simulink model "simulator_prototype"  (R2021b)
(part 11 of 12)

t6722 = ct{1511};
t6724 = ct{1512};
t6725 = ct{1513};
t6727 = ct{1514};
t6728 = ct{1515};
t6731 = ct{1516};
t6732 = ct{1517};
t6736 = ct{1518};
t6737 = ct{1519};
t6738 = ct{1520};
t6739 = ct{1521};
t674 = ct{1522};
t6740 = ct{1523};
t6742 = ct{1524};
t6743 = ct{1525};
t6744 = ct{1526};
t6745 = ct{1527};
t6746 = ct{1528};
t6747 = ct{1529};
t6750 = ct{1530};
t6751 = ct{1531};
t6754 = ct{1532};
t6756 = ct{1533};
t6757 = ct{1534};
t6758 = ct{1535};
t6760 = ct{1536};
t6762 = ct{1537};
t6763 = ct{1538};
t6764 = ct{1539};
t6765 = ct{1540};
t6766 = ct{1541};
t6767 = ct{1542};
t6768 = ct{1543};
t6769 = ct{1544};
t6770 = ct{1545};
t6771 = ct{1546};
t6772 = ct{1547};
t6773 = ct{1548};
t6774 = ct{1549};
t6775 = ct{1550};
t6776 = ct{1551};
t6778 = ct{1552};
t6779 = ct{1553};
t6780 = ct{1554};
t6781 = ct{1555};
t6782 = ct{1556};
t6783 = ct{1557};
t6784 = ct{1558};
t6785 = ct{1559};
t6786 = ct{1560};
t6787 = ct{1561};
t6788 = ct{1562};
t6789 = ct{1563};
t6791 = ct{1564};
t6792 = ct{1565};
t6793 = ct{1566};
t6795 = ct{1567};
t6796 = ct{1568};
t6797 = ct{1569};
t6798 = ct{1570};
t6799 = ct{1571};
t6800 = ct{1572};
t6803 = ct{1573};
t6804 = ct{1574};
t6808 = ct{1575};
t6810 = ct{1576};
t6813 = ct{1577};
t6814 = ct{1578};
t6816 = ct{1579};
t6817 = ct{1580};
t6819 = ct{1581};
t6820 = ct{1582};
t6821 = ct{1583};
t6822 = ct{1584};
t6823 = ct{1585};
t6824 = ct{1586};
t6825 = ct{1587};
t6826 = ct{1588};
t6827 = ct{1589};
t6828 = ct{1590};
t6831 = ct{1591};
t6833 = ct{1592};
t6836 = ct{1593};
t6838 = ct{1594};
t6839 = ct{1595};
t684 = ct{1596};
t6841 = ct{1597};
t6842 = ct{1598};
t6843 = ct{1599};
t6844 = ct{1600};
t6848 = ct{1601};
t6849 = ct{1602};
t685 = ct{1603};
t6851 = ct{1604};
t6852 = ct{1605};
t6853 = ct{1606};
t6855 = ct{1607};
t6858 = ct{1608};
t6859 = ct{1609};
t686 = ct{1610};
t6866 = ct{1611};
t6867 = ct{1612};
t6868 = ct{1613};
t687 = ct{1614};
t6870 = ct{1615};
t6872 = ct{1616};
t6873 = ct{1617};
t6875 = ct{1618};
t6877 = ct{1619};
t6878 = ct{1620};
t6879 = ct{1621};
t6880 = ct{1622};
t6882 = ct{1623};
t6883 = ct{1624};
t6884 = ct{1625};
t6885 = ct{1626};
t6886 = ct{1627};
t6887 = ct{1628};
t6888 = ct{1629};
t6889 = ct{1630};
t6894 = ct{1631};
t6897 = ct{1632};
t6900 = ct{1633};
t6902 = ct{1634};
t6903 = ct{1635};
t6904 = ct{1636};
t6908 = ct{1637};
t6909 = ct{1638};
t6910 = ct{1639};
t6911 = ct{1640};
t6912 = ct{1641};
t6913 = ct{1642};
t6916 = ct{1643};
t6918 = ct{1644};
t6919 = ct{1645};
t6920 = ct{1646};
t6924 = ct{1647};
t6925 = ct{1648};
t6929 = ct{1649};
t6931 = ct{1650};
t6932 = ct{1651};
t6933 = ct{1652};
t6941 = ct{1653};
t6942 = ct{1654};
t6945 = ct{1655};
t6949 = ct{1656};
t6950 = ct{1657};
t6951 = ct{1658};
t6959 = ct{1659};
t6962 = ct{1660};
t6964 = ct{1661};
t6965 = ct{1662};
t6966 = ct{1663};
t6968 = ct{1664};
t6971 = ct{1665};
t6972 = ct{1666};
t6975 = ct{1667};
t6976 = ct{1668};
t6979 = ct{1669};
t6983 = ct{1670};
t6985 = ct{1671};
t6987 = ct{1672};
t6989 = ct{1673};
t6992 = ct{1674};
t6993 = ct{1675};
t6994 = ct{1676};
t6995 = ct{1677};
t6996 = ct{1678};
t6997 = ct{1679};
t7000 = ct{1680};
t7001 = ct{1681};
t7003 = ct{1682};
t7005 = ct{1683};
t7007 = ct{1684};
t7009 = ct{1685};
t7010 = ct{1686};
t7011 = ct{1687};
t7012 = ct{1688};
t7014 = ct{1689};
t7016 = ct{1690};
t7019 = ct{1691};
t7020 = ct{1692};
t7022 = ct{1693};
t7023 = ct{1694};
t7024 = ct{1695};
t7025 = ct{1696};
t7026 = ct{1697};
t7028 = ct{1698};
t7029 = ct{1699};
t7030 = ct{1700};
t7031 = ct{1701};
t7032 = ct{1702};
t7033 = ct{1703};
t7034 = ct{1704};
t7035 = ct{1705};
t7036 = ct{1706};
t7037 = ct{1707};
t7038 = ct{1708};
t7039 = ct{1709};
t7040 = ct{1710};
t7041 = ct{1711};
t7042 = ct{1712};
t7043 = ct{1713};
t7047 = ct{1714};
t7048 = ct{1715};
t7049 = ct{1716};
t7051 = ct{1717};
t7052 = ct{1718};
t7055 = ct{1719};
t7057 = ct{1720};
t7059 = ct{1721};
t7060 = ct{1722};
t7061 = ct{1723};
t7062 = ct{1724};
t7063 = ct{1725};
t7064 = ct{1726};
t7066 = ct{1727};
t707 = ct{1728};
t7072 = ct{1729};
t7073 = ct{1730};
t7074 = ct{1731};
t7076 = ct{1732};
t7078 = ct{1733};
t7079 = ct{1734};
t708 = ct{1735};
t7080 = ct{1736};
t7083 = ct{1737};
t7084 = ct{1738};
t7086 = ct{1739};
t7088 = ct{1740};
t7090 = ct{1741};
t7092 = ct{1742};
t7095 = ct{1743};
t7098 = ct{1744};
t710 = ct{1745};
t7101 = ct{1746};
t7102 = ct{1747};
t7108 = ct{1748};
t7109 = ct{1749};
t7111 = ct{1750};
t7112 = ct{1751};
t7114 = ct{1752};
t7118 = ct{1753};
t7125 = ct{1754};
t7127 = ct{1755};
t7128 = ct{1756};
t7131 = ct{1757};
t7132 = ct{1758};
t7133 = ct{1759};
t7134 = ct{1760};
t7140 = ct{1761};
t7142 = ct{1762};
t7148 = ct{1763};
t7149 = ct{1764};
t7150 = ct{1765};
t7156 = ct{1766};
t7159 = ct{1767};
t7161 = ct{1768};
t7162 = ct{1769};
t7164 = ct{1770};
t7166 = ct{1771};
t7170 = ct{1772};
t7171 = ct{1773};
t7174 = ct{1774};
t7176 = ct{1775};
t7179 = ct{1776};
t7181 = ct{1777};
t7182 = ct{1778};
t7184 = ct{1779};
t7186 = ct{1780};
t7187 = ct{1781};
t7195 = ct{1782};
t7196 = ct{1783};
t7197 = ct{1784};
t7199 = ct{1785};
t7200 = ct{1786};
t7203 = ct{1787};
t7204 = ct{1788};
t7205 = ct{1789};
t7206 = ct{1790};
t7208 = ct{1791};
t721 = ct{1792};
t7211 = ct{1793};
t7213 = ct{1794};
t7215 = ct{1795};
t7216 = ct{1796};
t7217 = ct{1797};
t7218 = ct{1798};
t7219 = ct{1799};
t722 = ct{1800};
t7220 = ct{1801};
t7221 = ct{1802};
t7222 = ct{1803};
t7224 = ct{1804};
t7226 = ct{1805};
t7228 = ct{1806};
t7229 = ct{1807};
t7230 = ct{1808};
t7231 = ct{1809};
t7232 = ct{1810};
t7233 = ct{1811};
t7234 = ct{1812};
t7235 = ct{1813};
t7237 = ct{1814};
t7238 = ct{1815};
t724 = ct{1816};
t7240 = ct{1817};
t7243 = ct{1818};
t7244 = ct{1819};
t7246 = ct{1820};
t7248 = ct{1821};
t7249 = ct{1822};
t7251 = ct{1823};
t7253 = ct{1824};
t7254 = ct{1825};
t7255 = ct{1826};
t7256 = ct{1827};
t7257 = ct{1828};
t7260 = ct{1829};
t7261 = ct{1830};
t7262 = ct{1831};
t7263 = ct{1832};
t7265 = ct{1833};
t7266 = ct{1834};
t7267 = ct{1835};
t7268 = ct{1836};
t7269 = ct{1837};
t7271 = ct{1838};
t7272 = ct{1839};
t7273 = ct{1840};
t7274 = ct{1841};
t7275 = ct{1842};
t7277 = ct{1843};
t7279 = ct{1844};
t7281 = ct{1845};
t7283 = ct{1846};
t7292 = ct{1847};
t7294 = ct{1848};
t7295 = ct{1849};
t7298 = ct{1850};
t7300 = ct{1851};
t7301 = ct{1852};
t7302 = ct{1853};
t7303 = ct{1854};
t7304 = ct{1855};
t7307 = ct{1856};
t7310 = ct{1857};
t7311 = ct{1858};
t7312 = ct{1859};
t7315 = ct{1860};
t7316 = ct{1861};
t7319 = ct{1862};
t7323 = ct{1863};
t7324 = ct{1864};
t7326 = ct{1865};
t7327 = ct{1866};
t7328 = ct{1867};
t7329 = ct{1868};
t7335 = ct{1869};
t7336 = ct{1870};
t7337 = ct{1871};
t7342 = ct{1872};
t7343 = ct{1873};
t7344 = ct{1874};
t7345 = ct{1875};
t7346 = ct{1876};
t7347 = ct{1877};
t7349 = ct{1878};
t7351 = ct{1879};
t7352 = ct{1880};
t7353 = ct{1881};
t7354 = ct{1882};
t7355 = ct{1883};
t7356 = ct{1884};
t7358 = ct{1885};
t7359 = ct{1886};
t7360 = ct{1887};
t7363 = ct{1888};
t7364 = ct{1889};
t7367 = ct{1890};
t7368 = ct{1891};
t7369 = ct{1892};
t7370 = ct{1893};
t7378 = ct{1894};
t7379 = ct{1895};
t7380 = ct{1896};
t7385 = ct{1897};
t7387 = ct{1898};
t7388 = ct{1899};
t7390 = ct{1900};
t7391 = ct{1901};
t7392 = ct{1902};
t7393 = ct{1903};
t7394 = ct{1904};
t7396 = ct{1905};
t7397 = ct{1906};
t7398 = ct{1907};
t7399 = ct{1908};
t7401 = ct{1909};
t7402 = ct{1910};
t7404 = ct{1911};
t7405 = ct{1912};
t7406 = ct{1913};
t7407 = ct{1914};
t7408 = ct{1915};
t7409 = ct{1916};
t7410 = ct{1917};
t7411 = ct{1918};
t7412 = ct{1919};
t7413 = ct{1920};
t7414 = ct{1921};
t7415 = ct{1922};
t7416 = ct{1923};
t7417 = ct{1924};
t7419 = ct{1925};
t7420 = ct{1926};
t7421 = ct{1927};
t7424 = ct{1928};
t7425 = ct{1929};
t7432 = ct{1930};
t7433 = ct{1931};
t7436 = ct{1932};
t7439 = ct{1933};
t7441 = ct{1934};
t7443 = ct{1935};
t7444 = ct{1936};
t7446 = ct{1937};
t7447 = ct{1938};
t7448 = ct{1939};
t7450 = ct{1940};
t7451 = ct{1941};
t7453 = ct{1942};
t7454 = ct{1943};
t7456 = ct{1944};
t7458 = ct{1945};
t7462 = ct{1946};
t7463 = ct{1947};
t7469 = ct{1948};
t7470 = ct{1949};
t7472 = ct{1950};
t7473 = ct{1951};
t7479 = ct{1952};
t7480 = ct{1953};
t7482 = ct{1954};
t7483 = ct{1955};
t7487 = ct{1956};
t7489 = ct{1957};
t749 = ct{1958};
t7490 = ct{1959};
t7491 = ct{1960};
t7493 = ct{1961};
t7494 = ct{1962};
t7501 = ct{1963};
t7511 = ct{1964};
t7512 = ct{1965};
t7514 = ct{1966};
t7518 = ct{1967};
t7519 = ct{1968};
t7523 = ct{1969};
t7524 = ct{1970};
t7525 = ct{1971};
t7526 = ct{1972};
t7532 = ct{1973};
t7534 = ct{1974};
t7535 = ct{1975};
t7537 = ct{1976};
t7538 = ct{1977};
t7544 = ct{1978};
t7548 = ct{1979};
t7553 = ct{1980};
t7554 = ct{1981};
t7560 = ct{1982};
t7561 = ct{1983};
t7562 = ct{1984};
t7596 = ct{1985};
t7599 = ct{1986};
t7601 = ct{1987};
t7607 = ct{1988};
t7609 = ct{1989};
t7610 = ct{1990};
t7611 = ct{1991};
t7612 = ct{1992};
t7613 = ct{1993};
t7614 = ct{1994};
t7615 = ct{1995};
t762 = ct{1996};
t7624 = ct{1997};
t7626 = ct{1998};
t7630 = ct{1999};
t7631 = ct{2000};
t7638 = ct{2001};
t7639 = ct{2002};
t7641 = ct{2003};
t7652 = ct{2004};
t7654 = ct{2005};
t7655 = ct{2006};
t7656 = ct{2007};
t7658 = ct{2008};
t7662 = ct{2009};
t7663 = ct{2010};
t7664 = ct{2011};
t7665 = ct{2012};
t7668 = ct{2013};
t7670 = ct{2014};
t7672 = ct{2015};
t7675 = ct{2016};
t7676 = ct{2017};
t7677 = ct{2018};
t768 = ct{2019};
t7682 = ct{2020};
t7683 = ct{2021};
t7686 = ct{2022};
t7688 = ct{2023};
t7690 = ct{2024};
t7691 = ct{2025};
t7692 = ct{2026};
t7695 = ct{2027};
t7696 = ct{2028};
t7697 = ct{2029};
t7704 = ct{2030};
t7707 = ct{2031};
t7710 = ct{2032};
t7711 = ct{2033};
t7712 = ct{2034};
t7713 = ct{2035};
t7715 = ct{2036};
t7716 = ct{2037};
t7724 = ct{2038};
t7725 = ct{2039};
t7727 = ct{2040};
t7730 = ct{2041};
t7736 = ct{2042};
t7737 = ct{2043};
t7738 = ct{2044};
t7746 = ct{2045};
t7752 = ct{2046};
t7753 = ct{2047};
t7756 = ct{2048};
t7763 = ct{2049};
t777 = ct{2050};
t7773 = ct{2051};
t7784 = ct{2052};
t7789 = ct{2053};
t7790 = ct{2054};
t7791 = ct{2055};
t7792 = ct{2056};
t7796 = ct{2057};
t7798 = ct{2058};
t7804 = ct{2059};
t7805 = ct{2060};
t7807 = ct{2061};
t7808 = ct{2062};
t7809 = ct{2063};
t7811 = ct{2064};
t7814 = ct{2065};
t7815 = ct{2066};
t7816 = ct{2067};
t7817 = ct{2068};
t7820 = ct{2069};
t7822 = ct{2070};
t7823 = ct{2071};
t7824 = ct{2072};
t7826 = ct{2073};
t7827 = ct{2074};
t7828 = ct{2075};
t7830 = ct{2076};
t7835 = ct{2077};
t7836 = ct{2078};
t7838 = ct{2079};
t7839 = ct{2080};
t7840 = ct{2081};
t7841 = ct{2082};
t7842 = ct{2083};
t7845 = ct{2084};
t7847 = ct{2085};
t7848 = ct{2086};
t7850 = ct{2087};
t7859 = ct{2088};
t7860 = ct{2089};
t7868 = ct{2090};
t7869 = ct{2091};
t7880 = ct{2092};
t7885 = ct{2093};
t7888 = ct{2094};
t7891 = ct{2095};
t7894 = ct{2096};
t7895 = ct{2097};
t7897 = ct{2098};
t7900 = ct{2099};
t7902 = ct{2100};
t7909 = ct{2101};
t7919 = ct{2102};
t792 = ct{2103};
t7920 = ct{2104};
t7921 = ct{2105};
t7922 = ct{2106};
t7923 = ct{2107};
t7924 = ct{2108};
t7925 = ct{2109};
t7926 = ct{2110};
t793 = ct{2111};
t7938 = ct{2112};
t7939 = ct{2113};
t7940 = ct{2114};
t7948 = ct{2115};
t7949 = ct{2116};
t7951 = ct{2117};
t7952 = ct{2118};
t7953 = ct{2119};
t7955 = ct{2120};
t7957 = ct{2121};
t7965 = ct{2122};
t7966 = ct{2123};
t7975 = ct{2124};
t7976 = ct{2125};
t8 = ct{2126};
t801 = ct{2127};
t802 = ct{2128};
t808 = ct{2129};
t813 = ct{2130};
t819 = ct{2131};
t821 = ct{2132};
t850 = ct{2133};
t855 = ct{2134};
t874 = ct{2135};
t878 = ct{2136};
t9 = ct{2137};
t941 = ct{2138};
t948 = ct{2139};
t951 = ct{2140};
t7372 = t7369./2.0;
t7426 = t5486+t6634+t6638;
t7440 = -t7439;
t7442 = -t7441;
t7449 = t5579+t6772+t6780;
t7461 = t5682+t6817+t6819;
t7495 = -t7494;
t7496 = (t3915.*t7469)./2.0;
t7497 = t7470.*(-t1901+t3122+t3277).*(-1.0./2.0);
t7498 = (t3976.*t7469)./2.0;
t7502 = (t4001.*t7470)./2.0;
t7505 = t5082+t5356+t6395+t7203;
t7506 = t6793.*(t4844+t5119-t5723-t6364).*(-1.0./2.0);
t7507 = (t6793.*(t4844+t5119-t5723-t6364))./2.0;
t7508 = (t4118.*t7469)./2.0;
t7510 = t7470.*(t951+t10.*(-t1881+t3121+t3276)).*(-1.0./2.0);
t7515 = t6711.*(t4927+t5198-t5762-t6392).*(-1.0./2.0);
t7516 = (t6711.*(t4927+t5198-t5762-t6392))./2.0;
t7529 = (t4838.*t7469)./2.0;
t7530 = t7470.*(t11.*((t237.*(t42-t43))./9.007199254740992e+15+t15.*(-t1881+t3121+t3276))+t16.*(-t1901+t3122+t3277)).*(-1.0./2.0);
t7541 = (t3500.*t7523)./2.0;
t7543 = t11.*t7523.*(t1861-t3221).*(-1.0./2.0);
t7545 = (t3503.*t7524)./2.0;
t7546 = (t11.*t3502.*t7524)./2.0;
t7549 = (t3915.*t7523)./2.0;
t7551 = t7524.*(-t1901+t3122+t3277).*(-1.0./2.0);
t7552 = (t7524.*(-t1901+t3122+t3277))./2.0;
t7557 = (t4118.*t7523)./2.0;
t7558 = t7524.*(t951+t10.*(-t1881+t3121+t3276)).*(-1.0./2.0);
t7559 = (t7524.*(t951+t10.*(-t1881+t3121+t3276)))./2.0;
t7563 = (t3500.*t7544)./2.0;
t7564 = t11.*t7544.*(t1861-t3221).*(-1.0./2.0);
t7565 = (t3503.*t7548)./2.0;
t7566 = (t11.*t3502.*t7548)./2.0;
t7575 = (t3976.*t7544)./2.0;
t7577 = (t4001.*t7548)./2.0;
t7579 = (t4838.*t7523)./2.0;
t7580 = t7524.*(t11.*((t237.*(t42-t43))./9.007199254740992e+15+t15.*(-t1881+t3121+t3276))+t16.*(-t1901+t3122+t3277)).*(-1.0./2.0);
t7581 = t5844+t7072+t7074;
t7602 = (t5958.*t7463)./2.0;
t7604 = (t5962.*t7463)./2.0;
t7616 = (t5958.*t7480)./2.0;
t7618 = (t5962.*t7480)./2.0;
t7632 = (t3500.*t7630)./2.0;
t7634 = t11.*t7630.*(t1861-t3221).*(-1.0./2.0);
t7635 = (t3503.*t7631)./2.0;
t7636 = (t11.*t3502.*t7631)./2.0;
t7645 = (t3915.*t7630)./2.0;
t7646 = t7631.*(-t1901+t3122+t3277).*(-1.0./2.0);
t7647 = (t3976.*t7630)./2.0;
t7648 = (t4001.*t7631)./2.0;
t7649 = (t4118.*t7630)./2.0;
t7651 = t7631.*(t951+t10.*(-t1881+t3121+t3276)).*(-1.0./2.0);
t7657 = -t7656;
t7660 = (t4838.*t7630)./2.0;
t7661 = t7631.*(t11.*((t237.*(t42-t43))./9.007199254740992e+15+t15.*(-t1881+t3121+t3276))+t16.*(-t1901+t3122+t3277)).*(-1.0./2.0);
t7669 = (t6689.*t7463)./2.0;
t7671 = t6650.*(t5034-t5280-t6302+t7166).*(-1.0./2.0);
t7673 = (t6793.*t7463)./2.0;
t7678 = t6711.*(t5034-t5280-t6302+t7166).*(-1.0./2.0);
t7679 = (t6711.*(t5034-t5280-t6302+t7166))./2.0;
t7680 = (t6689.*t7480)./2.0;
t7687 = (t6793.*t7480)./2.0;
t7709 = t5234+t5453+t6369+t6372+t6616+t6618;
t7714 = t6773+t6774+t6775+t6784;
t7720 = t6813+t6814+t6816+t6823;
t7726 = t6842+t6843+t6844+t6849;
t7728 = t6848+t6851+t6853+t6855;
t7729 = -t7727;
t7731 = -t7730;
t7734 = t3217.*(-t6848+t6852+t6584.*(t3563-t4051)+t6585.*(t3563-t4051)).*(-1.0./2.0);
t7741 = t3502.*(-t6848+t6852+t6584.*(t3563-t4051)+t6585.*(t3563-t4051)).*(-1.0./2.0);
t7745 = t3910.*(-t6848+t6852+t6584.*(t3563-t4051)+t6585.*(t3563-t4051)).*(-1.0./2.0);
t7748 = t5410+t5564+t6547+t6548+t6758+t6763;
t7749 = t5412+t5563+t6550+t6551+t6764+t6765;
t7751 = (t3216.*t7746)./2.0;
t7755 = t6929+t6931+t6932+t6933;
t7758 = t5419+t5641+t6552+t6556+t6791+t6796;
t7761 = t7746.*(t2674-t2676+t3022-t3027).*(-1.0./2.0);
t7762 = (t7746.*(t2674-t2676+t3022-t3027))./2.0;
t7766 = (t3980.*t7746)./2.0;
t7769 = (t3217.*t7756)./2.0;
t7771 = (t3502.*t7756)./2.0;
t7772 = t6945+t6949+t6950+t6951;
t7775 = (t3910.*t7756)./2.0;
t7779 = (t3217.*t7773)./2.0;
t7782 = (t3502.*t7773)./2.0;
t7788 = (t3910.*t7773)./2.0;
t7793 = -t7792;
t7795 = t5798+t5802+t6561+t6562+t6866+t6867;
t7799 = t5636+t5772+t6683+t6684+t6908+t6909;
t7800 = t5638+t5774+t6685+t6686+t6910+t6912;
t7802 = (t3217.*t7798)./2.0;
t7810 = (t3910.*t7798)./2.0;
t7813 = (t3991.*t7798)./2.0;
t7825 = t7181+t7184+t7186+t7187;
t7831 = t5553+t6111+t6740+t6743+t7324+t7327;
t7843 = t5695+t6262+t6885+t6886+t7353+t7354;
t7844 = t5694+t6266+t6887+t6889+t7355+t7356;
t7846 = -t7845;
t7849 = -t7848;
t7854 = t2297.*(t5816-t6360-t7032+t7033+t7367-t7369).*(-1.0./2.0);
t7855 = t3047.*(t5816-t6360-t7032+t7033+t7367-t7369).*(-1.0./2.0);
t7856 = t6074+t6941+t6942+t7073+t7076+t7078+t7079;
t7861 = -t7860;
t7862 = t5875+t6481+t7128+t7131+t7390+t7391;
t7863 = t5874+t6480+t7132+t7133+t7392+t7393;
t7875 = t5467+t6626+t6627+t6663+t7490+t7493;
t7881 = t3129+t3200+t3201+t3208+t3468+t3482+t3488+t3590+t3817+t3818+t3890+t3896+t4208+t4339+t4341+t4415+t4416+t5589+t5593+t5720+t5724+t5907+t5914+t6008+t6015+t6447+t6453+t6503+t6507;
t7883 = t5945+t6750+t7108+t7109+t7424+t7425;
t7896 = (t3217.*t7894)./2.0;
t7898 = (t3502.*t7894)./2.0;
t7901 = -t7900;
t7903 = t5573+t6754+t6756+t6804+t7534+t7535;
t7908 = t5890+t6810+t7047+t7049+t7525+t7526;
t7911 = (t3217.*t7909)./2.0;
t7914 = (t3502.*t7909)./2.0;
t7918 = (t3991.*t7909)./2.0;
t7927 = (t3216.*t7925)./2.0;
t7928 = (t3217.*t7926)./2.0;
t7930 = t7925.*(t1861-t3221).*(-1.0./2.0);
t7931 = (t7925.*(t1861-t3221))./2.0;
t7932 = (t3502.*t7926)./2.0;
t7934 = (t3980.*t7925)./2.0;
t7936 = (t3991.*t7926)./2.0;
t7937 = t2990+t2991+t3057+t3058+t4828+t4833+t4895+t4902+t5919+t5922+t5930+t5933+t6316+t6319+t6354+t6357+t6836+t6838+t6839+t6841;
t7941 = t5826+t7060+t7061+t7195+t7652+t7655;
t7950 = t6110+t7213+t7238+t7240+t7664+t7665;
t7954 = (t3217.*t7951)./2.0;
t7956 = (t3502.*t7951)./2.0;
t7958 = (t3991.*t7951)./2.0;
t6277 = t3934.*t5848.*(t1513+t1879+t2598+t2820+t2834+t3117+t3118).*(-3.633675e-3);
t6278 = t3934.*t5848.*(t1513+t1879+t2598+t2820+t2834+t3117+t3118).*3.633675e-3;
t6644 = -t6643;
t6834 = (t5848.*t5958)./2.0;
t6835 = (t5848.*t5962)./2.0;
t6960 = -t6959;
t7013 = -t7012;
t7027 = -t7026;
t7085 = -t7084;
t7103 = -t7102;
t7113 = -t7112;
t7115 = -t7114;
t7143 = -t7142;
t7157 = -t7156;
t7175 = -t7174;
t7177 = -t7176;
t7180 = -t7179;
t7202 = -t7200;
t7207 = -t7206;
t7242 = (t5848.*t6689)./2.0;
t7245 = -t7244;
t7250 = -t7249;
t7258 = -t7257;
t7264 = (t5848.*t6793)./2.0;
t7270 = -t7269;
t7276 = -t7275;
t7371 = -t7370;
t7373 = -t7372;
t7427 = t188.*t7426.*4.297799892626299e-1;
t7428 = (t2338.*t7426)./2.0;
t7429 = (t2994.*t7426)./2.0;
t7431 = t7426.*(t1456-t2355).*(-1.0./2.0);
t7464 = (t2307.*t7461)./2.0;
t7466 = (t11.*t2297.*t7461)./2.0;
t7467 = t7461.*(t1456-t2355).*(-1.0./2.0);
t7499 = -t7498;
t7503 = -t7502;
t7509 = -t7508;
t7542 = -t7541;
t7547 = -t7546;
t7550 = -t7549;
t7567 = -t7565;
t7568 = -t7566;
t7576 = -t7575;
t7578 = -t7577;
t7582 = t188.*t7581.*4.297799892626299e-1;
t7584 = (t2307.*t7581)./2.0;
t7585 = (t11.*t2297.*t7581)./2.0;
t7586 = (t2338.*t7581)./2.0;
t7587 = (t2994.*t7581)./2.0;
t7588 = t7581.*(t1456-t2355).*(-1.0./2.0);
t7589 = (t7581.*(t1456-t2355))./2.0;
t7603 = -t7602;
t7605 = -t7604;
t7617 = -t7616;
t7619 = -t7618;
t7628 = (t5859.*t7505)./2.0;
t7629 = (t5860.*t7505)./2.0;
t7633 = -t7632;
t7650 = -t7649;
t7674 = -t7673;
t7684 = (t6650.*t7505)./2.0;
t7693 = (t6711.*t7505)./2.0;
t7698 = t6632+t6633+t6636+t6637;
t7717 = t50.*t189.*t7714.*4.771516396025243e-17;
t7719 = (t2297.*t7714)./2.0;
t7721 = t50.*t189.*t7720.*4.771516396025243e-17;
t7722 = (t2297.*t7720)./2.0;
t7732 = (t3216.*t7726)./2.0;
t7739 = t7726.*(t1861-t3221).*(-1.0./2.0);
t7740 = (t7726.*(t1861-t3221))./2.0;
t7743 = t7726.*(t2674-t2676+t3022-t3027).*(-1.0./2.0);
t7744 = (t7726.*(t2674-t2676+t3022-t3027))./2.0;
t7759 = (t2297.*t7758)./2.0;
t7764 = (t3047.*t7758)./2.0;
t7768 = (t3216.*t7755)./2.0;
t7770 = t7755.*(t1861-t3221).*(-1.0./2.0);
t7774 = t7755.*(t2674-t2676+t3022-t3027).*(-1.0./2.0);
t7776 = -t7775;
t7777 = (t3216.*t7772)./2.0;
t7780 = -t7779;
t7781 = t7772.*(t1861-t3221).*(-1.0./2.0);
t7783 = -t7782;
t7786 = t7772.*(t2674-t2676+t3022-t3027).*(-1.0./2.0);
t7787 = (t7772.*(t2674-t2676+t3022-t3027))./2.0;
t7803 = -t7802;
t7806 = t7799.*(t1861-t3221).*(-1.0./2.0);
t7818 = t7799.*(t2674-t2676+t3022-t3027).*(-1.0./2.0);
t7819 = (t7799.*(t2674-t2676+t3022-t3027))./2.0;
t7821 = (t3980.*t7799)./2.0;
t7832 = (t2297.*t7831)./2.0;
t7833 = (t3047.*t7831)./2.0;
t7853 = t5817+t6360+t7032+t7036+t7368+t7369;
t7857 = t34.*t7856;
t7864 = t7862.*(t1861-t3221).*(-1.0./2.0);
t7865 = (t3502.*t7863)./2.0;
t7870 = t7862.*(t2674-t2676+t3022-t3027).*(-1.0./2.0);
t7871 = (t3910.*t7863)./2.0;
t7873 = (t3980.*t7862)./2.0;
t7874 = (t3991.*t7863)./2.0;
t7876 = t50.*t189.*t7875.*4.771516396025243e-17;
t7877 = (t2297.*t7875)./2.0;
t7878 = (t3047.*t7875)./2.0;
t7886 = (t3217.*t7883)./2.0;
t7889 = (t3910.*t7883)./2.0;
t7892 = (t3991.*t7883)./2.0;
t7904 = t50.*t189.*t7903.*4.771516396025243e-17;
t7906 = (t2297.*t7903)./2.0;
t7907 = (t3047.*t7903)./2.0;
t7910 = (t3216.*t7908)./2.0;
t7912 = t7908.*(t1861-t3221).*(-1.0./2.0);
t7913 = (t7908.*(t1861-t3221))./2.0;
t7917 = (t3980.*t7908)./2.0;
t7929 = -t7928;
t7933 = -t7932;
t7935 = -t7934;
t7942 = t50.*t189.*t7941.*4.771516396025243e-17;
t7944 = (t2297.*t7941)./2.0;
t7945 = (t3047.*t7941)./2.0;
t7969 = t5846+t6625+t6731+t6737+t6781+t6782+t6785+t6786+t7024+t7025+t7204+t7206+t7396+t7399;
t7970 = t5846+t6625+t6732+t6739+t6781+t6782+t6785+t6786+t7024+t7025+t7204+t7206+t7396+t7399;
t7971 = t5827+t5967+t5969+t6206+t6209+t6822+t6824+t6826+t6827+t7062+t7063+t7196+t7654+t7657;
t7972 = t5827+t5967+t5969+t6208+t6210+t6822+t6824+t6826+t6827+t7062+t7063+t7196+t7654+t7657;
t7987 = t5105+t5246+t5248+t5374+t5383+t5386+t5390+t5422+t5468+t5556+t5558+t5614+t5624+t5642+t5725+t5753+t5867+t5870+t5891+t5893+t5988+t6022+t6055+t6080+t6125+t6141+t6185+t6188+t6200+t6418+t6555+t6557+t6569+t6571+t6575+t6608+t6628+t6629+t6664+t6797+t6798+t6883+t7095+t7098+t7148+t7150+t7279+t7342+t7343+t7349+t7472+t7491+t7495+t7607+t7610;
t7988 = t5105+t5246+t5248+t5374+t5383+t5386+t5390+t5422+t5468+t5556+t5558+t5616+t5632+t5642+t5725+t5753+t5868+t5872+t5891+t5893+t5988+t6022+t6055+t6080+t6125+t6141+t6187+t6189+t6200+t6418+t6555+t6557+t6570+t6572+t6575+t6608+t6628+t6629+t6664+t6797+t6798+t6883+t7095+t7098+t7148+t7150+t7279+t7342+t7343+t7349+t7472+t7491+t7495+t7609+t7611;
t7430 = -t7429;
t7465 = -t7464;
t7583 = -t7582;
t7694 = -t7693;
t7699 = t50.*t189.*t7698.*4.771516396025243e-17;
t7700 = (t2297.*t7698)./2.0;
t7718 = -t7717;
t7723 = -t7722;
t7760 = -t7759;
t7765 = -t7764;
t7778 = -t7777;
t7834 = -t7833;
t7866 = -t7865;
t7872 = -t7871;
t7879 = -t7878;
t7887 = -t7886;
t7890 = -t7889;
t7905 = -t7904;
t7943 = -t7942;
t7959 = t5567+t6050+t6119+t6219+t6226+t6788+t6792+t6878+t6880+t7057+t7064+t7140+t7143;
t7960 = t5567+t6050+t6119+t6219+t6226+t6789+t6799+t6878+t6880+t7057+t7064+t7140+t7143;
t7961 = t5612+t6062+t6094+t6324+t6343+t6831+t6834+t6894+t6900+t7041+t7048+t7197+t7200;
t7962 = t5612+t6062+t6094+t6324+t6343+t6833+t6835+t6894+t6900+t7041+t7048+t7197+t7200;
t7963 = t3416+t3765+t3766+t4030+t4039+t4041+t4270+t4272+t4318+t4372+t4373+t5997+t6000+t6045+t6047+t6455+t6458+t6520+t6522+t7265+t7266+t7268+t7270;
t7964 = t3416+t3765+t3766+t4030+t4039+t4041+t4270+t4272+t4318+t4372+t4373+t5999+t6001+t6043+t6046+t6457+t6459+t6519+t6521+t7271+t7272+t7274+t7276;
t7967 = t5820+t6361+t6635+t6641+t6642+t6644+t6692+t6694+t7034+t7039+t7149+t7157+t7371+t7372;
t7968 = t5820+t6361+t6635+t6641+t6642+t6644+t6693+t6695+t7034+t7039+t7149+t7157+t7371+t7372;
t7973 = t3129+t3200+t3201+t3208+t3468+t3482+t3488+t3590+t3817+t3818+t3890+t3896+t4208+t4339+t4341+t4415+t4416+t5589+t5593+t5717+t5722+t5907+t5914+t6006+t6010+t6447+t6453+t6501+t6505+t6671+t6672+t6688+t6691+t7255+t7258+t7262+t7263;
t7974 = t3129+t3200+t3201+t3208+t3468+t3482+t3488+t3590+t3817+t3818+t3890+t3896+t4208+t4339+t4341+t4415+t4416+t5587+t5592+t5720+t5724+t5905+t5910+t6008+t6015+t6445+t6450+t6503+t6507+t6858+t6859+t6868+t6870+t7243+t7245+t7248+t7251;
t7977 = t5343+t5565+t5813+t5851+t5877+t5880+t6067+t6096+t6173+t6180+t6217+t6225+t6425+t6438+t6461+t6469+t6483+t6484+t6701+t6707+t6962+t6964+t6994+t6996+t7111+t7115+t7159+t7161+t7416+t7419;
t7978 = t5343+t5565+t5813+t5851+t5877+t5880+t6067+t6096+t6175+t6183+t6217+t6225+t6425+t6438+t6461+t6469+t6483+t6484+t6703+t6709+t6962+t6964+t6994+t6996+t7111+t7115+t7159+t7161+t7417+t7421;
t7979 = t5344+t5568+t5680+t5690+t5924+t5926+t5966+t5974+t5977+t5981+t5982+t6241+t6290+t6296+t6366+t6368+t6527+t6539+t7029+t7030+t7035+t7040+t7301+t7303+t7360+t7363+t7613+t7617;
t7980 = t5344+t5568+t5680+t5690+t5924+t5926+t5966+t5975+t5979+t5981+t5982+t6241+t6292+t6300+t6366+t6368+t6527+t6539+t7029+t7030+t7035+t7040+t7301+t7303+t7360+t7363+t7615+t7619;
t7981 = t5430+t5496+t5497+t5554+t6087+t6112+t6152+t6153+t6157+t6192+t6195+t6231+t6238+t6284+t6582+t6595+t6601+t6612+t6614+t6645+t6648+t6705+t6742+t6746+t6976+t7118+t7125+t7127+t7171+t7177+t7323+t7326+t7329+t7411+t7414;
t7982 = t5430+t5496+t5497+t5554+t6087+t6112+t6152+t6153+t6157+t6192+t6195+t6233+t6240+t6284+t6582+t6595+t6601+t6612+t6614+t6646+t6649+t6705+t6742+t6746+t6976+t7118+t7125+t7127+t7171+t7177+t7323+t7326+t7329+t7413+t7415;
t7983 = t4489+t5251+t5256+t5258+t5306+t5449+t5451+t5549+t5576+t5577+t5764+t5768+t5836+t5839+t5908+t5913+t5928+t5931+t5937+t5950+t5957+t6143+t6144+t6227+t6304+t6307+t6309+t6311+t6512+t6514+t6524+t6525+t7003+t7005+t7007+t7009+t7042+t7052+t7294+t7295+t7351+t7352+t7599+t7603;
t7984 = t4489+t5251+t5256+t5258+t5306+t5449+t5451+t5549+t5576+t5577+t5766+t5770+t5836+t5839+t5908+t5913+t5928+t5931+t5937+t5951+t5960+t6143+t6144+t6227+t6307+t6308+t6311+t6312+t6513+t6517+t6524+t6525+t7003+t7005+t7007+t7009+t7042+t7052+t7294+t7295+t7351+t7352+t7601+t7605;
t7985 = t5574+t5626+t5650+t5652+t5685+t5687+t5878+t5882+t5898+t5899+t6088+t6169+t6179+t6314+t6432+t6435+t6436+t6466+t6467+t6717+t6757+t6760+t6768+t6769+t6808+t6904+t7298+t7358+t7359+t7378+t7532+t7537+t7538+t7624+t7628;
t7986 = t5574+t5626+t5650+t5652+t5685+t5687+t5879+t5884+t5898+t5899+t6088+t6170+t6182+t6314+t6432+t6435+t6436+t6466+t6467+t6717+t6757+t6760+t6768+t6769+t6808+t6904+t7298+t7358+t7359+t7378+t7532+t7537+t7538+t7626+t7629;
t7701 = -t7700;
et303 = (t5465.*(t350+t366-t1205+t1210-t1217-t1218-t2147+t2152+t2154+t2155-t3405-t3409-t3420-t3739+t3746+t26.*t50.*t202.*(t46-t47).*8.687615694748404e-39))./2.0;
et304 = t5480.*(t350+t366-t1205+t1210-t1217-t1218-t2147+t2152+t2154+t2155-t3405-t3409-t3420-t3739+t3746+t26.*t50.*t202.*(t46-t47).*8.687615694748404e-39).*(-1.0./2.0)+(t3879.*t4147)./2.0+(t3876.*t4154)./2.0-(t3877.*t4153)./2.0-(t3898.*t4147)./2.0+(t3877.*t4313)./2.0+(t5142.*t5362)./2.0;
et305 = (t5205.*t5305)./2.0-(t5200.*t5362)./2.0-(t5205.*t5358)./2.0+(t5483.*t5603)./2.0+(t5466.*t5646)./2.0-(t5483.*t5647)./2.0-(t5491.*t5646)./2.0-(t5860.*t5904)./2.0+(t5858.*t5911)./2.0+(t5856.*t5949)./2.0+(t5860.*t5946)./2.0-(t5859.*t5949)./2.0-(t5858.*t5958)./2.0-(t5855.*t5962)./2.0+(t5857.*t5962)./2.0+(t3878.*(t1089-t1104-t1105-t1121-t2117+t2120+t2122+t2123))./2.0-(t3897.*(t1089-t1104-t1105-t1121-t2117+t2120+t2122+t2123))./2.0+(t5594.*(t410-t5466))./2.0-(t5645.*(t410-t5466))./2.0-(t5359.*(t649+t670+t686+t687+t1577+t1578+t1586+t1600+t2303+t2339+t2689+t3030+t3299+t3312))./2.0;
et306 = t5201.*(t1196+t1212+t1237+t1238+t2139+t2140+t2159+t2165+t2754+t2814+t2953+t3072+t3415+t3423).*(-1.0./2.0)+(t3876.*(t313-t314-t1108+t1115-t1158-t1159-t2117+t2120+t2122+t2123))./2.0+(t5359.*(-t56+t60+t649+t670+t686+t687+t1577+t1578+t1586+t1600+t2303+t2339+t2689+t3030+t3299+t3312))./2.0+(t5201.*(-t321+t332+t1196+t1212+t1237+t1238+t2139+t2140+t2159+t2165+t2754+t2814+t2953+t3072+t3415+t3423))./2.0;
et307 = -t5547-t5584-t5585-t5825+t6076+t6341-t6346+t6377+t6379./2.0+t6491+t6493+t6727+t6728+t6985+t7162+t7174+t7179;
et308 = t5857.*(t4371.*(t1896-t3239).*7.26735e-3+t2363.*(t3328+t3344+t3642-t3658+t22.*(t3242-t3554).*1.838876e-2+t28.*(t3242-t3554).*9.99471e-3).*7.26735e-3).*(-1.0./2.0);
et309 = (t5313.*(t4853.*(t1896-t3239).*7.26735e-3+t2363.*(t684+t685-t710+t724+t1686-t1690+t1700+t1701+t2371+t2698+t2707-t2716+t2719+t3329-t3337-t3351-t3641+t3643+t3655-t3659+t4114+t4115).*7.26735e-3))./2.0-(t5859.*t6064)./2.0-(t5946.*t6039)./2.0-(t5958.*t6041)./2.0+(t6681.*(t1477-t2502))./2.0+(t6913.*(t1861-t3221))./2.0;
et310 = (t3055.*(t3435-t3448+t4615+t4619+t3976.*(t1896-t3239).*5.7e-7+t3980.*(t1896-t3239).*4.0e-8))./2.0;
et311 = t4746-t5085+t5091-t5214+t4920.*(t1861-t3221).*7.83e-6+t3934.*(t951+t10.*(-t1881+t3121+t3276)).*7.83e-6+t4118.*(t2694-t2701+t3036-t3043).*7.83e-6;
et312 = t3934.*(-t1901+t3122+t3277).*3.24e-6;
et313 = -t2306-t2317+t3145+t3148+t35.*t941.*t948.*(t850-t874).*3.775747223193135e-1;
et314 = t36.*t941.*t948.*(t850-t874).*2.244797987218524e-1;
et315 = -t2306-t2317+t3145+t3148+t35.*t941.*t948.*(t850-t874).*3.775747223193135e-1;
et316 = t36.*t941.*t948.*(t850-t874).*2.244797987218524e-1;
et317 = -t2306-t2317+t3145+t3148+t35.*t941.*t948.*(t850-t874).*3.775747223193135e-1;
et318 = t36.*t941.*t948.*(t850-t874).*2.244797987218524e-1;
et319 = -t2748-t2749+t2773+t2781-t2788+t3211+t3471+t4032-t4047+t262.*(t46-t47).*2.075672598245148e-23;
et320 = t264.*(t46-t47).*1.875105520197095e-20;
et321 = t50.*t202.*(t4757-t5088-t5090+t5097-t5098+t3913.*(t2694-t2701+t3036-t3043).*1.6e-7+t3934.*(-t1881+t3121+t3276).*1.6e-7+t3934.*(-t1901+t3122+t3277).*5.0e-8);
et322 = 2.836813422250052e-17;
et323 = -t2306-t2317+t3145+t3148+t35.*t941.*t948.*(t850-t874).*3.775747223193135e-1;
et324 = t36.*t941.*t948.*(t850-t874).*2.244797987218524e-1;
et325 = t5038+t5387-t5415-t5416-t5673+t5779-t5781+t5784-t5896-t5938+t5941+t5990-t6019+t6024-t6115+t6116+t6202-t6271-t6272+t6398+t6423-t6440-t6442+t6515-t6518+t6602-t6803+t6897-t6965+t6966+t7014+t7016+t7055+t7086+t7090+t7304-t7311-t7312+t7319+t7385./2.0+t7436+t7596+t7641./2.0;
et326 = (t201.*(t4213+t5016+t123.*t188.*(t2694-t2701+t3036-t3043).*2.442490654175345e-23+t50.*t189.*t4915.*(t42-t43).*2.711709361697228e-39))./2.0;
et327 = (t3395.*(t5508-t5515+t5598+t5599-t5605-t5611+t4920.*(t3985+t12.*(t1861-t3221)).*9.3e-7+t4915.*(t3512-t4006).*9.0e-8))./2.0+(t2363.*(et311+et312))./2.0+(t6696.*(t2527-t3009))./2.0+(t5141.*(et313+et314))./2.0;
et328 = t3934.*t4215.*(t1554+t2361+t2362+t2367+t2414+t3961+t3968+t4198+t4201+t11.*(-t1901+t3122+t3277).*5.68686e-3).*5.43845e-3+t3517.*t5200.*(t2694-t2701+t3036-t3043).*1.444822e-2+(t3499.*t5358.*(t2674-t2676+t3022-t3027))./2.0;
et329 = t3649.*t5560.*(t2694-t2701+t3036-t3043).*1.444822e-2+t3943.*t5480.*(t2694-t2701+t3036-t3043).*5.43845e-3+(t3924.*t5645.*(t2674-t2676+t3022-t3027))./2.0+t4352.*t5857.*(t2694-t2701+t3036-t3043).*3.633675e-3+(t4346.*t5946.*(t2674-t2676+t3022-t3027))./2.0;
et330 = t3517.*t3934.*(-t56+t60+t649+t670+t686+t687+t1577+t1578+t1586+t1600+t2303+t2339+t2689+t3030+t3299+t3312).*(-1.444822e-2)-t3649.*t4915.*(-t56+t60+t649+t670+t686+t687+t1577+t1578+t1586+t1600+t2303+t2339+t2689+t3030+t3299+t3312).*1.444822e-2-(t3499.*t3910.*(-t321+t332+t1196+t1212+t1237+t1238+t2139+t2140+t2159+t2165+t2754+t2814+t2953+t3072+t3415+t3423))./2.0+(t4172.*t5647.*(et315+et316))./2.0+(t5958.*(et317+et318).*(t1488+t1874+t2519+t2740+t2747+t3096+t3097))./2.0;
et331 = t3934.*t3943.*t5491.*5.43845e-3+(t3910.*t3924.*t5647)./2.0-t3649.*t4920.*t5200.*1.444822e-2-(t3638.*t4879.*t5358)./2.0+t3934.*t4352.*t5859.*3.633675e-3+(t3910.*t4346.*t5958)./2.0+t4215.*t4920.*t5480.*5.43845e-3;
et332 = t4215.*t4915.*t5491.*(-5.43845e-3)+(t4172.*t4879.*t5645)./2.0+(t3638.*t3910.*(et319+et320))./2.0+(t4879.*t5946.*(t1488+t1874+t2519+t2740+t2747+t3096+t3097))./2.0-t4915.*t5859.*(t1513+t1879+t2598+t2820+t2834+t3117+t3118).*3.633675e-3+t4920.*t5857.*(t1513+t1879+t2598+t2820+t2834+t3117+t3118).*3.633675e-3+et321.*et322+(t3638.*(et323+et324).*(-t321+t332+t1196+t1212+t1237+t1238+t2139+t2140+t2159+t2165+t2754+t2814+t2953+t3072+t3415+t3423))./2.0;
et333 = t3582.*1.33637554986e-4+t3716-t3717+t27.*(t1896-t3239).*4.36041e-5;
et334 = t27.*t28.*(t1896-t3239).*7.26350557185e-5;
et335 = -t5014-t5083-t5103+t5106-t5455-t5745-t5747-t5751+t5814./2.0+t5842+t5853+t5986-t6091+t6121+t6234+t6373-t6394+t6396-t6568-t6574+t6576-t6619+t6620+t6968+t6972+t7102+t7112+(t6647.*(et333+et334))./2.0+(t3395.*(t3428-t3432-t4570+t4576+t4582-t4603))./2.0;
et336 = (t6682.*(t3524.*1.838876e-2-t3591+t3592+t16.*(t1861-t3221).*(3.0./5.0e+2)+t16.*t17.*(t1861-t3221).*9.99471e-3))./2.0+(t2388.*(-t3064+t4065+t3236.*(t1861-t3221).*9.840000000000001e-6))./2.0+(t5645.*t6013)./2.0+(t5647.*t6014)./2.0+(t5480.*t6256)./2.0+(t5491.*t6257)./2.0-(t5857.*t6059)./2.0-(t5859.*t6060)./2.0;
et337 = t5946.*t6031.*(-1.0./2.0)-(t5958.*t6032)./2.0+(t3055.*(-t3080+t4100+t11.*t3236.*(t1861-t3221).*1.02e-6))./2.0+(t3217.*(t3993+t4240-t4332+t4464+t4031.*(t2801-t2850)+t4026.*(t335-t1539-t2831+t2851)))./2.0+(t3216.*(-t4236+t4330+t4645+t3213.*(t1896-t3239)+t4019.*(t2801-t2850)+t21.*t3893.*(t1896-t3239)))./2.0;
et338 = t707+t708-t721-t722-t749+t762+t768-t777-t792-t793-t801-t802-t808+t813-t819+t821-t1629+t1637-t1640-t1641-t1659-t1661+t1666+t1667+t1683+t1692+t1705-t1712+t1758+t1759+t1775+t1776+t1973+t1993+t1994+t2023+t2053+t2060-t2089-t2090+t2098+t2099-t8.*t9.*t15.*t50.*t189.*3.670836568391568e-22;
et339 = t10.*t13.*t14.*t50.*t189.*(-3.279367663374749e-19)-t8.*t9.*t11.*t15.*t50.*t189.*7.075931802640439e-19;
et340 = t8.*t11.*t14.*t15.*t50.*t189.*(-1.190170786299927e-18)-t9.*t11.*t13.*t15.*t50.*t189.*1.190170786299927e-18;
et341 = t13.*t14.*t15.*t16.*t50.*t189.*(-3.226512155691387e-19);
et342 = t3704+t3707-t3863+t4904+t4912-t5154+t5155-t5186+t3370.*(t1477-t2502).*9.3e-7+t4031.*(t3512-t4006).*9.0e-8+t12.*t3980.*(t3242-t3554).*9.0e-8;
et343 = t17.*t3980.*(t3242-t3554).*9.3e-7;
et344 = t707+t708-t721-t722-t749+t762+t768-t777-t792-t793-t801-t802-t808+t813-t819+t821-t1629+t1637-t1640-t1641-t1659-t1661+t1666+t1667+t1683+t1692+t1705-t1712+t1758+t1759+t1775+t1776+t1973+t1993+t1994+t2023+t2053+t2060-t2089-t2090+t2098+t2099-t8.*t9.*t15.*t50.*t189.*3.670836568391568e-22;
et345 = t10.*t13.*t14.*t50.*t189.*(-3.279367663374749e-19)-t8.*t9.*t11.*t15.*t50.*t189.*7.075931802640439e-19;
et346 = t8.*t11.*t14.*t15.*t50.*t189.*(-1.190170786299927e-18)-t9.*t11.*t13.*t15.*t50.*t189.*1.190170786299927e-18;
et347 = t13.*t14.*t15.*t16.*t50.*t189.*(-3.226512155691387e-19);
et348 = -t5813+t6066+t6086-t6112+t6171-t6180+t6283-t6425+t6460-t6469+t6700-t6705+t6706-t6742+t6744-t6962-t6964+t7114+t7170+t7176-t7326+t7328+t7410+(t5026.*(et344+et345+et346+et347))./2.0+(t7092.*(t1477-t2502))./2.0;
et349 = (t6647.*(t3359-t3670+t22.*(t3242-t3554).*1.33637554986e-4+t28.*(t3242-t3554).*7.26350557185e-5))./2.0;
et350 = (t3055.*(t3131+t3132+t3171+t3446-t4281-t4282-t4301+t4303-t4308+t4310-t4583-t4594+t4623+t4639+t2388.*(t1456-t2355).*4.0e-8+(t3543.*(t1861-t3221))./1.0e+8+(t3500.*(t1896-t3239))./1.0e+8-t11.*t2297.*t2363.*2.4e-7))./2.0;
et351 = (t2363.*(t3157+t3158+t3386-t4299-t4300-t4562+t4567+t3543.*(t1861-t3221).*6.2e-7+t3500.*(t1896-t3239).*6.2e-7-(t11.*(t1861-t3221).*(t1896-t3239))./1.0e+8-(t11.*t2297.*t2363)./1.0e+8-(t11.*t3502.*t3547)./1.0e+8))./2.0+(t5859.*(t4927+t5198-t5762-t6392))./2.0;
et352 = (t21.*t2363.*(-t3434+t4606+t3980.*(t1896-t3239).*1.02e-6))./2.0;
et353 = t3582.*1.33637554986e-4+t3716-t3717+t27.*(t1896-t3239).*4.36041e-5;
et354 = t27.*t28.*(t1896-t3239).*7.26350557185e-5;
et355 = t6093+t6731+t6737+t6781+t6782+t6785+t6786-t7041-t7048+t7204+t7206+(t3976.*(t4573.*(t2813-t2835+t12.*(t1456-t2355).*1.02e-6+t17.*(t1456-t2355).*9.0e-8)+t4577.*(-t2804+t2838+t3109+t17.*(t1456-t2355).*9.3e-7)+t3133.*(t3242-t3554)))./2.0;
et356 = (t5543.*(t1456-t2355))./2.0+(t4001.*(t4359-t5236+t4604.*(-t2804+t2838+t3109+t17.*(t1456-t2355).*9.3e-7)))./2.0;
et357 = t50.*t189.*(-t4504+t4515+t3395.*(t2813-t2835+t12.*(t1456-t2355).*1.02e-6+t17.*(t1456-t2355).*9.0e-8)+t3396.*(-t2804+t2838+t3109+t17.*(t1456-t2355).*9.3e-7));
et358 = 4.771516396025243e-17;
et359 = t7857+t30.*(et303+et304+et305+et306)+t33.*(et307+et308+et309+et310)-t31.*(et325+et326+et327+et328+et329+et330+et331+et332)+t32.*(et335+et336+et337)+dq2.*dq4.*(t3129+t3200+t3201+t3208+t3468+t3482+t3488+t3590+t3817+t3818+t3890+t3896+t4208+t4339+t4341+t4415+t4416+t5587+t5592+t5720+t5724+t5905+t5910+t6008+t6015+t6445+t6450+t6503+t6507-t6672+t6687+t6690-t7255+t7257+t7261-t7263+(t5594.*(et338+et339+et340+et341))./2.0);
et360 = -dq2.*dq3.*(t2965+t2966+t3195+t3205+t3318+t3324+t3474+t3496+t3688+t3689+t3770+t3823+t3906+t3967+t4244+t4286+t4458+t4461+t4486+t4488+t4663+t4665+t4728+t4730+t5653+t5658-t5675-t5677-t5920+t5934+t5947+t6131+t6134+t6162+t6166+t6291+t6297-t6323+t6656+t6658+t6673+t6679+t7226+t7230+t7232+t7234+t4215.*t5466.*(t2694-t2701+t3036-t3043).*5.43845e-3+t3934.*t5857.*(t1513+t1879+t2598+t2820+t2834+t3117+t3118).*3.633675e-3);
et361 = dq3.*dq5.*(t5344+t5568+t5628+t5649+t5651+t5686+t5688+t5881+t5897+t5900+t5966+t5981+t5982+t6177+t6241+t6366+t6368+t6431+t6433+t6437+t6465+t6468+t6770+t6771+t6903+t7035+t7040+t7301+t7303+t7360+t7363+t7613+t7617+t3810.*t5480.*(t2694-t2701+t3036-t3043).*5.43845e-3+t3951.*t5857.*(t2694-t2701+t3036-t3043).*3.633675e-3);
et362 = dq5.*dq6.*(t6062+t6831+t6834+t6894+t6900-t7024-t7025+t7197+t7200+t7398+(t3395.*(et342+et343))./2.0+(t5792.*(t1477-t2502))./2.0+(t3055.*(t4876+t4905+t4906+t3055.*(t1456-t2355).*1.02e-6+t3047.*(t1477-t2502).*1.02e-6+t3976.*(t3242-t3554).*1.02e-6))./2.0);
et363 = -dq2.*dq5.*(t3416+t3765+t3766+t4030+t4039+t4041+t4270+t4272+t4318+t4372+t4373+t5999+t6001+t6043+t6046+t6457+t6459+t6519+t6521-t7266+t7267+t7269+(t5856.*(t4853.*(t1896-t3239).*7.26735e-3+t2363.*(t684+t685-t710+t724+t1686-t1690+t1700+t1701+t2371+t2698+t2707-t2716+t2719+t3329-t3337-t3351-t3641+t3643+t3655-t3659+t4114+t4115).*7.26735e-3))./2.0)+dq4.*dq5.*(et348+et349+et350+et351+et352);
et364 = -dq2.*dq5.*(t3416+t3765+t3766+t4030+t4039+t4041+t4270+t4272+t4318+t4372+t4373+t5997+t6000+t6045+t6047+t6455+t6458+t6520+t6522-t7272+t7273+t7275+(t5911.*(t4814.*(t1861-t3221)+t2297.*(t642+t643-t667+t674+t1587+t1606+t1608+t1609+t2295+t2671+t2683+t2684-t2695+t3279+t3297-t3303+t3597+t3603+t3609-t3614+t4053+t4054)))./2.0)+dq3.*dq6.*(t5590+t5968+t5970+t6205-t6209+t6270+t6508+t6509+t6820+t6821+t6825+t6828+t7315+t7316)+dq3.*dq6.*(t5827+t5993+t5995+t6342-t6355+t6924+t6925+t7062+t7063+t7196+t7654+t7657)-dq2.*dq4.*(t3126+t3193+t3194+t3209+t3463+t3480+t3490+t3588+t3820+t3821+t3891+t3895+t4205+t4337+t4342+t4413+t4417-t5589-t5593+t5718+t5721-t5907-t5914+t6007+t6009+t6452+t6502+t6504+t6858+t6859+t6868+t6870+t7243+t7245+t7248+t7251+(t5858.*(et353+et354))./2.0);
et365 = dq4.*dq5.*(t5343+t5430+t5496+t5497+t5565+t5851+t5877+t5880+t6096+t6152+t6153+t6157+t6192+t6195+t6217+t6225+t6231+t6238+t6483+t6484+t6582+t6595+t6601+t6612+t6614+t6645+t6648+t6994+t6996+t7118+t7125+t7159+t7161+t7416+t7419)+dq4.*dq6.*(t5567+t6119+t6219+t6226-t6635+t6639+t6640+t6643-t6692-t6694+t7057+t7064+t7156+(t6682.*(-t4045+t4049+t12.*(t1861-t3221).*1.838876e-2+t17.*(t1861-t3221).*9.99471e-3))./2.0);
et366 = dq3.*dq4.*(t5105+t5257+t5259+t5468+t5575+t5578+t5725+t5753+t5763+t5835+t5840+t5909+t5915+t5956+t5988+t6125+t6141+t6303-t6309+t6523+t6526+t6569+t6571+t6575+t6628+t6629+t6664+t7043+t7051+t7095+t7098+t7148+t7150+t7279+t7342+t7343+t7349+t7472+t7491+t7495+t7607+t7610+(t3712.*t5645.*(t2674-t2676+t3022-t3027))./2.0+(t3322.*t3910.*(-t321+t332+t1196+t1212+t1237+t1238+t2139+t2140+t2159+t2165+t2754+t2814+t2953+t3072+t3415+t3423))./2.0);
et367 = dq3.*dq4.*(t4489+t5247+t5249+t5251+t5306+t5376+t5384+t5385+t5389+t5421+t5449+t5451+t5549+t5555+t5557+t5613+t5643+t5869+t5892+t5894+t5928+t5931+t5937+t6023+t6053+t6081+t6143+t6144+t6184-t6188+t6201+t6227+t6307+t6311+t6419+t6512+t6514+t6554+t6558+t6607+t6795+t6800+t6882+t7003+t7005+t7007+t7009+t7294+t7295+t7351+t7352+t7599+t7603+t3755.*t5480.*(t2694-t2701+t3036-t3043).*5.43845e-3+t3369.*t3934.*(-t56+t60+t649+t670+t686+t687+t1577+t1578+t1586+t1600+t2303+t2339+t2689+t3030+t3299+t3312).*1.444822e-2)-dq1.*dq6.*t7710.*2.0-dq2.*dq6.*t7711-dq2.*dq6.*t7712-dq1.*dq5.*t7835.*2.0-dq1.*dq4.*t7880.*2.0;
et368 = dq1.*dq2.*t7937.*2.0-dq1.*dq3.*t7966.*2.0+dq5.*dq6.*(et355+et356)+dq3.*dq5.*(t5574+t5679+t5689+t5925+t5927+t5976+t6088+t6295+t6314+t6528+t6540+t6717+t6757+t6760+t6808+t7028+t7031+t7298+t7358+t7359+t7378+t7532+t7537+t7538+t7624+t7628+(t3808.*t5645.*(t2674-t2676+t3022-t3027))./2.0+(t3925.*t5946.*(t2674-t2676+t3022-t3027))./2.0)-dq2.*dq3.*(t2965+t2966+t3195+t3205+t3318+t3324+t3474+t3496+t3688+t3689+t3770+t3823+t3906+t3967+t4244+t4286+t4458+t4461+t4486+t4488+t4677+t4680+t4704+t4708+t5775+t5777-t5787-t5788-t6020+t6026+t6028+t6129+t6133+t6164+t6168+t6407+t6409-t6421+t6654+t6657+t6678+t6680+t7224+t7229+t7233+t7235+(t4172.*t5603.*(t2674-t2676+t3022-t3027))./2.0+(t3910.*t5946.*(t1488+t1874+t2519+t2740+t2747+t3096+t3097))./2.0);
et369 = dq4.*dq6.*(t5820+t6361-t6788-t6792+t6877+t6879+t7034+t7039+t7142+t7371+t7372+(t6647.*(t3566.*1.33637554986e-4+t4157-t4158+t28.*(t1896-t3239).*7.26350557185e-5))./2.0+et357.*et358);
et370 = -t5547-t5584-t5585-t5825+t6076+t6341-t6346+t6377+t6379./2.0+t6491+t6493+t6727+t6728+t6985+t7162+t7174+t7179;
et371 = t5858.*(t4371.*(t1896-t3239).*7.26735e-3+t2363.*(t3328+t3344+t3642-t3658+t22.*(t3242-t3554).*1.838876e-2+t28.*(t3242-t3554).*9.99471e-3).*7.26735e-3).*(-1.0./2.0);
et372 = (t5313.*(t4853.*(t1896-t3239).*7.26735e-3+t2363.*(t684+t685-t710+t724+t1686-t1690+t1700+t1701+t2371+t2698+t2707-t2716+t2719+t3329-t3337-t3351-t3641+t3643+t3655-t3659+t4114+t4115).*7.26735e-3))./2.0-(t5860.*t6064)./2.0-(t5949.*t6039)./2.0-(t5962.*t6041)./2.0+(t6681.*(t1477-t2502))./2.0+(t6913.*(t1861-t3221))./2.0;
et373 = (t3055.*(t3435-t3448+t4615+t4619+t3976.*(t1896-t3239).*5.7e-7+t3980.*(t1896-t3239).*4.0e-8))./2.0;
et374 = t4746-t5085+t5091-t5214+t4920.*(t1861-t3221).*7.83e-6+t3934.*(t951+t10.*(-t1881+t3121+t3276)).*7.83e-6+t4118.*(t2694-t2701+t3036-t3043).*7.83e-6;
et375 = t3934.*(-t1901+t3122+t3277).*3.24e-6;
et376 = -t2306-t2317+t3145+t3148+t35.*t941.*t948.*(t850-t874).*3.775747223193135e-1;
et377 = t36.*t941.*t948.*(t850-t874).*2.244797987218524e-1;
et378 = -t2306-t2317+t3145+t3148+t35.*t941.*t948.*(t850-t874).*3.775747223193135e-1;
et379 = t36.*t941.*t948.*(t850-t874).*2.244797987218524e-1;
et380 = -t2306-t2317+t3145+t3148+t35.*t941.*t948.*(t850-t874).*3.775747223193135e-1;
et381 = t36.*t941.*t948.*(t850-t874).*2.244797987218524e-1;
et382 = -t2306-t2317+t3145+t3148+t35.*t941.*t948.*(t850-t874).*3.775747223193135e-1;
et383 = t36.*t941.*t948.*(t850-t874).*2.244797987218524e-1;
et384 = -t2748-t2749+t2773+t2781-t2788+t3211+t3471+t4032-t4047+t262.*(t46-t47).*2.075672598245148e-23;
et385 = t264.*(t46-t47).*1.875105520197095e-20;
et386 = t50.*t202.*(t4757-t5088-t5090+t5097-t5098+t3913.*(t2694-t2701+t3036-t3043).*1.6e-7+t3934.*(-t1881+t3121+t3276).*1.6e-7+t3934.*(-t1901+t3122+t3277).*5.0e-8);
et387 = 2.836813422250052e-17;
et388 = t5038+t5387-t5415-t5416-t5673+t5779-t5781+t5784-t5896-t5938+t5941+t5990-t6019+t6024-t6115+t6116+t6202-t6271-t6272+t6398+t6423-t6440-t6442+t6515-t6518+t6602-t6803+t6897-t6965+t6966+t7014+t7016+t7055+t7086+t7090+t7304-t7311-t7312+t7319+t7385./2.0+t7436+t7596+t7641./2.0;
et389 = (t201.*(t4213+t5016+t123.*t188.*(t2694-t2701+t3036-t3043).*2.442490654175345e-23+t50.*t189.*t4915.*(t42-t43).*2.711709361697228e-39))./2.0;
et390 = (t3395.*(t5508-t5515+t5598+t5599-t5605-t5611+t4920.*(t3985+t12.*(t1861-t3221)).*9.3e-7+t4915.*(t3512-t4006).*9.0e-8))./2.0+(t2363.*(et374+et375))./2.0+(t6696.*(t2527-t3009))./2.0+(t5141.*(et376+et377))./2.0;
et391 = t3934.*t4215.*(t1554+t2361+t2362+t2367+t2414+t3961+t3968+t4198+t4201+t11.*(-t1901+t3122+t3277).*5.68686e-3).*5.43845e-3;
et392 = t4172.*(et378+et379).*(t350+t366-t1205+t1210-t1217-t1218-t2147+t2152+t2154+t2155-t3405-t3409-t3420-t3739+t3746+t26.*t50.*t202.*(t46-t47).*8.687615694748404e-39).*(-1.0./2.0);
et393 = t3517.*t5201.*(t2694-t2701+t3036-t3043).*1.444822e-2+(t3499.*t5359.*(t2674-t2676+t3022-t3027))./2.0+t3649.*t5560.*(t2694-t2701+t3036-t3043).*1.444822e-2+t3943.*t5483.*(t2694-t2701+t3036-t3043).*5.43845e-3+(t3924.*t5646.*(t2674-t2676+t3022-t3027))./2.0;
et394 = t4352.*t5858.*(t2694-t2701+t3036-t3043).*3.633675e-3+(t4346.*t5949.*(t2674-t2676+t3022-t3027))./2.0+(t3638.*t5362.*(et380+et381))./2.0+(t5962.*(et382+et383).*(t1488+t1874+t2519+t2740+t2747+t3096+t3097))./2.0;
et395 = t3910.*t3924.*(t350+t366-t1205+t1210-t1217-t1218-t2147+t2152+t2154+t2155-t3405-t3409-t3420-t3739+t3746+t26.*t50.*t202.*(t46-t47).*8.687615694748404e-39).*(-1.0./2.0);
et396 = t3517.*t3934.*t5205.*(-1.444822e-2)-(t3499.*t3910.*t5362)./2.0-t3649.*t4915.*t5205.*1.444822e-2-t3649.*t4920.*t5201.*1.444822e-2-(t3638.*t4879.*t5359)./2.0+t3934.*t4352.*t5860.*3.633675e-3+(t3910.*t4346.*t5962)./2.0;
et397 = t4215.*t4920.*t5483.*5.43845e-3+(t4172.*t4879.*t5646)./2.0+(t3638.*t3910.*(et384+et385))./2.0+(t4879.*t5949.*(t1488+t1874+t2519+t2740+t2747+t3096+t3097))./2.0-t4915.*t5860.*(t1513+t1879+t2598+t2820+t2834+t3117+t3118).*3.633675e-3+t4920.*t5858.*(t1513+t1879+t2598+t2820+t2834+t3117+t3118).*3.633675e-3+et386.*et387;
et398 = t3934.*t3943.*(t410-t5466).*(-5.43845e-3)+t4215.*t4915.*(t410-t5466).*5.43845e-3;
et399 = t3582.*1.33637554986e-4+t3716-t3717+t27.*(t1896-t3239).*4.36041e-5;
et400 = t27.*t28.*(t1896-t3239).*7.26350557185e-5;
et401 = -t5014-t5083-t5103+t5106-t5455-t5745-t5747-t5751+t5814./2.0+t5842+t5853+t5986-t6091+t6121+t6234+t6373-t6394+t6396-t6568-t6574+t6576-t6619+t6620+t6968+t6972+t7102+t7112+(t6647.*(et399+et400))./2.0+(t3395.*(t3428-t3432-t4570+t4576+t4582-t4603))./2.0;
et402 = t6014.*(t350+t366-t1205+t1210-t1217-t1218-t2147+t2152+t2154+t2155-t3405-t3409-t3420-t3739+t3746+t26.*t50.*t202.*(t46-t47).*8.687615694748404e-39).*(-1.0./2.0);
et403 = (t6682.*(t3524.*1.838876e-2-t3591+t3592+t16.*(t1861-t3221).*(3.0./5.0e+2)+t16.*t17.*(t1861-t3221).*9.99471e-3))./2.0+(t2388.*(-t3064+t4065+t3236.*(t1861-t3221).*9.840000000000001e-6))./2.0+(t5646.*t6013)./2.0+(t5483.*t6256)./2.0-(t5858.*t6059)./2.0-(t5860.*t6060)./2.0-(t5949.*t6031)./2.0-(t5962.*t6032)./2.0;
et404 = (t3055.*(-t3080+t4100+t11.*t3236.*(t1861-t3221).*1.02e-6))./2.0-(t6257.*(t410-t5466))./2.0+(t3217.*(t3993+t4240-t4332+t4464+t4031.*(t2801-t2850)+t4026.*(t335-t1539-t2831+t2851)))./2.0+(t3216.*(-t4236+t4330+t4645+t3213.*(t1896-t3239)+t4019.*(t2801-t2850)+t21.*t3893.*(t1896-t3239)))./2.0;
et405 = t3704+t3707-t3863+t4904+t4912-t5154+t5155-t5186+t3370.*(t1477-t2502).*9.3e-7+t4031.*(t3512-t4006).*9.0e-8+t12.*t3980.*(t3242-t3554).*9.0e-8;
et406 = t17.*t3980.*(t3242-t3554).*9.3e-7;
et407 = t3582.*1.33637554986e-4+t3716-t3717+t27.*(t1896-t3239).*4.36041e-5;
et408 = t27.*t28.*(t1896-t3239).*7.26350557185e-5;
et409 = t707+t708-t721-t722-t749+t762+t768-t777-t792-t793-t801-t802-t808+t813-t819+t821-t1629+t1637-t1640-t1641-t1659-t1661+t1666+t1667+t1683+t1692+t1705-t1712+t1758+t1759+t1775+t1776+t1973+t1993+t1994+t2023+t2053+t2060-t2089-t2090+t2098+t2099-t8.*t9.*t15.*t50.*t189.*3.670836568391568e-22;
et410 = t10.*t13.*t14.*t50.*t189.*(-3.279367663374749e-19)-t8.*t9.*t11.*t15.*t50.*t189.*7.075931802640439e-19;
et411 = t8.*t11.*t14.*t15.*t50.*t189.*(-1.190170786299927e-18)-t9.*t11.*t13.*t15.*t50.*t189.*1.190170786299927e-18;
et412 = t13.*t14.*t15.*t16.*t50.*t189.*(-3.226512155691387e-19);
et413 = t707+t708-t721-t722-t749+t762+t768-t777-t792-t793-t801-t802-t808+t813-t819+t821-t1629+t1637-t1640-t1641-t1659-t1661+t1666+t1667+t1683+t1692+t1705-t1712+t1758+t1759+t1775+t1776+t1973+t1993+t1994+t2023+t2053+t2060-t2089-t2090+t2098+t2099-t8.*t9.*t15.*t50.*t189.*3.670836568391568e-22;
et414 = t10.*t13.*t14.*t50.*t189.*(-3.279367663374749e-19)-t8.*t9.*t11.*t15.*t50.*t189.*7.075931802640439e-19;
et415 = t8.*t11.*t14.*t15.*t50.*t189.*(-1.190170786299927e-18)-t9.*t11.*t13.*t15.*t50.*t189.*1.190170786299927e-18;
et416 = t13.*t14.*t15.*t16.*t50.*t189.*(-3.226512155691387e-19);
et417 = -t5813+t6066+t6086-t6112+t6174+t6283-t6425+t6460-t6469+t6702-t6705+t6708-t6742+t6744-t6962-t6964+t7114+t7170+t7176-t7326+t7328+t7412;
et418 = (t5278.*(t350+t366-t1205+t1210-t1217-t1218-t2147+t2152+t2154+t2155-t3405-t3409-t3420-t3739+t3746+t26.*t50.*t202.*(t46-t47).*8.687615694748404e-39))./2.0+(t5026.*(et413+et414+et415+et416))./2.0+(t7092.*(t1477-t2502))./2.0;
et419 = (t6647.*(t3359-t3670+t22.*(t3242-t3554).*1.33637554986e-4+t28.*(t3242-t3554).*7.26350557185e-5))./2.0;
et420 = (t3055.*(t3131+t3132+t3171+t3446-t4281-t4282-t4301+t4303-t4308+t4310-t4583-t4594+t4623+t4639+t2388.*(t1456-t2355).*4.0e-8+(t3543.*(t1861-t3221))./1.0e+8+(t3500.*(t1896-t3239))./1.0e+8-t11.*t2297.*t2363.*2.4e-7))./2.0;
et421 = (t2363.*(t3157+t3158+t3386-t4299-t4300-t4562+t4567+t3543.*(t1861-t3221).*6.2e-7+t3500.*(t1896-t3239).*6.2e-7-(t11.*(t1861-t3221).*(t1896-t3239))./1.0e+8-(t11.*t2297.*t2363)./1.0e+8-(t11.*t3502.*t3547)./1.0e+8))./2.0+(t5860.*(t4927+t5198-t5762-t6392))./2.0;
et422 = (t21.*t2363.*(-t3434+t4606+t3980.*(t1896-t3239).*1.02e-6))./2.0;
et423 = -t5344-t5568+t5626+t5650+t5652+t5685+t5687+t5879+t5884+t5898+t5899-t5966+t5980+t6170+t6182-t6241+t6367+t6432+t6435+t6436+t6466+t6467+t6768+t6769+t6904-t7040+t7300+t7302-t7363+t7614+t7618;
et424 = (t4118.*(t4573.*(t2813-t2835+t12.*(t1456-t2355).*1.02e-6+t17.*(t1456-t2355).*9.0e-8)+t4577.*(-t2804+t2838+t3109+t17.*(t1456-t2355).*9.3e-7)+t3133.*(t3242-t3554)))./2.0;
et425 = (t6651.*(t4814.*(t1861-t3221)+t2297.*(t642+t643-t667+t674+t1587+t1606+t1608+t1609+t2295+t2671+t2683+t2684-t2695+t3279+t3297-t3303+t3597+t3603+t3609-t3614+t4053+t4054)))./2.0+(t5809.*(t951+t10.*(-t1881+t3121+t3276)))./2.0+((t1861-t3221).*(t4658+t4719+t5240+t5262-t3483.*(t1005+t20.*(t1941-t3315+t39.*t1022.*(t855-t878).*2.196325630278387e-1))-t3431.*(t1896-t3239)))./2.0;
et426 = t6093+t6732+t6739+t6781+t6782+t6785+t6786-t7041-t7048+t7204+t7206+(t3976.*(t4573.*(t2813-t2835+t12.*(t1456-t2355).*1.02e-6+t17.*(t1456-t2355).*9.0e-8)+t4577.*(-t2804+t2838+t3109+t17.*(t1456-t2355).*9.3e-7)+t3133.*(t3242-t3554)))./2.0;
et427 = (t5543.*(t1456-t2355))./2.0+(t4001.*(t4359-t5236+t4604.*(-t2804+t2838+t3109+t17.*(t1456-t2355).*9.3e-7)))./2.0;
et428 = t50.*t189.*(-t4504+t4515+t3395.*(t2813-t2835+t12.*(t1456-t2355).*1.02e-6+t17.*(t1456-t2355).*9.0e-8)+t3396.*(-t2804+t2838+t3109+t17.*(t1456-t2355).*9.3e-7));
et429 = 4.771516396025243e-17;
et430 = t7857+t33.*(et370+et371+et372+et373)-t29.*t7937-t31.*(et388+et389+et390+et391+et392+et393+et394+et395+et396+et397+et398)+t32.*(et401+et402+et403+et404);
et431 = dq5.*dq6.*(t6062+t6833+t6835+t6894+t6900-t7024-t7025+t7197+t7200+t7398+(t3395.*(et405+et406))./2.0+(t5792.*(t1477-t2502))./2.0+(t3055.*(t4876+t4905+t4906+t3055.*(t1456-t2355).*1.02e-6+t3047.*(t1477-t2502).*1.02e-6+t3976.*(t3242-t3554).*1.02e-6))./2.0);
et432 = -dq1.*dq4.*(t3126+t3193+t3194+t3209+t3463+t3480+t3490+t3588+t3820+t3821+t3891+t3895+t4205+t4337+t4342+t4413+t4417-t5589-t5593+t5718+t5721-t5907-t5914+t6007+t6009+t6452+t6502+t6504-t6672+t6687+t6690-t7255+t7257+t7261-t7263+(t5594.*(et409+et410+et411+et412))./2.0+(t5858.*(et407+et408))./2.0)+dq3.*dq6.*(t5590+t5968+t5970+t6207-t6210+t6270+t6508+t6509+t6820+t6821+t6825+t6828+t7315+t7316)+dq3.*dq6.*(t5827+t5993+t5995+t6347-t6358+t6924+t6925+t7062+t7063+t7196+t7654+t7657);
et433 = dq3.*dq4.*(t4489+t5247+t5249+t5251+t5306+t5376+t5384+t5385+t5389+t5421+t5449+t5451+t5549+t5555+t5557+t5615+t5631+t5643+t5871+t5892+t5894+t5928+t5931+t5937+t6023+t6053+t6081+t6143+t6144+t6186-t6189+t6201+t6227+t6307+t6311+t6419+t6513+t6517+t6554+t6558+t6607+t6795+t6800+t6882+t7003+t7005+t7007+t7009+t7294+t7295+t7351+t7352+t7601+t7605+t3755.*t5483.*(t2694-t2701+t3036-t3043).*5.43845e-3)+dq4.*dq5.*(t5343+t5430+t5496+t5497+t5565+t5851+t5877+t5880+t6096+t6152+t6153+t6157+t6192+t6195+t6217+t6225+t6233+t6240+t6483+t6484+t6582+t6595+t6601+t6612+t6614+t6646+t6649+t6994+t6996+t7118+t7125+t7159+t7161+t7417+t7421);
et434 = dq4.*dq6.*(t5567+t6119+t6219+t6226-t6635+t6639+t6640+t6643-t6693-t6695+t7057+t7064+t7156+(t6682.*(-t4045+t4049+t12.*(t1861-t3221).*1.838876e-2+t17.*(t1861-t3221).*9.99471e-3))./2.0)+dq4.*dq5.*(et417+et418+et419+et420+et421+et422)-dq3.*dq5.*(et423+et424+et425);
et435 = dq3.*dq4.*(t5105+t5257+t5259+t5468+t5575+t5578+t5725+t5753+t5765+t5769+t5835+t5840+t5909+t5915+t5959+t5988+t6125+t6141+t6306-t6312+t6523+t6526+t6570+t6572+t6575+t6628+t6629+t6664+t7043+t7051+t7095+t7098+t7148+t7150+t7279+t7342+t7343+t7349+t7472+t7491+t7495+t7609+t7611+(t3712.*t5646.*(t2674-t2676+t3022-t3027))./2.0)-dq1.*dq6.*t7711-dq1.*dq6.*t7712-dq2.*dq6.*t7713.*2.0-dq2.*dq5.*t7836.*2.0+dq2.*dq4.*t7881.*2.0-dq1.*dq5.*t7963-dq1.*dq5.*t7964-dq2.*dq3.*t7965.*2.0-dq1.*dq3.*t7975+dq1.*dq4.*t7974-dq1.*dq3.*t7976+dq5.*dq6.*(et426+et427)+dq3.*dq5.*(t5574+t5679+t5689+t5925+t5927+t5978+t6088+t6299+t6314+t6528+t6540+t6717+t6757+t6760+t6808+t7028+t7031+t7298+t7358+t7359+t7378+t7532+t7537+t7538+t7626+t7629+(t3808.*t5646.*(t2674-t2676+t3022-t3027))./2.0+(t3925.*t5949.*(t2674-t2676+t3022-t3027))./2.0);
et436 = dq4.*dq6.*(t5820+t6361-t6789-t6799+t6877+t6879+t7034+t7039+t7142+t7371+t7372+(t6647.*(t3566.*1.33637554986e-4+t4157-t4158+t28.*(t1896-t3239).*7.26350557185e-5))./2.0+et428.*et429);
et437 = t1288+t1289+t1302+t1303-t1319-t1320+t1336-t1348+t1350+t1351-t1360+t1369-t1378+t1396-t1425+t1435-t2174+t2183-t2187+t2193-t2194-t2195+t2199-t2203-t2215+t2219-t2222-t2223+t2239+t2240-t2256-t2257+t2555+t2556+t2572+t2583-t2605-t2606+t2612+t2613-t2618-t2619+t2651+t2652;
et438 = t18.*t19.*t20.*t50.*t202.*(-3.566935413776081e-21);
et439 = t24.*t25.*t26.*t50.*t202.*(-3.992732227073824e-24);
et440 = t18.*t19.*t26.*t27.*t50.*t202.*(-3.509445006623964e-21);
et441 = t21.*t24.*t25.*t26.*t50.*t202.*(-7.696420262413979e-21);
et442 = t707+t708-t721-t722-t749+t762+t768-t777-t792-t793-t801-t802-t808+t813-t819+t821-t1629+t1637-t1640-t1641-t1659-t1661+t1666+t1667+t1683+t1692+t1705-t1712+t1758+t1759+t1775+t1776+t1973+t1993+t1994+t2023+t2053+t2060-t2089-t2090+t2098+t2099-t8.*t9.*t15.*t50.*t189.*3.670836568391568e-22;
et443 = t10.*t13.*t14.*t50.*t189.*(-3.279367663374749e-19)-t8.*t9.*t11.*t15.*t50.*t189.*7.075931802640439e-19;
et444 = t8.*t11.*t14.*t15.*t50.*t189.*(-1.190170786299927e-18)-t9.*t11.*t13.*t15.*t50.*t189.*1.190170786299927e-18;
et445 = t13.*t14.*t15.*t16.*t50.*t189.*(-3.226512155691387e-19);
et446 = t1288+t1289+t1302+t1303-t1319-t1320+t1336-t1348+t1350+t1351-t1360+t1369-t1378+t1396-t1425+t1435-t2174+t2183-t2187+t2193-t2194-t2195+t2199-t2203-t2215+t2219-t2222-t2223+t2239+t2240-t2256-t2257+t2555+t2556+t2572+t2583-t2605-t2606+t2612+t2613-t2618-t2619+t2651+t2652;
et447 = t18.*t19.*t20.*t50.*t202.*(-3.566935413776081e-21);
et448 = t24.*t25.*t26.*t50.*t202.*(-3.992732227073824e-24);
et449 = t18.*t19.*t26.*t27.*t50.*t202.*(-3.509445006623964e-21);
et450 = t21.*t24.*t25.*t26.*t50.*t202.*(-7.696420262413979e-21);
et451 = t4923+t4924-t5678+t5684+t6918-t6919+t6920-t6987+t7164+t7408+t7427-t7444-t7496+t7668+t7669+t7670-t7737-t7789+t7790+t7868+t7876+t7895-t7896-t7910-t7911+((t2674-t2676+t3022-t3027).*(t5243+t5265-t5821+t3543.*(-t3064+t4065+t3236.*(t1861-t3221).*9.840000000000001e-6)+t5043.*(t1896-t3239)))./2.0+(t3910.*(t5411-t5563+t6762-t6765+t4604.*(t3428-t3432-t4570+t4576+t4582-t4603)+t6244.*(t3563-t4051)))./2.0+(t3880.*t3901)./2.0+(t3805.*t4274)./2.0+(t3902.*t4324)./2.0;
et452 = (t4008.*t4273)./2.0+(t3216.*t7379)./2.0+(t3217.*t7380)./2.0+(t3216.*t7799)./2.0-(t3216.*t7804)./2.0+(t3217.*t7805)./2.0+(t3910.*t7281)./2.0-(t3910.*t7716)./2.0+(t5783.*(et437+et438+et439+et440+et441))./2.0-(t3217.*(t5637+t5773-t6685-t6910+t6911+t6490.*(t3563-t4051)))./2.0+(t7715.*(t2674-t2676+t3022-t3027))./2.0-(t7748.*(t2674-t2676+t3022-t3027))./2.0+(t6650.*(t5034-t5280-t6302+t7166))./2.0+(t7083.*(-t1901+t3122+t3277))./2.0+(t7433.*(-t1901+t3122+t3277))./2.0+(t7470.*(-t1901+t3122+t3277))./2.0;
et453 = t50.*t189.*(t2363.*t5346-t2363.*t5353-t2388.*t5345+t2388.*t6004+t50.*t202.*t5352.*9.543032792050485e-17).*4.771516396025243e-17+t3755.*t6011.*(t2694-t2701+t3036-t3043).*5.43845e-3+(t3712.*t6255.*(t2674-t2676+t3022-t3027))./2.0;
et454 = t4215.*t6013.*(t2694-t2701+t3036-t3043).*5.43845e-3+(t4172.*t6256.*(t2674-t2676+t3022-t3027))./2.0-(t3975.*t6682.*(t2674-t2676+t3022-t3027))./2.0-t4018.*t6647.*(t2694-t2701+t3036-t3043).*3.633675e-3-(t6059.*(t2674-t2676+t3022-t3027).*(t1488+t1874+t2519+t2740+t2747+t3096+t3097))./2.0;
et455 = t6031.*(t2694-t2701+t3036-t3043).*(t1513+t1879+t2598+t2820+t2834+t3117+t3118).*(-3.633675e-3)+t3755.*t3934.*(et442+et443+et444+et445).*5.43845e-3-t50.*t189.*t7758.*4.771516396025243e-17;
et456 = t50.*t189.*t7791.*(-4.771516396025243e-17)+t3934.*t4215.*t6014.*5.43845e-3+(t3910.*t4172.*t6257)./2.0-(t3910.*t3975.*t6689)./2.0-t3934.*t4018.*t6650.*3.633675e-3-(t3910.*t6060.*(t1488+t1874+t2519+t2740+t2747+t3096+t3097))./2.0;
et457 = t3934.*t6032.*(t1513+t1879+t2598+t2820+t2834+t3117+t3118).*(-3.633675e-3)-(t3712.*t3910.*(et446+et447+et448+et449+et450))./2.0-t236.*t241.*t4343.*t5036.*1.16903445774439e-94;
et458 = t236.*t241.*t4375.*t5025.*(-1.16903445774439e-94);
et459 = t236.*t241.*t4705.*t5037.*(-1.16903445774439e-94);
et460 = t236.*t241.*t4716.*t5027.*(-1.16903445774439e-94);
et461 = t5793+t5796+t4577.*(t4618+t4634-t12.*t2363.*t3047.*9.0e-8-t17.*t2363.*t3047.*9.3e-7+t12.*t3980.*(t1896-t3239).*9.0e-8+t17.*t3980.*(t1896-t3239).*9.3e-7);
et462 = t4573.*(t4617+t4635-t12.*t2363.*t3047.*1.02e-6-t17.*t2363.*t3047.*9.0e-8+t12.*t3980.*(t1896-t3239).*1.02e-6+t17.*t3980.*(t1896-t3239).*9.0e-8);
et463 = t22.*t6675.*(t3242-t3554)+t28.*t6674.*(t3242-t3554);
et464 = t5537+t5542+t7443+t7456+t7518+t7519+t7557+t7559+t7686+t7687+t7692+t7694+t7902+t7906+t7922+t7923+t7931+t7933-(t3502.*t7725)./2.0-(t3502.*t7798)./2.0+(t3910.*t7795)./2.0-(t3910.*(t5669-t6476-t6478+t6875+t4026.*(t3435-t3448+t4615+t4619+t3976.*(t1896-t3239).*5.7e-7+t3980.*(t1896-t3239).*4.0e-8)))./2.0-(t7724.*(t1861-t3221))./2.0;
et465 = (t2297.*(t5618+t6429-t6902+t3055.*(t4795+t4801+t4808+t3976.*(t2694-t2701+t3036-t3043).*5.7e-7)+t6384.*(t1477-t2502)))./2.0-(t7704.*(t2674-t2676+t3022-t3027))./2.0-((t1861-t3221).*(-t5828-t5829+t6593+t6596+t22.*t6699.*(t3242-t3554)+t28.*t6696.*(t3242-t3554)))./2.0;
et466 = t2297.*(t6462-t6464-t6766-t6767+t3055.*(t4809+t3976.*(t2694-t2701+t3036-t3043).*1.02e-6)+t5572.*(t1477-t2502)).*(-1.0./2.0)-((t2674-t2676+t3022-t3027).*(et461+et462+et463))./2.0;
et467 = (t3925.*(t4853.*(t1896-t3239).*7.26735e-3+t2363.*(t684+t685-t710+t724+t1686-t1690+t1700+t1701+t2371+t2698+t2707-t2716+t2719+t3329-t3337-t3351-t3641+t3643+t3655-t3659+t4114+t4115).*7.26735e-3).*(t2674-t2676+t3022-t3027))./2.0;
et468 = t3951.*(t4814.*(t1861-t3221)+t2297.*(t642+t643-t667+t674+t1587+t1606+t1608+t1609+t2295+t2671+t2683+t2684-t2695+t3279+t3297-t3303+t3597+t3603+t3609-t3614+t4053+t4054)).*(t2694-t2701+t3036-t3043).*3.633675e-3;
et469 = (t4371.*(t1896-t3239).*7.26735e-3+t2363.*(t3328+t3344+t3642-t3658+t22.*(t3242-t3554).*1.838876e-2+t28.*(t3242-t3554).*9.99471e-3).*7.26735e-3).*(t2674-t2676+t3022-t3027).*(t1488+t1874+t2519+t2740+t2747+t3096+t3097).*(-1.0./2.0);
et470 = t6039.*(t2694-t2701+t3036-t3043).*(t1513+t1879+t2598+t2820+t2834+t3117+t3118).*(-3.633675e-3)+t3934.*t3951.*t6711.*3.633675e-3+(t3910.*t3925.*t6793)./2.0-(t3910.*t6064.*(t1488+t1874+t2519+t2740+t2747+t3096+t3097))./2.0-t3934.*t6041.*(t1513+t1879+t2598+t2820+t2834+t3117+t3118).*3.633675e-3;
et471 = t236.*t241.*t4314.*t4763.*(-2.394182569460511e-91);
et472 = t236.*t241.*t4260.*t4850.*(-2.394182569460511e-91);
et473 = t236.*t241.*t4716.*t4762.*(-2.394182569460511e-91);
et474 = t236.*t241.*t4705.*t4847.*(-2.394182569460511e-91);
et475 = t6413+t7401+t4880.*(t4795+t4801+t4808+t3976.*(t2694-t2701+t3036-t3043).*5.7e-7)+t4031.*(t5287+t5291-t5328+t5333+t5337-t5340+t4835.*(t2694-t2701+t3036-t3043).*5.7e-7+t4838.*(t2694-t2701+t3036-t3043).*4.0e-8);
et476 = t4026.*(-t5202+t5286+t5297+t5331-t5332-t5336+t5341+(t4920.*(t1861-t3221))./1.0e+8+(t3934.*(t951+t10.*(-t1881+t3121+t3276)))./1.0e+8+(t4118.*(t2694-t2701+t3036-t3043))./1.0e+8+t4835.*(t2694-t2701+t3036-t3043).*4.0e-8+t4838.*(t2694-t2701+t3036-t3043).*2.4e-7);
et477 = t4872.*(-t4494-t4495+t4799+t4823+t3976.*(t2694-t2701+t3036-t3043).*4.0e-8+t3980.*(t2694-t2701+t3036-t3043).*2.4e-7);
et478 = t237.*6.47e-6;
et479 = t238.*5.84482e-3-t50.*t189.*3.311325901843639e-18;
et480 = t10.*t50.*t189.*3.31613276532711e-19-t15.*t50.*t189.*3.670836568391568e-22;
et481 = -t2306-t2317+t3145+t3148+t35.*t941.*t948.*(t850-t874).*3.775747223193135e-1;
et482 = t36.*t941.*t948.*(t850-t874).*2.244797987218524e-1;
et483 = t3237.*(t4744-t5084+t5087-t5089-t5096+t3913.*(t2694-t2701+t3036-t3043).*5.0e-8+t3934.*(-t1881+t3121+t3276).*5.0e-8+t3934.*(-t1901+t3122+t3277).*1.1e-7)-t3931.*t5917-t3937.*t5916;
et484 = t3238.*(t4757-t5088-t5090+t5097-t5098+t3913.*(t2694-t2701+t3036-t3043).*1.6e-7+t3934.*(-t1881+t3121+t3276).*1.6e-7+t3934.*(-t1901+t3122+t3277).*5.0e-8)+(t201.*t5028.*(t46-t47))./9.007199254740992e+15;
et485 = t50.*t202.*(t46-t47).*(t4213+t5016+t123.*t188.*(t2694-t2701+t3036-t3043).*2.442490654175345e-23+t50.*t189.*t4915.*(t42-t43).*2.711709361697228e-39).*(-1.232595164407831e-32);
et486 = t262.*1.869599668e-7;
et487 = t264.*1.688944904408e-4;
et488 = t50.*t202.*(-9.568553024307061e-20);
et489 = t20.*t50.*t202.*9.582443148530891e-21;
et490 = t26.*t50.*t202.*(-1.060741086483328e-23);
et491 = -t2306-t2317+t3145+t3148+t35.*t941.*t948.*(t850-t874).*3.775747223193135e-1;
et492 = t36.*t941.*t948.*(t850-t874).*2.244797987218524e-1;
et493 = t3236.*(t4744-t5084+t5087-t5089-t5096+t3913.*(t2694-t2701+t3036-t3043).*5.0e-8+t3934.*(-t1881+t3121+t3276).*5.0e-8+t3934.*(-t1901+t3122+t3277).*1.1e-7);
et494 = t5917.*(t1941-t3315+t39.*t1022.*(t855-t878).*2.196325630278387e-1)-t5916.*(t1959-t3313+t38.*t1022.*(t855-t878).*2.196325630278387e-1);
et495 = -t3235.*(t4757-t5088-t5090+t5097-t5098+t3913.*(t2694-t2701+t3036-t3043).*1.6e-7+t3934.*(-t1881+t3121+t3276).*1.6e-7+t3934.*(-t1901+t3122+t3277).*5.0e-8)-(t140.*t201.*t5028)./9.007199254740992e+15;
et496 = (t50.*t140.*t202.*(t4213+t5016+t123.*t188.*(t2694-t2701+t3036-t3043).*2.442490654175345e-23+t50.*t189.*t4915.*(t42-t43).*2.711709361697228e-39))./8.112963841460668e+31;
et497 = -t2306-t2317+t3145+t3148+t35.*t941.*t948.*(t850-t874).*3.775747223193135e-1;
et498 = t36.*t941.*t948.*(t850-t874).*2.244797987218524e-1;
et499 = -t2306-t2317+t3145+t3148+t35.*t941.*t948.*(t850-t874).*3.775747223193135e-1;
et500 = t36.*t941.*t948.*(t850-t874).*2.244797987218524e-1;
et501 = -t2306-t2317+t3145+t3148+t35.*t941.*t948.*(t850-t874).*3.775747223193135e-1;
et502 = t36.*t941.*t948.*(t850-t874).*2.244797987218524e-1;
et503 = -t2306-t2317+t3145+t3148+t35.*t941.*t948.*(t850-t874).*3.775747223193135e-1;
et504 = t36.*t941.*t948.*(t850-t874).*2.244797987218524e-1;
et505 = -t2306-t2317+t3145+t3148+t35.*t941.*t948.*(t850-t874).*3.775747223193135e-1;
et506 = t36.*t941.*t948.*(t850-t874).*2.244797987218524e-1;
tau_c = ft_17({dq1,dq2,dq3,dq4,dq5,dq6,et359,et360,et361,et362,et363,et364,et365,et366,et367,et368,et369,et430,et431,et432,et433,et434,et435,et436,et451,et452,et453,et454,et455,et456,et457,et458,et459,et460,et464,et465,et466,et467,et468,et469,et470,et471,et472,et473,et474,et475,et476,et477,et478,et479,et480,et481,et482,et483,et484,et485,et486,et487,et488,et489,et490,et491,et492,et493,et494,et495,et496,et497,et498,et499,et500,et501,et502,et503,et504,et505,et506,t10,t1005,t1022,t11,t12,t1205,t1210,t1217,t1218,t1288,t1289,t13,t1302,t1303,t1319,t1320,t1336,t1348,t1350,t1351,t1360,t1369,t1378,t1396,t14,t140,t1425,t1435,t1456,t1477,t1488,t15,t1513,t1539,t1587,t16,t1606,t1608,t1609,t1629,t1637,t1640,t1641,t1659,t1661,t1666,t1667,t1683,t1686,t1690,t1692,t17,t1700,t1701,t1705,t1712,t1758,t1759,t1775,t1776,t18,t1861,t1874,t1879,t188,t1881,t189,t1896,t19,t1901,t1941,t1959,t1973,t1993,t1994,t20,t201,t202,t2023,t2053,t2060,t2089,t2090,t2098,t2099,t21,t2147,t2152,t2154,t2155,t2174,t2183,t2187,t2193,t2194,t2195,t2199,t22,t2203,t2215,t2219,t2222,t2223,t2239,t2240,t2256,t2257,t2292,t2295,t2297,t2306,t2307,t2317,t2337,t2338,t2355,t236,t2363,t2368,t237,t2371,t2388,t2399,t24,t241,t2419,t25,t2502,t2519,t2555,t2556,t2572,t2583,t2598,t26,t2605,t2606,t2612,t2613,t2618,t2619,t2651,t2652,t2671,t2674,t2676,t2683,t2684,t2694,t2695,t2698,t27,t2701,t2707,t2716,t2719,t2740,t2747,t28,t2801,t2804,t2813,t2820,t2831,t2834,t2835,t2838,t2850,t2851,t29,t2994,t30,t3015,t3022,t3027,t3036,t3043,t3047,t3055,t3064,t3068,t3080,t3096,t3097,t31,t3109,t3117,t3118,t3121,t3122,t3126,t3131,t3132,t3133,t3145,t3148,t3157,t3158,t3171,t3193,t3194,t32,t3209,t3216,t3217,t3221,t3235,t3236,t3237,t3238,t3239,t3242,t3276,t3277,t3279,t3290,t3297,t33,t3303,t3313,t3315,t3328,t3329,t3337,t3340,t3344,t335,t3351,t3359,t3370,t3386,t3395,t34,t3405,t3409,t3420,t3428,t3431,t3432,t3434,t3435,t3446,t3448,t3463,t3480,t3483,t3490,t3499,t35,t350,t3500,t3502,t3503,t3512,t3517,t3524,t3543,t3547,t3554,t3563,t3566,t3582,t3588,t3591,t3592,t3597,t36,t3603,t3609,t3611,t3614,t3638,t3639,t3640,t3641,t3642,t3643,t3649,t3655,t3658,t3659,t366,t3670,t3703,t3704,t3707,t3708,t3716,t3717,t3739,t3746,t38,t3808,t3809,t3810,t3820,t3821,t3840,t3846,t3856,t3862,t3863,t3891,t3895,t39,t3901,t3902,t3903,t3910,t3915,t3924,t3925,t3934,t3943,t3951,t3974,t3975,t3976,t3980,t3991,t3993,t4001,t4006,t4008,t4018,t4019,t4026,t4031,t4035,t4045,t4049,t4051,t4053,t4054,t4065,t4100,t4109,t4110,t4114,t4115,t4118,t4146,t4165,t4172,t4187,t42,t4205,t4215,t4240,t4261,t4263,t4273,t4274,t4275,t4281,t4282,t4287,t4288,t4299,t43,t4300,t4301,t4303,t4308,t4310,t4324,t4325,t4326,t4332,t4334,t4337,t4342,t4346,t4352,t4371,t4413,t4417,t4464,t4468,t4470,t4476,t4494,t4495,t4501,t4502,t4518,t4553,t4559,t4562,t4563,t4567,t4570,t4573,t4576,t4577,t4582,t4583,t4594,t46,t4603,t4604,t4606,t4615,t4617,t4618,t4619,t4623,t4634,t4635,t4639,t4644,t4652,t4658,t4673,t4675,t4678,t4683,t47,t4703,t4705,t4709,t4713,t4716,t4719,t4722,t4724,t4725,t4741,t4746,t4751,t4760,t4761,t4762,t4763,t4795,t4799,t4801,t4808,t4809,t4814,t4823,t4835,t4838,t4843,t4844,t4847,t4850,t4853,t4872,t4874,t4876,t4879,t4880,t4887,t4903,t4904,t4905,t4906,t4911,t4912,t4915,t4920,t4923,t4924,t4925,t4927,t4950,t50,t5025,t5026,t5027,t5028,t5034,t5036,t5037,t5041,t5042,t5043,t5080,t5085,t5086,t5091,t5093,t5108,t5119,t5153,t5154,t5155,t5161,t5164,t5167,t5169,t5183,t5184,t5185,t5186,t5189,t5190,t5194,t5198,t5202,t5213,t5214,t5240,t5243,t5262,t5264,t5265,t5278,t5279,t5280,t5283,t5286,t5287,t5291,t5296,t5297,t5301,t5302,t5303,t5304,t5308,t5309,t5328,t5331,t5332,t5333,t5336,t5337,t5340,t5341,t5343,t5344,t5346,t5361,t5363,t5370,t5372,t5381,t5382,t5391,t5392,t5393,t5395,t5399,t5400,t5401,t5402,t5403,t5404,t5405,t5411,t5425,t5430,t5433,t5434,t5436,t5437,t5438,t5439,t5452,t5453,t5454,t5456,t5457,t5458,t5459,t5460,t5464,t5481,t5487,t5488,t5490,t5493,t5494,t5495,t5496,t5499,t5523,t5535,t5536,t5537,t5538,t5539,t5542,t5544,t5545,t5548,t5550,t5563,t5565,t5568,t5569,t5570,t5572,t5580,t5581,t5586,t5589,t5593,t5594,t5604,t5607,t5618,t5637,t5645,t5646,t5669,t5678,t5679,t5684,t5689,t5691,t5698,t5699,t5713,t5714,t5718,t5721,t5723,t5730,t5731,t5734,t5735,t5738,t5739,t5741,t5742,t5758,t5759,t5760,t5761,t5762,t5767,t5771,t5773,t5782,t5783,t5790,t5791,t5792,t5793,t5796,t5804,t5809,t5813,t5816,t5819,t5821,t5828,t5829,t5849,t5851,t5857,t5858,t5859,t5860,t5876,t5880,t5886,t5901,t5902,t5907,t5914,t5916,t5917,t5918,t5925,t5927,t5939,t5946,t5949,t5954,t5955,t5966,t5976,t5978,t5980,t6004,t6005,t6007,t6009,t6011,t6013,t6014,t6031,t6032,t6039,t6041,t6054,t6058,t6059,t6060,t6064,t6065,t6066,t6083,t6086,t6095,t6098,t6100,t6102,t6112,t6135,t6137,t6149,t6151,t6156,t6159,t6160,t6172,t6174,t6178,t6190,t6192,t6193,t6194,t6196,t6223,t6228,t6230,t6231,t6233,t6237,t6239,t6241,t6244,t6250,t6251,t6255,t6256,t6257,t6261,t6263,t6275,t6278,t6281,t6283,t6287,t6295,t6299,t6302,t6305,t6326,t6360,t6362,t6364,t6367,t6371,t6376,t6384,t6392,t6402,t6413,t642,t6425,t6428,t6429,t643,t6443,t6452,t6460,t6462,t6464,t6469,t6476,t6478,t6482,t6490,t6502,t6504,t6510,t6528,t6540,t6549,t6564,t6565,t6580,t6584,t6585,t6589,t6593,t6594,t6596,t6609,t6610,t6611,t6613,t6616,t6617,t6622,t6623,t6635,t6639,t6640,t6643,t6645,t6646,t6647,t6648,t6649,t6650,t6651,t6665,t667,t6672,t6674,t6675,t6681,t6682,t6685,t6687,t6689,t6690,t6692,t6693,t6694,t6695,t6696,t6699,t6702,t6704,t6705,t6708,t6711,t6719,t6722,t6724,t6725,t6736,t6738,t674,t6742,t6744,t6745,t6747,t6751,t6762,t6765,t6766,t6767,t6772,t6776,t6778,t6779,t6783,t6787,t6793,t684,t6848,t685,t6852,t6872,t6873,t6875,t6884,t6886,t6887,t6888,t6902,t6910,t6911,t6916,t6918,t6919,t6920,t6959,t6962,t6964,t6971,t6975,t6979,t6983,t6987,t6989,t6992,t6993,t6995,t6997,t7000,t7001,t7010,t7011,t7012,t7013,t7019,t7020,t7022,t7023,t7024,t7025,t7027,t7028,t7031,t7032,t7033,t7037,t7038,t7040,t7059,t7066,t707,t708,t7080,t7083,t7084,t7088,t7092,t710,t7101,t7114,t7118,t7125,t7134,t7156,t7159,t7161,t7164,t7166,t7170,t7176,t7182,t7187,t7199,t7205,t7207,t7208,t721,t7211,t7215,t7216,t7217,t7218,t7219,t722,t7220,t7221,t7222,t7228,t7231,t7237,t7238,t724,t7240,t7242,t7246,t7250,t7253,t7254,t7255,t7256,t7257,t7260,t7261,t7263,t7264,t7277,t7281,t7283,t7292,t7300,t7302,t7307,t7310,t7326,t7328,t7335,t7336,t7337,t7344,t7345,t7346,t7347,t7353,t7354,t7355,t7363,t7364,t7367,t7369,t7370,t7373,t7387,t7388,t7394,t7397,t7398,t7401,t7402,t7404,t7405,t7406,t7407,t7408,t7409,t7410,t7412,t7420,t7426,t7427,t7428,t7429,t7430,t7432,t7433,t7439,t7440,t7442,t7443,t7444,t7446,t7447,t7448,t7450,t7451,t7453,t7454,t7456,t7458,t7461,t7462,t7463,t7464,t7465,t7466,t7469,t7470,t7473,t7479,t7480,t7482,t7483,t7487,t7489,t749,t7496,t7498,t7501,t7502,t7505,t7507,t7508,t7509,t7510,t7511,t7512,t7514,t7516,t7518,t7519,t7523,t7524,t7529,t7530,t7542,t7544,t7545,t7546,t7548,t7549,t7550,t7551,t7552,t7553,t7554,t7557,t7559,t7560,t7561,t7562,t7563,t7564,t7565,t7566,t7567,t7568,t7575,t7577,t7579,t7582,t7583,t7584,t7585,t7586,t7587,t7589,t7612,t7614,t7616,t7618,t762,t7630,t7631,t7633,t7634,t7635,t7636,t7638,t7639,t7645,t7646,t7647,t7648,t7650,t7651,t7658,t7660,t7662,t7663,t7668,t7669,t7670,t7672,t7673,t7674,t7675,t7676,t7677,t7678,t7679,t768,t7680,t7682,t7683,t7684,t7686,t7687,t7688,t7690,t7691,t7692,t7694,t7695,t7696,t7697,t7698,t7699,t7701,t7704,t7707,t7710,t7711,t7712,t7713,t7714,t7715,t7716,t7718,t7719,t7720,t7721,t7723,t7726,t7727,t7730,t7732,t7734,t7736,t7737,t7738,t7740,t7741,t7744,t7745,t7746,t7748,t7751,t7752,t7753,t7755,t7756,t7759,t7760,t7762,t7763,t7764,t7765,t7766,t7768,t7769,t777,t7771,t7772,t7773,t7775,t7778,t7780,t7781,t7783,t7784,t7786,t7787,t7788,t7789,t7790,t7792,t7793,t7795,t7796,t7799,t7802,t7804,t7806,t7807,t7808,t7809,t7810,t7811,t7813,t7814,t7815,t7816,t7817,t7818,t7819,t7820,t7821,t7822,t7823,t7824,t7826,t7827,t7828,t7830,t7831,t7832,t7833,t7835,t7836,t7838,t7839,t7840,t7841,t7842,t7846,t7847,t7848,t7849,t7850,t7854,t7855,t7859,t7861,t7862,t7863,t7864,t7866,t7868,t7869,t7870,t7871,t7872,t7873,t7874,t7876,t7877,t7878,t7879,t7880,t7881,t7883,t7885,t7887,t7888,t7890,t7891,t7892,t7894,t7895,t7896,t7897,t7898,t7900,t7901,t7902,t7904,t7905,t7906,t7907,t7908,t7909,t7910,t7911,t7912,t7913,t7914,t7917,t7918,t7919,t792,t7920,t7921,t7922,t7923,t7924,t7925,t7926,t7927,t7928,t7929,t793,t7931,t7933,t7934,t7936,t7938,t7939,t7940,t7942,t7943,t7944,t7945,t7948,t7949,t7951,t7952,t7953,t7954,t7955,t7956,t7957,t7958,t7959,t7960,t7961,t7962,t7963,t7964,t7965,t7966,t7971,t7972,t7974,t7975,t7976,t7977,t7983,t7984,t7985,t7986,t7987,t7988,t8,t801,t802,t808,t813,t819,t821,t850,t855,t874,t878,t9,t941,t948,t951});
end
function tau_c = ft_17(ct)
dq1 = ct{1};
dq2 = ct{2};
dq3 = ct{3};
dq4 = ct{4};
dq5 = ct{5};
dq6 = ct{6};
et359 = ct{7};
et360 = ct{8};
et361 = ct{9};
et362 = ct{10};
et363 = ct{11};
et364 = ct{12};
et365 = ct{13};
et366 = ct{14};
et367 = ct{15};
et368 = ct{16};
et369 = ct{17};
et430 = ct{18};
et431 = ct{19};
et432 = ct{20};
et433 = ct{21};
et434 = ct{22};
et435 = ct{23};
et436 = ct{24};
et451 = ct{25};
et452 = ct{26};
et453 = ct{27};
et454 = ct{28};
et455 = ct{29};
et456 = ct{30};
et457 = ct{31};
et458 = ct{32};
et459 = ct{33};
et460 = ct{34};
et464 = ct{35};
et465 = ct{36};
et466 = ct{37};
et467 = ct{38};
et468 = ct{39};
et469 = ct{40};
et470 = ct{41};
et471 = ct{42};
et472 = ct{43};
et473 = ct{44};
et474 = ct{45};
et475 = ct{46};
et476 = ct{47};
et477 = ct{48};
et478 = ct{49};
et479 = ct{50};
et480 = ct{51};
et481 = ct{52};
et482 = ct{53};
et483 = ct{54};
et484 = ct{55};
et485 = ct{56};
et486 = ct{57};
et487 = ct{58};
et488 = ct{59};
et489 = ct{60};
et490 = ct{61};
et491 = ct{62};
et492 = ct{63};
et493 = ct{64};
et494 = ct{65};
et495 = ct{66};
et496 = ct{67};
et497 = ct{68};
et498 = ct{69};
et499 = ct{70};
et500 = ct{71};
et501 = ct{72};
et502 = ct{73};
et503 = ct{74};
et504 = ct{75};
et505 = ct{76};
et506 = ct{77};
t10 = ct{78};
t1005 = ct{79};
t1022 = ct{80};
t11 = ct{81};
t12 = ct{82};
t1205 = ct{83};
t1210 = ct{84};
t1217 = ct{85};
t1218 = ct{86};
t1288 = ct{87};
t1289 = ct{88};
t13 = ct{89};
t1302 = ct{90};
t1303 = ct{91};
t1319 = ct{92};
t1320 = ct{93};
t1336 = ct{94};
t1348 = ct{95};
t1350 = ct{96};
t1351 = ct{97};
t1360 = ct{98};
t1369 = ct{99};
t1378 = ct{100};
t1396 = ct{101};
t14 = ct{102};
t140 = ct{103};
t1425 = ct{104};
t1435 = ct{105};
t1456 = ct{106};
t1477 = ct{107};
t1488 = ct{108};
t15 = ct{109};
t1513 = ct{110};
t1539 = ct{111};
t1587 = ct{112};
t16 = ct{113};
t1606 = ct{114};
t1608 = ct{115};
t1609 = ct{116};
t1629 = ct{117};
t1637 = ct{118};
t1640 = ct{119};
t1641 = ct{120};
t1659 = ct{121};
t1661 = ct{122};
t1666 = ct{123};
t1667 = ct{124};
t1683 = ct{125};
t1686 = ct{126};
t1690 = ct{127};
t1692 = ct{128};
t17 = ct{129};
t1700 = ct{130};
t1701 = ct{131};
t1705 = ct{132};
t1712 = ct{133};
t1758 = ct{134};
t1759 = ct{135};
t1775 = ct{136};
t1776 = ct{137};
t18 = ct{138};
t1861 = ct{139};
t1874 = ct{140};
t1879 = ct{141};
t188 = ct{142};
t1881 = ct{143};
t189 = ct{144};
t1896 = ct{145};
t19 = ct{146};
t1901 = ct{147};
t1941 = ct{148};
t1959 = ct{149};
t1973 = ct{150};
t1993 = ct{151};
t1994 = ct{152};
t20 = ct{153};
t201 = ct{154};
t202 = ct{155};
t2023 = ct{156};
t2053 = ct{157};
t2060 = ct{158};
t2089 = ct{159};
t2090 = ct{160};
t2098 = ct{161};
t2099 = ct{162};
t21 = ct{163};
t2147 = ct{164};
t2152 = ct{165};
t2154 = ct{166};
t2155 = ct{167};
t2174 = ct{168};
t2183 = ct{169};
t2187 = ct{170};
t2193 = ct{171};
t2194 = ct{172};
t2195 = ct{173};
t2199 = ct{174};
t22 = ct{175};
t2203 = ct{176};
t2215 = ct{177};
t2219 = ct{178};
t2222 = ct{179};
t2223 = ct{180};
t2239 = ct{181};
t2240 = ct{182};
t2256 = ct{183};
t2257 = ct{184};
t2292 = ct{185};
t2295 = ct{186};
t2297 = ct{187};
t2306 = ct{188};
t2307 = ct{189};
t2317 = ct{190};
t2337 = ct{191};
t2338 = ct{192};
t2355 = ct{193};
t236 = ct{194};
t2363 = ct{195};
t2368 = ct{196};
t237 = ct{197};
t2371 = ct{198};
t2388 = ct{199};
t2399 = ct{200};
t24 = ct{201};
t241 = ct{202};
t2419 = ct{203};
t25 = ct{204};
t2502 = ct{205};
t2519 = ct{206};
t2555 = ct{207};
t2556 = ct{208};
t2572 = ct{209};
t2583 = ct{210};
t2598 = ct{211};
t26 = ct{212};
t2605 = ct{213};
t2606 = ct{214};
t2612 = ct{215};
t2613 = ct{216};
t2618 = ct{217};
t2619 = ct{218};
t2651 = ct{219};
t2652 = ct{220};
t2671 = ct{221};
t2674 = ct{222};
t2676 = ct{223};
t2683 = ct{224};
t2684 = ct{225};
t2694 = ct{226};
t2695 = ct{227};
t2698 = ct{228};
t27 = ct{229};
t2701 = ct{230};
t2707 = ct{231};
t2716 = ct{232};
t2719 = ct{233};
t2740 = ct{234};
t2747 = ct{235};
t28 = ct{236};
t2801 = ct{237};
t2804 = ct{238};
t2813 = ct{239};
t2820 = ct{240};
t2831 = ct{241};
t2834 = ct{242};
t2835 = ct{243};
t2838 = ct{244};
t2850 = ct{245};
t2851 = ct{246};
t29 = ct{247};
t2994 = ct{248};
t30 = ct{249};
t3015 = ct{250};
t3022 = ct{251};
t3027 = ct{252};
t3036 = ct{253};
t3043 = ct{254};
t3047 = ct{255};
t3055 = ct{256};
t3064 = ct{257};
t3068 = ct{258};
t3080 = ct{259};
t3096 = ct{260};
t3097 = ct{261};
t31 = ct{262};
t3109 = ct{263};
t3117 = ct{264};
t3118 = ct{265};
t3121 = ct{266};
t3122 = ct{267};
t3126 = ct{268};
t3131 = ct{269};
t3132 = ct{270};
t3133 = ct{271};
t3145 = ct{272};
t3148 = ct{273};
t3157 = ct{274};
t3158 = ct{275};
t3171 = ct{276};
t3193 = ct{277};
t3194 = ct{278};
t32 = ct{279};
t3209 = ct{280};
t3216 = ct{281};
t3217 = ct{282};
t3221 = ct{283};
t3235 = ct{284};
t3236 = ct{285};
t3237 = ct{286};
t3238 = ct{287};
t3239 = ct{288};
t3242 = ct{289};
t3276 = ct{290};
t3277 = ct{291};
t3279 = ct{292};
t3290 = ct{293};
t3297 = ct{294};
t33 = ct{295};
t3303 = ct{296};
t3313 = ct{297};
t3315 = ct{298};
t3328 = ct{299};
t3329 = ct{300};
t3337 = ct{301};
t3340 = ct{302};
t3344 = ct{303};
t335 = ct{304};
t3351 = ct{305};
t3359 = ct{306};
t3370 = ct{307};
t3386 = ct{308};
t3395 = ct{309};
t34 = ct{310};
t3405 = ct{311};
t3409 = ct{312};
t3420 = ct{313};
t3428 = ct{314};
t3431 = ct{315};
t3432 = ct{316};
t3434 = ct{317};
t3435 = ct{318};
t3446 = ct{319};
t3448 = ct{320};
t3463 = ct{321};
t3480 = ct{322};
t3483 = ct{323};
t3490 = ct{324};
t3499 = ct{325};
t35 = ct{326};
t350 = ct{327};
t3500 = ct{328};
t3502 = ct{329};
t3503 = ct{330};
t3512 = ct{331};
t3517 = ct{332};
t3524 = ct{333};
t3543 = ct{334};
t3547 = ct{335};
t3554 = ct{336};
t3563 = ct{337};
t3566 = ct{338};
t3582 = ct{339};
t3588 = ct{340};
t3591 = ct{341};
t3592 = ct{342};
t3597 = ct{343};
t36 = ct{344};
t3603 = ct{345};
t3609 = ct{346};
t3611 = ct{347};
t3614 = ct{348};
t3638 = ct{349};
t3639 = ct{350};
t3640 = ct{351};
t3641 = ct{352};
t3642 = ct{353};
t3643 = ct{354};
t3649 = ct{355};
t3655 = ct{356};
t3658 = ct{357};
t3659 = ct{358};
t366 = ct{359};
t3670 = ct{360};
t3703 = ct{361};
t3704 = ct{362};
t3707 = ct{363};
t3708 = ct{364};
t3716 = ct{365};
t3717 = ct{366};
t3739 = ct{367};
t3746 = ct{368};
t38 = ct{369};
t3808 = ct{370};
t3809 = ct{371};
t3810 = ct{372};
t3820 = ct{373};
t3821 = ct{374};
t3840 = ct{375};
t3846 = ct{376};
t3856 = ct{377};
t3862 = ct{378};
t3863 = ct{379};
t3891 = ct{380};
t3895 = ct{381};
t39 = ct{382};
t3901 = ct{383};
t3902 = ct{384};
t3903 = ct{385};
t3910 = ct{386};
t3915 = ct{387};
t3924 = ct{388};
t3925 = ct{389};
t3934 = ct{390};
t3943 = ct{391};
t3951 = ct{392};
t3974 = ct{393};
t3975 = ct{394};
t3976 = ct{395};
t3980 = ct{396};
t3991 = ct{397};
t3993 = ct{398};
t4001 = ct{399};
t4006 = ct{400};
t4008 = ct{401};
t4018 = ct{402};
t4019 = ct{403};
t4026 = ct{404};
t4031 = ct{405};
t4035 = ct{406};
t4045 = ct{407};
t4049 = ct{408};
t4051 = ct{409};
t4053 = ct{410};
t4054 = ct{411};
t4065 = ct{412};
t4100 = ct{413};
t4109 = ct{414};
t4110 = ct{415};
t4114 = ct{416};
t4115 = ct{417};
t4118 = ct{418};
t4146 = ct{419};
t4165 = ct{420};
t4172 = ct{421};
t4187 = ct{422};
t42 = ct{423};
t4205 = ct{424};
t4215 = ct{425};
t4240 = ct{426};
t4261 = ct{427};
t4263 = ct{428};
t4273 = ct{429};
t4274 = ct{430};
t4275 = ct{431};
t4281 = ct{432};
t4282 = ct{433};
t4287 = ct{434};
t4288 = ct{435};
t4299 = ct{436};
t43 = ct{437};
t4300 = ct{438};
t4301 = ct{439};
t4303 = ct{440};
t4308 = ct{441};
t4310 = ct{442};
t4324 = ct{443};
t4325 = ct{444};
t4326 = ct{445};
t4332 = ct{446};
t4334 = ct{447};
t4337 = ct{448};
t4342 = ct{449};
t4346 = ct{450};
t4352 = ct{451};
t4371 = ct{452};
t4413 = ct{453};
t4417 = ct{454};
t4464 = ct{455};
t4468 = ct{456};
t4470 = ct{457};
t4476 = ct{458};
t4494 = ct{459};
t4495 = ct{460};
t4501 = ct{461};
t4502 = ct{462};
t4518 = ct{463};
t4553 = ct{464};
t4559 = ct{465};
t4562 = ct{466};
t4563 = ct{467};
t4567 = ct{468};
t4570 = ct{469};
t4573 = ct{470};
t4576 = ct{471};
t4577 = ct{472};
t4582 = ct{473};
t4583 = ct{474};
t4594 = ct{475};
t46 = ct{476};
t4603 = ct{477};
t4604 = ct{478};
t4606 = ct{479};
t4615 = ct{480};
t4617 = ct{481};
t4618 = ct{482};
t4619 = ct{483};
t4623 = ct{484};
t4634 = ct{485};
t4635 = ct{486};
t4639 = ct{487};
t4644 = ct{488};
t4652 = ct{489};
t4658 = ct{490};
t4673 = ct{491};
t4675 = ct{492};
t4678 = ct{493};
t4683 = ct{494};
t47 = ct{495};
t4703 = ct{496};
t4705 = ct{497};
t4709 = ct{498};
t4713 = ct{499};
t4716 = ct{500};
t4719 = ct{501};
t4722 = ct{502};
t4724 = ct{503};
t4725 = ct{504};
t4741 = ct{505};
t4746 = ct{506};
t4751 = ct{507};
t4760 = ct{508};
t4761 = ct{509};
t4762 = ct{510};
t4763 = ct{511};
t4795 = ct{512};
t4799 = ct{513};
t4801 = ct{514};
t4808 = ct{515};
t4809 = ct{516};
t4814 = ct{517};
t4823 = ct{518};
t4835 = ct{519};
t4838 = ct{520};
t4843 = ct{521};
t4844 = ct{522};
t4847 = ct{523};
t4850 = ct{524};
t4853 = ct{525};
t4872 = ct{526};
t4874 = ct{527};
t4876 = ct{528};
t4879 = ct{529};
t4880 = ct{530};
t4887 = ct{531};
t4903 = ct{532};
t4904 = ct{533};
t4905 = ct{534};
t4906 = ct{535};
t4911 = ct{536};
t4912 = ct{537};
t4915 = ct{538};
t4920 = ct{539};
t4923 = ct{540};
t4924 = ct{541};
t4925 = ct{542};
t4927 = ct{543};
t4950 = ct{544};
t50 = ct{545};
t5025 = ct{546};
t5026 = ct{547};
t5027 = ct{548};
t5028 = ct{549};
t5034 = ct{550};
t5036 = ct{551};
t5037 = ct{552};
t5041 = ct{553};
t5042 = ct{554};
t5043 = ct{555};
t5080 = ct{556};
t5085 = ct{557};
t5086 = ct{558};
t5091 = ct{559};
t5093 = ct{560};
t5108 = ct{561};
t5119 = ct{562};
t5153 = ct{563};
t5154 = ct{564};
t5155 = ct{565};
t5161 = ct{566};
t5164 = ct{567};
t5167 = ct{568};
t5169 = ct{569};
t5183 = ct{570};
t5184 = ct{571};
t5185 = ct{572};
t5186 = ct{573};
t5189 = ct{574};
t5190 = ct{575};
t5194 = ct{576};
t5198 = ct{577};
t5202 = ct{578};
t5213 = ct{579};
t5214 = ct{580};
t5240 = ct{581};
t5243 = ct{582};
t5262 = ct{583};
t5264 = ct{584};
t5265 = ct{585};
t5278 = ct{586};
t5279 = ct{587};
t5280 = ct{588};
t5283 = ct{589};
t5286 = ct{590};
t5287 = ct{591};
t5291 = ct{592};
t5296 = ct{593};
t5297 = ct{594};
t5301 = ct{595};
t5302 = ct{596};
t5303 = ct{597};
t5304 = ct{598};
t5308 = ct{599};
t5309 = ct{600};
t5328 = ct{601};
t5331 = ct{602};
t5332 = ct{603};
t5333 = ct{604};
t5336 = ct{605};
t5337 = ct{606};
t5340 = ct{607};
t5341 = ct{608};
t5343 = ct{609};
t5344 = ct{610};
t5346 = ct{611};
t5361 = ct{612};
t5363 = ct{613};
t5370 = ct{614};
t5372 = ct{615};
t5381 = ct{616};
t5382 = ct{617};
t5391 = ct{618};
t5392 = ct{619};
t5393 = ct{620};
t5395 = ct{621};
t5399 = ct{622};
t5400 = ct{623};
t5401 = ct{624};
t5402 = ct{625};
t5403 = ct{626};
t5404 = ct{627};
t5405 = ct{628};
t5411 = ct{629};
t5425 = ct{630};
t5430 = ct{631};
t5433 = ct{632};
t5434 = ct{633};
t5436 = ct{634};
t5437 = ct{635};
t5438 = ct{636};
t5439 = ct{637};
t5452 = ct{638};
t5453 = ct{639};
t5454 = ct{640};
t5456 = ct{641};
t5457 = ct{642};
t5458 = ct{643};
t5459 = ct{644};
t5460 = ct{645};
t5464 = ct{646};
t5481 = ct{647};
t5487 = ct{648};
t5488 = ct{649};
t5490 = ct{650};
t5493 = ct{651};
t5494 = ct{652};
t5495 = ct{653};
t5496 = ct{654};
t5499 = ct{655};
t5523 = ct{656};
t5535 = ct{657};
t5536 = ct{658};
t5537 = ct{659};
t5538 = ct{660};
t5539 = ct{661};
t5542 = ct{662};
t5544 = ct{663};
t5545 = ct{664};
t5548 = ct{665};
t5550 = ct{666};
t5563 = ct{667};
t5565 = ct{668};
t5568 = ct{669};
t5569 = ct{670};
t5570 = ct{671};
t5572 = ct{672};
t5580 = ct{673};
t5581 = ct{674};
t5586 = ct{675};
t5589 = ct{676};
t5593 = ct{677};
t5594 = ct{678};
t5604 = ct{679};
t5607 = ct{680};
t5618 = ct{681};
t5637 = ct{682};
t5645 = ct{683};
t5646 = ct{684};
t5669 = ct{685};
t5678 = ct{686};
t5679 = ct{687};
t5684 = ct{688};
t5689 = ct{689};
t5691 = ct{690};
t5698 = ct{691};
t5699 = ct{692};
t5713 = ct{693};
t5714 = ct{694};
t5718 = ct{695};
t5721 = ct{696};
t5723 = ct{697};
t5730 = ct{698};
t5731 = ct{699};
t5734 = ct{700};
t5735 = ct{701};
t5738 = ct{702};
t5739 = ct{703};
t5741 = ct{704};
t5742 = ct{705};
t5758 = ct{706};
t5759 = ct{707};
t5760 = ct{708};
t5761 = ct{709};
t5762 = ct{710};
t5767 = ct{711};
t5771 = ct{712};
t5773 = ct{713};
t5782 = ct{714};
t5783 = ct{715};
t5790 = ct{716};
t5791 = ct{717};
t5792 = ct{718};
t5793 = ct{719};
t5796 = ct{720};
t5804 = ct{721};
t5809 = ct{722};
t5813 = ct{723};
t5816 = ct{724};
t5819 = ct{725};
t5821 = ct{726};
t5828 = ct{727};
t5829 = ct{728};
t5849 = ct{729};
t5851 = ct{730};
t5857 = ct{731};
t5858 = ct{732};
t5859 = ct{733};
t5860 = ct{734};
t5876 = ct{735};
t5880 = ct{736};
t5886 = ct{737};
t5901 = ct{738};
t5902 = ct{739};
t5907 = ct{740};
t5914 = ct{741};
t5916 = ct{742};
t5917 = ct{743};
t5918 = ct{744};
t5925 = ct{745};
t5927 = ct{746};
t5939 = ct{747};
t5946 = ct{748};
t5949 = ct{749};
t5954 = ct{750};
t5955 = ct{751};
t5966 = ct{752};
t5976 = ct{753};
t5978 = ct{754};
t5980 = ct{755};
t6004 = ct{756};
t6005 = ct{757};
t6007 = ct{758};
t6009 = ct{759};
t6011 = ct{760};
t6013 = ct{761};
t6014 = ct{762};
t6031 = ct{763};
t6032 = ct{764};
t6039 = ct{765};
t6041 = ct{766};
t6054 = ct{767};
t6058 = ct{768};
t6059 = ct{769};
t6060 = ct{770};
t6064 = ct{771};
t6065 = ct{772};
t6066 = ct{773};
t6083 = ct{774};
t6086 = ct{775};
t6095 = ct{776};
t6098 = ct{777};
t6100 = ct{778};
t6102 = ct{779};
t6112 = ct{780};
t6135 = ct{781};
t6137 = ct{782};
t6149 = ct{783};
t6151 = ct{784};
t6156 = ct{785};
t6159 = ct{786};
t6160 = ct{787};
t6172 = ct{788};
t6174 = ct{789};
t6178 = ct{790};
t6190 = ct{791};
t6192 = ct{792};
t6193 = ct{793};
t6194 = ct{794};
t6196 = ct{795};
t6223 = ct{796};
t6228 = ct{797};
t6230 = ct{798};
t6231 = ct{799};
t6233 = ct{800};
t6237 = ct{801};
t6239 = ct{802};
t6241 = ct{803};
t6244 = ct{804};
t6250 = ct{805};
t6251 = ct{806};
t6255 = ct{807};
t6256 = ct{808};
t6257 = ct{809};
t6261 = ct{810};
t6263 = ct{811};
t6275 = ct{812};
t6278 = ct{813};
t6281 = ct{814};
t6283 = ct{815};
t6287 = ct{816};
t6295 = ct{817};
t6299 = ct{818};
t6302 = ct{819};
t6305 = ct{820};
t6326 = ct{821};
t6360 = ct{822};
t6362 = ct{823};
t6364 = ct{824};
t6367 = ct{825};
t6371 = ct{826};
t6376 = ct{827};
t6384 = ct{828};
t6392 = ct{829};
t6402 = ct{830};
t6413 = ct{831};
t642 = ct{832};
t6425 = ct{833};
t6428 = ct{834};
t6429 = ct{835};
t643 = ct{836};
t6443 = ct{837};
t6452 = ct{838};
t6460 = ct{839};
t6462 = ct{840};
t6464 = ct{841};
t6469 = ct{842};
t6476 = ct{843};
t6478 = ct{844};
t6482 = ct{845};
t6490 = ct{846};
t6502 = ct{847};
t6504 = ct{848};
t6510 = ct{849};
t6528 = ct{850};
t6540 = ct{851};
t6549 = ct{852};
t6564 = ct{853};
t6565 = ct{854};
t6580 = ct{855};
t6584 = ct{856};
t6585 = ct{857};
t6589 = ct{858};
t6593 = ct{859};
t6594 = ct{860};
t6596 = ct{861};
t6609 = ct{862};
t6610 = ct{863};
t6611 = ct{864};
t6613 = ct{865};
t6616 = ct{866};
t6617 = ct{867};
t6622 = ct{868};
t6623 = ct{869};
t6635 = ct{870};
t6639 = ct{871};
t6640 = ct{872};
t6643 = ct{873};
t6645 = ct{874};
t6646 = ct{875};
t6647 = ct{876};
t6648 = ct{877};
t6649 = ct{878};
t6650 = ct{879};
t6651 = ct{880};
t6665 = ct{881};
t667 = ct{882};
t6672 = ct{883};
t6674 = ct{884};
t6675 = ct{885};
t6681 = ct{886};
t6682 = ct{887};
t6685 = ct{888};
t6687 = ct{889};
t6689 = ct{890};
t6690 = ct{891};
t6692 = ct{892};
t6693 = ct{893};
t6694 = ct{894};
t6695 = ct{895};
t6696 = ct{896};
t6699 = ct{897};
t6702 = ct{898};
t6704 = ct{899};
t6705 = ct{900};
t6708 = ct{901};
t6711 = ct{902};
t6719 = ct{903};
t6722 = ct{904};
t6724 = ct{905};
t6725 = ct{906};
t6736 = ct{907};
t6738 = ct{908};
t674 = ct{909};
t6742 = ct{910};
t6744 = ct{911};
t6745 = ct{912};
t6747 = ct{913};
t6751 = ct{914};
t6762 = ct{915};
t6765 = ct{916};
t6766 = ct{917};
t6767 = ct{918};
t6772 = ct{919};
t6776 = ct{920};
t6778 = ct{921};
t6779 = ct{922};
t6783 = ct{923};
t6787 = ct{924};
t6793 = ct{925};
t684 = ct{926};
t6848 = ct{927};
t685 = ct{928};
t6852 = ct{929};
t6872 = ct{930};
t6873 = ct{931};
t6875 = ct{932};
t6884 = ct{933};
t6886 = ct{934};
t6887 = ct{935};
t6888 = ct{936};
t6902 = ct{937};
t6910 = ct{938};
t6911 = ct{939};
t6916 = ct{940};
t6918 = ct{941};
t6919 = ct{942};
t6920 = ct{943};
t6959 = ct{944};
t6962 = ct{945};
t6964 = ct{946};
t6971 = ct{947};
t6975 = ct{948};
t6979 = ct{949};
t6983 = ct{950};
t6987 = ct{951};
t6989 = ct{952};
t6992 = ct{953};
t6993 = ct{954};
t6995 = ct{955};
t6997 = ct{956};
t7000 = ct{957};
t7001 = ct{958};
t7010 = ct{959};
t7011 = ct{960};
t7012 = ct{961};
t7013 = ct{962};
t7019 = ct{963};
t7020 = ct{964};
t7022 = ct{965};
t7023 = ct{966};
t7024 = ct{967};
t7025 = ct{968};
t7027 = ct{969};
t7028 = ct{970};
t7031 = ct{971};
t7032 = ct{972};
t7033 = ct{973};
t7037 = ct{974};
t7038 = ct{975};
t7040 = ct{976};
t7059 = ct{977};
t7066 = ct{978};
t707 = ct{979};
t708 = ct{980};
t7080 = ct{981};
t7083 = ct{982};
t7084 = ct{983};
t7088 = ct{984};
t7092 = ct{985};
t710 = ct{986};
t7101 = ct{987};
t7114 = ct{988};
t7118 = ct{989};
t7125 = ct{990};
t7134 = ct{991};
t7156 = ct{992};
t7159 = ct{993};
t7161 = ct{994};
t7164 = ct{995};
t7166 = ct{996};
t7170 = ct{997};
t7176 = ct{998};
t7182 = ct{999};
t7187 = ct{1000};
t7199 = ct{1001};
t7205 = ct{1002};
t7207 = ct{1003};
t7208 = ct{1004};
t721 = ct{1005};
t7211 = ct{1006};
t7215 = ct{1007};
t7216 = ct{1008};
t7217 = ct{1009};
t7218 = ct{1010};
t7219 = ct{1011};
t722 = ct{1012};
t7220 = ct{1013};
t7221 = ct{1014};
t7222 = ct{1015};
t7228 = ct{1016};
t7231 = ct{1017};
t7237 = ct{1018};
t7238 = ct{1019};
t724 = ct{1020};
t7240 = ct{1021};
t7242 = ct{1022};
t7246 = ct{1023};
t7250 = ct{1024};
t7253 = ct{1025};
t7254 = ct{1026};
t7255 = ct{1027};
t7256 = ct{1028};
t7257 = ct{1029};
t7260 = ct{1030};
t7261 = ct{1031};
t7263 = ct{1032};
t7264 = ct{1033};
t7277 = ct{1034};
t7281 = ct{1035};
t7283 = ct{1036};
t7292 = ct{1037};
t7300 = ct{1038};
t7302 = ct{1039};
t7307 = ct{1040};
t7310 = ct{1041};
t7326 = ct{1042};
t7328 = ct{1043};
t7335 = ct{1044};
t7336 = ct{1045};
t7337 = ct{1046};
t7344 = ct{1047};
t7345 = ct{1048};
t7346 = ct{1049};
t7347 = ct{1050};
t7353 = ct{1051};
t7354 = ct{1052};
t7355 = ct{1053};
t7363 = ct{1054};
t7364 = ct{1055};
t7367 = ct{1056};
t7369 = ct{1057};
t7370 = ct{1058};
t7373 = ct{1059};
t7387 = ct{1060};
t7388 = ct{1061};
t7394 = ct{1062};
t7397 = ct{1063};
t7398 = ct{1064};
t7401 = ct{1065};
t7402 = ct{1066};
t7404 = ct{1067};
t7405 = ct{1068};
t7406 = ct{1069};
t7407 = ct{1070};
t7408 = ct{1071};
t7409 = ct{1072};
t7410 = ct{1073};
t7412 = ct{1074};
t7420 = ct{1075};
t7426 = ct{1076};
t7427 = ct{1077};
t7428 = ct{1078};
t7429 = ct{1079};
t7430 = ct{1080};
t7432 = ct{1081};
t7433 = ct{1082};
t7439 = ct{1083};
t7440 = ct{1084};
t7442 = ct{1085};
t7443 = ct{1086};
t7444 = ct{1087};
t7446 = ct{1088};
t7447 = ct{1089};
t7448 = ct{1090};
t7450 = ct{1091};
t7451 = ct{1092};
t7453 = ct{1093};
t7454 = ct{1094};
t7456 = ct{1095};
t7458 = ct{1096};
t7461 = ct{1097};
t7462 = ct{1098};
t7463 = ct{1099};
t7464 = ct{1100};
t7465 = ct{1101};
t7466 = ct{1102};
t7469 = ct{1103};
t7470 = ct{1104};
t7473 = ct{1105};
t7479 = ct{1106};
t7480 = ct{1107};
t7482 = ct{1108};
t7483 = ct{1109};
t7487 = ct{1110};
t7489 = ct{1111};
t749 = ct{1112};
t7496 = ct{1113};
t7498 = ct{1114};
t7501 = ct{1115};
t7502 = ct{1116};
t7505 = ct{1117};
t7507 = ct{1118};
t7508 = ct{1119};
t7509 = ct{1120};
t7510 = ct{1121};
t7511 = ct{1122};
t7512 = ct{1123};
t7514 = ct{1124};
t7516 = ct{1125};
t7518 = ct{1126};
t7519 = ct{1127};
t7523 = ct{1128};
t7524 = ct{1129};
t7529 = ct{1130};
t7530 = ct{1131};
t7542 = ct{1132};
t7544 = ct{1133};
t7545 = ct{1134};
t7546 = ct{1135};
t7548 = ct{1136};
t7549 = ct{1137};
t7550 = ct{1138};
t7551 = ct{1139};
t7552 = ct{1140};
t7553 = ct{1141};
t7554 = ct{1142};
t7557 = ct{1143};
t7559 = ct{1144};
t7560 = ct{1145};
t7561 = ct{1146};
t7562 = ct{1147};
t7563 = ct{1148};
t7564 = ct{1149};
t7565 = ct{1150};
t7566 = ct{1151};
t7567 = ct{1152};
t7568 = ct{1153};
t7575 = ct{1154};
t7577 = ct{1155};
t7579 = ct{1156};
t7582 = ct{1157};
t7583 = ct{1158};
t7584 = ct{1159};
t7585 = ct{1160};
t7586 = ct{1161};
t7587 = ct{1162};
t7589 = ct{1163};
t7612 = ct{1164};
t7614 = ct{1165};
t7616 = ct{1166};
t7618 = ct{1167};
t762 = ct{1168};
t7630 = ct{1169};
t7631 = ct{1170};
t7633 = ct{1171};
t7634 = ct{1172};
t7635 = ct{1173};
t7636 = ct{1174};
t7638 = ct{1175};
t7639 = ct{1176};
t7645 = ct{1177};
t7646 = ct{1178};
t7647 = ct{1179};
t7648 = ct{1180};
t7650 = ct{1181};
t7651 = ct{1182};
t7658 = ct{1183};
t7660 = ct{1184};
t7662 = ct{1185};
t7663 = ct{1186};
t7668 = ct{1187};
t7669 = ct{1188};
t7670 = ct{1189};
t7672 = ct{1190};
t7673 = ct{1191};
t7674 = ct{1192};
t7675 = ct{1193};
t7676 = ct{1194};
t7677 = ct{1195};
t7678 = ct{1196};
t7679 = ct{1197};
t768 = ct{1198};
t7680 = ct{1199};
t7682 = ct{1200};
t7683 = ct{1201};
t7684 = ct{1202};
t7686 = ct{1203};
t7687 = ct{1204};
t7688 = ct{1205};
t7690 = ct{1206};
t7691 = ct{1207};
t7692 = ct{1208};
t7694 = ct{1209};
t7695 = ct{1210};
t7696 = ct{1211};
t7697 = ct{1212};
t7698 = ct{1213};
t7699 = ct{1214};
t7701 = ct{1215};
t7704 = ct{1216};
t7707 = ct{1217};
t7710 = ct{1218};
t7711 = ct{1219};
t7712 = ct{1220};
t7713 = ct{1221};
t7714 = ct{1222};
t7715 = ct{1223};
t7716 = ct{1224};
t7718 = ct{1225};
t7719 = ct{1226};
t7720 = ct{1227};
t7721 = ct{1228};
t7723 = ct{1229};
t7726 = ct{1230};
t7727 = ct{1231};
t7730 = ct{1232};
t7732 = ct{1233};
t7734 = ct{1234};
t7736 = ct{1235};
t7737 = ct{1236};
t7738 = ct{1237};
t7740 = ct{1238};
t7741 = ct{1239};
t7744 = ct{1240};
t7745 = ct{1241};
t7746 = ct{1242};
t7748 = ct{1243};
t7751 = ct{1244};
t7752 = ct{1245};
t7753 = ct{1246};
t7755 = ct{1247};
t7756 = ct{1248};
t7759 = ct{1249};
t7760 = ct{1250};
t7762 = ct{1251};
t7763 = ct{1252};
t7764 = ct{1253};
t7765 = ct{1254};
t7766 = ct{1255};
t7768 = ct{1256};
t7769 = ct{1257};
t777 = ct{1258};
t7771 = ct{1259};
t7772 = ct{1260};
t7773 = ct{1261};
t7775 = ct{1262};
t7778 = ct{1263};
t7780 = ct{1264};
t7781 = ct{1265};
t7783 = ct{1266};
t7784 = ct{1267};
t7786 = ct{1268};
t7787 = ct{1269};
t7788 = ct{1270};
t7789 = ct{1271};
t7790 = ct{1272};
t7792 = ct{1273};
t7793 = ct{1274};
t7795 = ct{1275};
t7796 = ct{1276};
t7799 = ct{1277};
t7802 = ct{1278};
t7804 = ct{1279};
t7806 = ct{1280};
t7807 = ct{1281};
t7808 = ct{1282};
t7809 = ct{1283};
t7810 = ct{1284};
t7811 = ct{1285};
t7813 = ct{1286};
t7814 = ct{1287};
t7815 = ct{1288};
t7816 = ct{1289};
t7817 = ct{1290};
t7818 = ct{1291};
t7819 = ct{1292};
t7820 = ct{1293};
t7821 = ct{1294};
t7822 = ct{1295};
t7823 = ct{1296};
t7824 = ct{1297};
t7826 = ct{1298};
t7827 = ct{1299};
t7828 = ct{1300};
t7830 = ct{1301};
t7831 = ct{1302};
t7832 = ct{1303};
t7833 = ct{1304};
t7835 = ct{1305};
t7836 = ct{1306};
t7838 = ct{1307};
t7839 = ct{1308};
t7840 = ct{1309};
t7841 = ct{1310};
t7842 = ct{1311};
t7846 = ct{1312};
t7847 = ct{1313};
t7848 = ct{1314};
t7849 = ct{1315};
t7850 = ct{1316};
t7854 = ct{1317};
t7855 = ct{1318};
t7859 = ct{1319};
t7861 = ct{1320};
t7862 = ct{1321};
t7863 = ct{1322};
t7864 = ct{1323};
t7866 = ct{1324};
t7868 = ct{1325};
t7869 = ct{1326};
t7870 = ct{1327};
t7871 = ct{1328};
t7872 = ct{1329};
t7873 = ct{1330};
t7874 = ct{1331};
t7876 = ct{1332};
t7877 = ct{1333};
t7878 = ct{1334};
t7879 = ct{1335};
t7880 = ct{1336};
t7881 = ct{1337};
t7883 = ct{1338};
t7885 = ct{1339};
t7887 = ct{1340};
t7888 = ct{1341};
t7890 = ct{1342};
t7891 = ct{1343};
t7892 = ct{1344};
t7894 = ct{1345};
t7895 = ct{1346};
t7896 = ct{1347};
t7897 = ct{1348};
t7898 = ct{1349};
t7900 = ct{1350};
t7901 = ct{1351};
t7902 = ct{1352};
t7904 = ct{1353};
t7905 = ct{1354};
t7906 = ct{1355};
t7907 = ct{1356};
t7908 = ct{1357};
t7909 = ct{1358};
t7910 = ct{1359};
t7911 = ct{1360};
t7912 = ct{1361};
t7913 = ct{1362};
t7914 = ct{1363};
t7917 = ct{1364};
t7918 = ct{1365};
t7919 = ct{1366};
t792 = ct{1367};
t7920 = ct{1368};
t7921 = ct{1369};
t7922 = ct{1370};
t7923 = ct{1371};
t7924 = ct{1372};
t7925 = ct{1373};
t7926 = ct{1374};
t7927 = ct{1375};
t7928 = ct{1376};
t7929 = ct{1377};
t793 = ct{1378};
t7931 = ct{1379};
t7933 = ct{1380};
t7934 = ct{1381};
t7936 = ct{1382};
t7938 = ct{1383};
t7939 = ct{1384};
t7940 = ct{1385};
t7942 = ct{1386};
t7943 = ct{1387};
t7944 = ct{1388};
t7945 = ct{1389};
t7948 = ct{1390};
t7949 = ct{1391};
t7951 = ct{1392};
t7952 = ct{1393};
t7953 = ct{1394};
t7954 = ct{1395};
t7955 = ct{1396};
t7956 = ct{1397};
t7957 = ct{1398};
t7958 = ct{1399};
t7959 = ct{1400};
t7960 = ct{1401};
t7961 = ct{1402};
t7962 = ct{1403};
t7963 = ct{1404};
t7964 = ct{1405};
t7965 = ct{1406};
t7966 = ct{1407};
t7971 = ct{1408};
t7972 = ct{1409};
t7974 = ct{1410};
t7975 = ct{1411};
t7976 = ct{1412};
t7977 = ct{1413};
t7983 = ct{1414};
t7984 = ct{1415};
t7985 = ct{1416};
t7986 = ct{1417};
t7987 = ct{1418};
t7988 = ct{1419};
t8 = ct{1420};
t801 = ct{1421};
t802 = ct{1422};
t808 = ct{1423};
t813 = ct{1424};
t819 = ct{1425};
t821 = ct{1426};
t850 = ct{1427};
t855 = ct{1428};
t874 = ct{1429};
t878 = ct{1430};
t9 = ct{1431};
t941 = ct{1432};
t948 = ct{1433};
t951 = ct{1434};
et507 = t3910.*(et475+et476+et477).*(-1.0./2.0)+(t4879.*(t6979+t4019.*(t4795+t4801+t4808+t3976.*(t2694-t2701+t3036-t3043).*5.7e-7)+t6159.*(t1896-t3239)))./2.0-(t4008.*t4501)./2.0-(t4324.*t4326)./2.0-(t3910.*t7827)./2.0-(t3910.*t7940)./2.0+(t4879.*t7544)./2.0+(t3809.*(et478+et479+et480))./2.0;
et508 = ((t6287+t4031.*(t4795+t4801+t4808+t3976.*(t2694-t2701+t3036-t3043).*5.7e-7)+t4026.*(-t4494-t4495+t4799+t4823+t3976.*(t2694-t2701+t3036-t3043).*4.0e-8+t3980.*(t2694-t2701+t3036-t3043).*2.4e-7)).*(et481+et482))./2.0+(t3910.*(et483+et484+et485))./2.0;
et509 = (t3499.*(et486+et487+et488+et489+et490))./2.0+((t3237.*t5916+t3238.*t5917+(t50.*t202.*t5028.*(t46-t47))./8.112963841460668e+31).*(et491+et492))./2.0+((t2674-t2676+t3022-t3027).*(et493+et494+et495+et496))./2.0;
et510 = (t2674-t2676+t3022-t3027).*(t7101+t7402+t7458+t7658-t6159.*(t1005+t20.*(t1941-t3315+t39.*t1022.*(t855-t878).*2.196325630278387e-1))-t4874.*(t4795+t4801+t4808+t3976.*(t2694-t2701+t3036-t3043).*5.7e-7)).*(-1.0./2.0);
et511 = t4879.*(t3235.*t5917-t3236.*t5916+(t50.*t140.*t202.*t5028)./8.112963841460668e+31).*(-1.0./2.0)+(t7828.*(t2674-t2676+t3022-t3027))./2.0+(t7939.*(t2674-t2676+t3022-t3027))./2.0+(t7283.*(et497+et498))./2.0+(t7548.*(et499+et500))./2.0+(t4879.*(-t5523+t6054+t6004.*(t1896-t3239)))./2.0+t3934.*(et501+et502).*(t1488+t1874+t2519+t2740+t2747+t3096+t3097).*(t1513+t1879+t2598+t2820+t2834+t3117+t3118).*3.633675e-3;
et512 = t3499.*t3649.*(t2674-t2676+t3022-t3027).*(t2694-t2701+t3036-t3043).*(-1.444822e-2)-t3517.*t3638.*(t2674-t2676+t3022-t3027).*(t2694-t2701+t3036-t3043).*1.444822e-2+t3943.*t4172.*(t2674-t2676+t3022-t3027).*(t2694-t2701+t3036-t3043).*5.43845e-3;
et513 = t3924.*t4215.*(t2674-t2676+t3022-t3027).*(t2694-t2701+t3036-t3043).*5.43845e-3+t236.*t241.*t4563.*t4716.*2.156487945535858e-75;
et514 = t236.*t241.*t4652.*t4705.*(-2.156487945535858e-75)-t3499.*t3649.*t3910.*t3934.*1.444822e-2-t3517.*t3638.*t3910.*t3934.*1.444822e-2;
et515 = t3910.*t3934.*t3943.*t4172.*5.43845e-3+t3910.*t3924.*t3934.*t4215.*5.43845e-3-t3638.*t3649.*t3910.*t4915.*1.444822e-2-t3910.*t4172.*t4215.*t4915.*5.43845e-3;
et516 = t4352.*(t2674-t2676+t3022-t3027).*(t2694-t2701+t3036-t3043).*(t1488+t1874+t2519+t2740+t2747+t3096+t3097).*3.633675e-3+t4346.*(t2674-t2676+t3022-t3027).*(t2694-t2701+t3036-t3043).*(t1513+t1879+t2598+t2820+t2834+t3117+t3118).*3.633675e-3+t3910.*t3934.*t4352.*(t1488+t1874+t2519+t2740+t2747+t3096+t3097).*3.633675e-3;
et517 = t3910.*t3934.*t4346.*(t1513+t1879+t2598+t2820+t2834+t3117+t3118).*3.633675e-3-t3910.*t4915.*(t1488+t1874+t2519+t2740+t2747+t3096+t3097).*(t1513+t1879+t2598+t2820+t2834+t3117+t3118).*3.633675e-3+t3638.*t3649.*t4920.*(t2674-t2676+t3022-t3027).*1.444822e-2;
et518 = t3638.*t3649.*t4879.*(t2694-t2701+t3036-t3043).*1.444822e-2+t4172.*t4215.*t4920.*(t2674-t2676+t3022-t3027).*5.43845e-3+t4172.*t4215.*t4879.*(t2694-t2701+t3036-t3043).*5.43845e-3;
et519 = t4920.*(t2674-t2676+t3022-t3027).*(t1488+t1874+t2519+t2740+t2747+t3096+t3097).*(t1513+t1879+t2598+t2820+t2834+t3117+t3118).*3.633675e-3+t4879.*(t2694-t2701+t3036-t3043).*(t1488+t1874+t2519+t2740+t2747+t3096+t3097).*(t1513+t1879+t2598+t2820+t2834+t3117+t3118).*3.633675e-3+t3638.*t3649.*t3934.*(et503+et504).*1.444822e-2;
et520 = t3934.*t4172.*t4215.*(et505+et506).*5.43845e-3;
et521 = t7587-t7660+t7945+t7957-t7958-(t3047.*t7720)./2.0+(t3910.*t7826)./2.0+(t3980.*t7772)./2.0+(t3991.*t7773)./2.0+(t7631.*(t11.*((t237.*(t42-t43))./9.007199254740992e+15+t15.*(-t1881+t3121+t3276))+t16.*(-t1901+t3122+t3277)))./2.0;
et522 = (t7182-t7187+t4577.*(t3846-t5169-t5184+t5185+t3055.*(t2337+t12.*(t1456-t2355)).*9.3e-7+t4553.*(t3242-t3554).*9.3e-7)+t4573.*(t3840+t3862-t5164+t5167-t5183+t5189)).*(t2674-t2676+t3022-t3027).*(-1.0./2.0);
et523 = t5393+t5395+t7786-t7788+t4187.*(t2674-t2676+t3022-t3027).*(t2694-t2701+t3036-t3043).*(t1488+t1874+t2519+t2740+t2747+t3096+t3097).*3.633675e-3+t4146.*(t2674-t2676+t3022-t3027).*(t2694-t2701+t3036-t3043).*(t1513+t1879+t2598+t2820+t2834+t3117+t3118).*3.633675e-3+t3910.*t3934.*t4187.*(t1488+t1874+t2519+t2740+t2747+t3096+t3097).*3.633675e-3;
et524 = t3910.*t3934.*t4146.*(t1513+t1879+t2598+t2820+t2834+t3117+t3118).*3.633675e-3;
et525 = t4261+t4287+t4724+t4760-t5301-t5302-t5303-t5304+t5400+t5402-t5487-t5488-t5494-t5495+t7404-t7406+t7818-t7824+(t3910.*(t5637+t5773-t6685-t6910+t6911+t6490.*(t3563-t4051)))./2.0+(t7804.*(t2674-t2676+t3022-t3027))./2.0+t4018.*(t2674-t2676+t3022-t3027).*(t2694-t2701+t3036-t3043).*(t1488+t1874+t2519+t2740+t2747+t3096+t3097).*3.633675e-3;
et526 = t3975.*(t2674-t2676+t3022-t3027).*(t2694-t2701+t3036-t3043).*(t1513+t1879+t2598+t2820+t2834+t3117+t3118).*3.633675e-3+t3910.*t3934.*t4018.*(t1488+t1874+t2519+t2740+t2747+t3096+t3097).*3.633675e-3+t3910.*t3934.*t3975.*(t1513+t1879+t2598+t2820+t2834+t3117+t3118).*3.633675e-3;
et527 = t5080-t7199+t4853.*(t1005+t20.*(t1941-t3315+t39.*t1022.*(t855-t878).*2.196325630278387e-1)).*7.26735e-3;
et528 = t2419.*(t684+t685-t710+t724+t1686-t1690+t1700+t1701+t2371+t2698+t2707-t2716+t2719+t3329-t3337-t3351-t3641+t3643+t3655-t3659+t4114+t4115).*7.26735e-3;
et529 = t707+t708-t721-t722-t749+t762+t768-t777-t792-t793-t801-t802-t808+t813-t819+t821-t1629+t1637-t1640-t1641-t1659-t1661+t1666+t1667+t1683+t1692+t1705-t1712+t1758+t1759+t1775+t1776+t1973+t1993+t1994+t2023+t2053+t2060-t2089-t2090+t2098+t2099-t8.*t9.*t15.*t50.*t189.*3.670836568391568e-22;
et530 = t10.*t13.*t14.*t50.*t189.*(-3.279367663374749e-19)-t8.*t9.*t11.*t15.*t50.*t189.*7.075931802640439e-19;
et531 = t8.*t11.*t14.*t15.*t50.*t189.*(-1.190170786299927e-18)-t9.*t11.*t13.*t15.*t50.*t189.*1.190170786299927e-18;
et532 = t13.*t14.*t15.*t16.*t50.*t189.*(-3.226512155691387e-19);
et533 = -t4678+t4703-t5308-t5381+t5459+t5481-t5570-t5586-t5849+t6160+t6959-t7059-t7066+t7344+t7346+t7439+t7450-t7512+t7549+t7551+t7673-t7684+t7727+t7730+t7753+t7802-t7841-t7842+t7848+t7900+t7904+t7919-t7927+t7928+(t6647.*(et527+et528))./2.0;
et534 = (t7462.*(t4853.*(t1896-t3239).*7.26735e-3+t2363.*(t684+t685-t710+t724+t1686-t1690+t1700+t1701+t2371+t2698+t2707-t2716+t2719+t3329-t3337-t3351-t3641+t3643+t3655-t3659+t4114+t4115).*7.26735e-3))./2.0;
et535 = (t3910.*(t6263-t6887+t6888-t7355+t7307.*(t3563-t4051)+t21.*t3547.*(-t3434+t4606+t3980.*(t1896-t3239).*1.02e-6)))./2.0+(t3216.*(-t5828-t5829+t6593+t6596+t22.*t6699.*(t3242-t3554)+t28.*t6696.*(t3242-t3554)))./2.0;
et536 = (t3915.*(t6872+t6058.*(t1896-t3239)+t4019.*(t3435-t3448+t4615+t4619+t3976.*(t1896-t3239).*5.7e-7+t3980.*(t1896-t3239).*4.0e-8)))./2.0;
et537 = (t3217.*(t6251-t6997-t7310+t7388+t7554+t4880.*(t3435-t3448+t4615+t4619+t3976.*(t1896-t3239).*5.7e-7+t3980.*(t1896-t3239).*4.0e-8)))./2.0+t4215.*t5279.*(t2694-t2701+t3036-t3043).*5.43845e-3;
et538 = t3810.*t6011.*(t2694-t2701+t3036-t3043).*5.43845e-3+t3951.*t6647.*(t2694-t2701+t3036-t3043).*3.633675e-3+t3810.*t3934.*(et529+et530+et531+et532).*5.43845e-3+t3934.*t5771.*(t1513+t1879+t2598+t2820+t2834+t3117+t3118).*3.633675e-3;
et539 = t50.*t189.*(t5618+t6429-t6902+t3055.*(t4795+t4801+t4808+t3976.*(t2694-t2701+t3036-t3043).*5.7e-7)+t6384.*(t1477-t2502)).*4.771516396025243e-17;
et540 = t5296-t5439-t6305+t7080+t7084+t7575+t7577-t7579+t7775+t7811-t7813-t7907+t7934-t7936+(t2994.*(-t6772+t6776+t3055.*(-t3434+t4606+t3980.*(t1896-t3239).*1.02e-6)))./2.0+(t7461.*(t1456-t2355))./2.0+(t7524.*(t11.*((t237.*(t42-t43))./9.007199254740992e+15+t15.*(-t1881+t3121+t3276))+t16.*(-t1901+t3122+t3277)))./2.0+(t7755.*(t2674-t2676+t3022-t3027))./2.0;
et541 = (t3047.*(t6462-t6464-t6766-t6767+t3055.*(t4809+t3976.*(t2694-t2701+t3036-t3043).*1.02e-6)+t5572.*(t1477-t2502)))./2.0;
et542 = ((t4673+t2363.*(t3566.*1.838876e-2+t4109-t4110+t28.*(t1896-t3239).*9.99471e-3).*7.26735e-3).*(t2674-t2676+t3022-t3027).*(t1488+t1874+t2519+t2740+t2747+t3096+t3097))./2.0;
et543 = -t5344-t5568+t5679+t5689+t5925+t5927-t5966+t5976+t5980-t6241+t6295+t6367+t6528+t6540+t7028+t7031-t7040+t7300+t7302-t7363+t7612+t7616;
et544 = (t4118.*(t4573.*(t2813-t2835+t12.*(t1456-t2355).*1.02e-6+t17.*(t1456-t2355).*9.0e-8)+t4577.*(-t2804+t2838+t3109+t17.*(t1456-t2355).*9.3e-7)+t3133.*(t3242-t3554)))./2.0;
et545 = (t6651.*(t4814.*(t1861-t3221)+t2297.*(t642+t643-t667+t674+t1587+t1606+t1608+t1609+t2295+t2671+t2683+t2684-t2695+t3279+t3297-t3303+t3597+t3603+t3609-t3614+t4053+t4054)))./2.0+(t5809.*(t951+t10.*(-t1881+t3121+t3276)))./2.0+((t1861-t3221).*(t4658+t4719+t5240+t5262-t3483.*(t1005+t20.*(t1941-t3315+t39.*t1022.*(t855-t878).*2.196325630278387e-1))-t3431.*(t1896-t3239)))./2.0+(t3808.*t5645.*(t2674-t2676+t3022-t3027))./2.0;
et546 = (t3925.*t5946.*(t2674-t2676+t3022-t3027))./2.0;
et547 = -t5344-t5568+t5679+t5689+t5925+t5927-t5966+t5978+t5980-t6241+t6299+t6367+t6528+t6540+t7028+t7031-t7040+t7300+t7302-t7363+t7614+t7618;
et548 = (t4118.*(t4573.*(t2813-t2835+t12.*(t1456-t2355).*1.02e-6+t17.*(t1456-t2355).*9.0e-8)+t4577.*(-t2804+t2838+t3109+t17.*(t1456-t2355).*9.3e-7)+t3133.*(t3242-t3554)))./2.0;
et549 = (t6651.*(t4814.*(t1861-t3221)+t2297.*(t642+t643-t667+t674+t1587+t1606+t1608+t1609+t2295+t2671+t2683+t2684-t2695+t3279+t3297-t3303+t3597+t3603+t3609-t3614+t4053+t4054)))./2.0+(t5809.*(t951+t10.*(-t1881+t3121+t3276)))./2.0+((t1861-t3221).*(t4658+t4719+t5240+t5262-t3483.*(t1005+t20.*(t1941-t3315+t39.*t1022.*(t855-t878).*2.196325630278387e-1))-t3431.*(t1896-t3239)))./2.0+(t3808.*t5646.*(t2674-t2676+t3022-t3027))./2.0;
et550 = (t3925.*t5949.*(t2674-t2676+t3022-t3027))./2.0;
et551 = -t32.*(et451+et452+et453+et454+et455+et456+et457+et458+et459+et460)-t33.*(et464+et465+et466+et467+et468+et469+et470+et471+et472+et473+et474)+t29.*t7966+t30.*t7965+t31.*(et507+et508+et509+et510+et511+et512+et513+et514+et515+et516+et517+et518+et519+et520)-t34.*(et521+et522)+dq4.*dq6.*(t5399+t5545+t6250+t6261+t7000+t7001+t7430-t7466+t7529+t7530+t7566+t7744+t7745+t7764-t7821+t7879+t7917+t7918+(t3991.*(t5637+t5773-t6685-t6910+t6911+t6490.*(t3563-t4051)))./2.0+(t11.*t7544.*(t1861-t3221))./2.0)-dq4.*dq5.*(t4559+t4713+t5283+t5392+t5458+t5499+t5569+t5607+t5954+t5955+t6172+t6178+t6564+t6565+t6983+t6989+t7011+t7013+t7335+t7336+t7409+t7428+t7447+t7448+t7465+t7482+t7509+t7510+t7561+t7562+t7563+t7567+t7676+t7677+t7679+t7680+t7695+t7696+t7760+t7762+t7763+t7793+t7806+t7808+t7815+t7817+t7869+t7877+t7897+t7898+t7913+t7914);
et552 = -dq5.*dq6.*(t5309+t5438+t6275+t6278+t7019+t7027+t7586+t7650+t7651+t7723+t7781+t7783+t7888+t7890+t7944+t7955+t7956)+dq3.*dq6.*(et523+et524).*2.0+dq3.*dq4.*(et525+et526).*2.0+dq4.*dq6.*(t5404+t5544+t6228+t6230+t6971+t6975+t7583+t7645+t7646+t7721+t7778+t7780+t7871+t7943+t7953+t7954+(t7862.*(t2674-t2676+t3022-t3027))./2.0)-dq4.*dq5.*(et533+et534+et535+et536+et537+et538+et539)-dq1.*dq6.*t7948-dq2.*dq6.*t7949+dq1.*dq2.*t7975-dq1.*dq6.*t7971+dq1.*dq2.*t7976-dq2.*dq6.*t7972-dq1.*dq4.*t7983-dq2.*dq4.*t7984-dq1.*dq5.*t7985-dq1.*dq4.*t7987-dq2.*dq5.*t7986-dq2.*dq4.*t7988+dq5.*dq6.*(et540+et541+et542)-dq3.*dq5.*(t4722+t4741+t5361+t5363+t5535+t5536+t5538+t5539+t5730+t5731+t5734+t5735+t7736+t7738+t7809+t7810).*2.0+dq1.*dq5.*(et543+et544+et545+et546)+dq2.*dq5.*(et547+et548+et549+et550);
et553 = t7585+t7634-t7636-t7873-t7874+(t3047.*(t5816-t6360-t7032+t7033+t7367-t7369))./2.0+(t3047.*t7698)./2.0-(t3217.*t7826)./2.0+(t3980.*t7726)./2.0+(t3216.*(t7182-t7187+t4577.*(t3846-t5169-t5184+t5185+t3055.*(t2337+t12.*(t1456-t2355)).*9.3e-7+t4553.*(t3242-t3554).*9.3e-7)+t4573.*(t3840+t3862-t5164+t5167-t5183+t5189)))./2.0;
et554 = t3991.*(-t6848+t6852+t6584.*(t3563-t4051)+t6585.*(t3563-t4051)).*(-1.0./2.0)+t50.*t189.*t7796.*4.771516396025243e-17;
et555 = t6413+t7401+t4880.*(t4795+t4801+t4808+t3976.*(t2694-t2701+t3036-t3043).*5.7e-7)+t4031.*(t5287+t5291-t5328+t5333+t5337-t5340+t4835.*(t2694-t2701+t3036-t3043).*5.7e-7+t4838.*(t2694-t2701+t3036-t3043).*4.0e-8);
et556 = t4026.*(-t5202+t5286+t5297+t5331-t5332-t5336+t5341+(t4920.*(t1861-t3221))./1.0e+8+(t3934.*(t951+t10.*(-t1881+t3121+t3276)))./1.0e+8+(t4118.*(t2694-t2701+t3036-t3043))./1.0e+8+t4835.*(t2694-t2701+t3036-t3043).*4.0e-8+t4838.*(t2694-t2701+t3036-t3043).*2.4e-7);
et557 = t4872.*(-t4494-t4495+t4799+t4823+t3976.*(t2694-t2701+t3036-t3043).*4.0e-8+t3980.*(t2694-t2701+t3036-t3043).*2.4e-7);
et558 = t3015-t3068+t4470-t4518+t3500.*(t1959-t3313+t38.*t1022.*(t855-t878).*2.196325630278387e-1).*9.840000000000001e-6;
et559 = t3237.*((t237.*(t42-t43))./9.007199254740992e+15+t15.*(-t1881+t3121+t3276)).*9.840000000000001e-6;
et560 = (t2674-t2676+t3022-t3027).*(-t6510+t7364+t7483+t5918.*(t1005+t20.*(t1941-t3315+t39.*t1022.*(t855-t878).*2.196325630278387e-1))+t6549.*(t4165+t27.*(t1959-t3313+t38.*t1022.*(t855-t878).*2.196325630278387e-1))+t7277.*(t1896-t3239));
et561 = -1.0./2.0;
et562 = -t2306-t2317+t3145+t3148+t35.*t941.*t948.*(t850-t874).*3.775747223193135e-1;
et563 = t36.*t941.*t948.*(t850-t874).*2.244797987218524e-1;
et564 = -t2306-t2317+t3145+t3148+t35.*t941.*t948.*(t850-t874).*3.775747223193135e-1;
et565 = t36.*t941.*t948.*(t850-t874).*2.244797987218524e-1;
et566 = -t2306-t2317+t3145+t3148+t35.*t941.*t948.*(t850-t874).*3.775747223193135e-1;
et567 = t36.*t941.*t948.*(t850-t874).*2.244797987218524e-1;
et568 = -t2306-t2317+t3145+t3148+t35.*t941.*t948.*(t850-t874).*3.775747223193135e-1;
et569 = t36.*t941.*t948.*(t850-t874).*2.244797987218524e-1;
et570 = t4746-t5085+t5091-t5214+t4920.*(t1861-t3221).*7.83e-6+t3934.*(t951+t10.*(-t1881+t3121+t3276)).*7.83e-6+t4118.*(t2694-t2701+t3036-t3043).*7.83e-6;
et571 = t3934.*(-t1901+t3122+t3277).*3.24e-6;
et572 = t4751-t5086+t5093-t5213+t4920.*(t1861-t3221).*3.24e-6+t3934.*(t951+t10.*(-t1881+t3121+t3276)).*3.24e-6+t4118.*(t2694-t2701+t3036-t3043).*3.24e-6;
et573 = t3934.*(-t1901+t3122+t3277).*3.11e-6;
et574 = -t2306-t2317+t3145+t3148+t35.*t941.*t948.*(t850-t874).*3.775747223193135e-1;
et575 = t36.*t941.*t948.*(t850-t874).*2.244797987218524e-1;
et576 = t1288+t1289+t1302+t1303-t1319-t1320+t1336-t1348+t1350+t1351-t1360+t1369-t1378+t1396-t1425+t1435-t2174+t2183-t2187+t2193-t2194-t2195+t2199-t2203-t2215+t2219-t2222-t2223+t2239+t2240-t2256-t2257+t2555+t2556+t2572+t2583-t2605-t2606+t2612+t2613-t2618-t2619+t2651+t2652;
et577 = t18.*t19.*t20.*t50.*t202.*(-3.566935413776081e-21);
et578 = t24.*t25.*t26.*t50.*t202.*(-3.992732227073824e-24);
et579 = t18.*t19.*t26.*t27.*t50.*t202.*(-3.509445006623964e-21);
et580 = t21.*t24.*t25.*t26.*t50.*t202.*(-7.696420262413979e-21);
et581 = t707+t708-t721-t722-t749+t762+t768-t777-t792-t793-t801-t802-t808+t813-t819+t821-t1629+t1637-t1640-t1641-t1659-t1661+t1666+t1667+t1683+t1692+t1705-t1712+t1758+t1759+t1775+t1776+t1973+t1993+t1994+t2023+t2053+t2060-t2089-t2090+t2098+t2099-t8.*t9.*t15.*t50.*t189.*3.670836568391568e-22;
et582 = t10.*t13.*t14.*t50.*t189.*(-3.279367663374749e-19)-t8.*t9.*t11.*t15.*t50.*t189.*7.075931802640439e-19;
et583 = t8.*t11.*t14.*t15.*t50.*t189.*(-1.190170786299927e-18)-t9.*t11.*t13.*t15.*t50.*t189.*1.190170786299927e-18;
et584 = t13.*t14.*t15.*t16.*t50.*t189.*(-3.226512155691387e-19);
et585 = t707+t708-t721-t722-t749+t762+t768-t777-t792-t793-t801-t802-t808+t813-t819+t821-t1629+t1637-t1640-t1641-t1659-t1661+t1666+t1667+t1683+t1692+t1705-t1712+t1758+t1759+t1775+t1776+t1973+t1993+t1994+t2023+t2053+t2060-t2089-t2090+t2098+t2099-t8.*t9.*t15.*t50.*t189.*3.670836568391568e-22;
et586 = t10.*t13.*t14.*t50.*t189.*(-3.279367663374749e-19)-t8.*t9.*t11.*t15.*t50.*t189.*7.075931802640439e-19;
et587 = t8.*t11.*t14.*t15.*t50.*t189.*(-1.190170786299927e-18)-t9.*t11.*t13.*t15.*t50.*t189.*1.190170786299927e-18;
et588 = t13.*t14.*t15.*t16.*t50.*t189.*(-3.226512155691387e-19);
et589 = t1288+t1289+t1302+t1303-t1319-t1320+t1336-t1348+t1350+t1351-t1360+t1369-t1378+t1396-t1425+t1435-t2174+t2183-t2187+t2193-t2194-t2195+t2199-t2203-t2215+t2219-t2222-t2223+t2239+t2240-t2256-t2257+t2555+t2556+t2572+t2583-t2605-t2606+t2612+t2613-t2618-t2619+t2651+t2652;
et590 = t18.*t19.*t20.*t50.*t202.*(-3.566935413776081e-21);
et591 = t24.*t25.*t26.*t50.*t202.*(-3.992732227073824e-24);
et592 = t18.*t19.*t26.*t27.*t50.*t202.*(-3.509445006623964e-21);
et593 = t21.*t24.*t25.*t26.*t50.*t202.*(-7.696420262413979e-21);
et594 = t4263+t4288+t4725+t4761+t5301+t5302+t5303+t5304+t5401+t5403+t5487+t5488+t5494+t5495+t5738+t5739+t5741+t5742+t7405+t7406+t7819+t7820+t7823+t7824-(t3217.*(et555+et556+et557))./2.0-((t2674-t2676+t3022-t3027).*(t5425+t5886+t7134+t5699.*(t1959-t3313+t38.*t1022.*(t855-t878).*2.196325630278387e-1)+t7088.*(t1896-t3239)+t3543.*(et558+et559)))./2.0;
et595 = t3216.*(t7101+t7402+t7458+t7658-t6159.*(t1005+t20.*(t1941-t3315+t39.*t1022.*(t855-t878).*2.196325630278387e-1))-t4874.*(t4795+t4801+t4808+t3976.*(t2694-t2701+t3036-t3043).*5.7e-7)).*(-1.0./2.0);
et596 = t188.*(t2388.*t5346-t2363.*t6004+t50.*t202.*t6005.*9.543032792050485e-17).*4.297799892626299e-1-(t3915.*(t6979+t4019.*(t4795+t4801+t4808+t3976.*(t2694-t2701+t3036-t3043).*5.7e-7)+t6159.*(t1896-t3239)))./2.0;
et597 = t188.*t7461.*4.297799892626299e-1-(t3903.*t4324)./2.0-(t4008.*t4275)./2.0+(t3901.*t4501)./2.0+(t4274.*t4326)./2.0+(t3216.*t7828)./2.0-(t3217.*t7827)./2.0+(t3216.*t7939)./2.0-(t3217.*t7940)./2.0-(t3915.*t7544)./2.0-(t3910.*t7784)./2.0-(t3910.*t7894)./2.0-(t3910.*t7909)./2.0+(t4879.*t7432)./2.0+(t4879.*t7469)./2.0;
et598 = ((-t1901+t3122+t3277).*(t6287+t4031.*(t4795+t4801+t4808+t3976.*(t2694-t2701+t3036-t3043).*5.7e-7)+t4026.*(-t4494-t4495+t4799+t4823+t3976.*(t2694-t2701+t3036-t3043).*4.0e-8+t3980.*(t2694-t2701+t3036-t3043).*2.4e-7)))./2.0;
et599 = t188.*(-t6196+t6428+t3055.*(-t4494-t4495+t4799+t4823+t3976.*(t2694-t2701+t3036-t3043).*4.0e-8+t3980.*(t2694-t2701+t3036-t3043).*2.4e-7)).*4.297799892626299e-1-(t7908.*(t2674-t2676+t3022-t3027))./2.0+et560.*et561+(t7283.*(-t1901+t3122+t3277))./2.0;
et600 = (t7548.*(-t1901+t3122+t3277))./2.0+(t7083.*(et562+et563))./2.0+(t7433.*(et564+et565))./2.0+(t7470.*(et566+et567))./2.0-(t3915.*(-t5523+t6054+t6004.*(t1896-t3239)))./2.0+(t4879.*(-t5264+t5804+t5698.*(t1896-t3239)))./2.0+t3943.*t6011.*(t2694-t2701+t3036-t3043).*5.43845e-3-t4215.*t5782.*(t2694-t2701+t3036-t3043).*5.43845e-3-(t4172.*t5901.*(t2674-t2676+t3022-t3027))./2.0;
et601 = (t3924.*t6255.*(t2674-t2676+t3022-t3027))./2.0+(t4346.*t6682.*(t2674-t2676+t3022-t3027))./2.0+t4352.*t6647.*(t2694-t2701+t3036-t3043).*3.633675e-3+(t7473.*(t2674-t2676+t3022-t3027).*(t1488+t1874+t2519+t2740+t2747+t3096+t3097))./2.0+t7462.*(t2694-t2701+t3036-t3043).*(t1513+t1879+t2598+t2820+t2834+t3117+t3118).*3.633675e-3+(t3910.*(t5034-t5280-t6302+t7166).*(t1488+t1874+t2519+t2740+t2747+t3096+t3097))./2.0;
et602 = (t6689.*(et568+et569).*(t1488+t1874+t2519+t2740+t2747+t3096+t3097))./2.0-t50.*t189.*(t201.*t6005.*(-8.595599785252598e-1)+t2399.*t5346+t2419.*t6004+t2388.*t6589+t2363.*(et570+et571)-t50.*t202.*(et572+et573).*9.543032792050485e-17).*4.771516396025243e-17-(t4172.*(et574+et575).*(et576+et577+et578+et579+et580))./2.0;
et603 = t3934.*t3943.*(et581+et582+et583+et584).*5.43845e-3-t4215.*t4915.*(et585+et586+et587+et588).*5.43845e-3+t50.*t189.*t7924.*4.771516396025243e-17-t50.*t189.*t7938.*4.771516396025243e-17;
et604 = t3934.*t4215.*t5783.*(-5.43845e-3)-(t3910.*t4172.*t5902)./2.0+t3934.*t4352.*t6650.*3.633675e-3+(t3910.*t4346.*t6689)./2.0+t4215.*t4920.*t6011.*5.43845e-3+(t4172.*t4879.*t6255)./2.0+(t4879.*t6682.*(t1488+t1874+t2519+t2740+t2747+t3096+t3097))./2.0;
et605 = t3934.*t7463.*(t1513+t1879+t2598+t2820+t2834+t3117+t3118).*3.633675e-3-t4915.*t6650.*(t1513+t1879+t2598+t2820+t2834+t3117+t3118).*3.633675e-3+t4920.*t6647.*(t1513+t1879+t2598+t2820+t2834+t3117+t3118).*3.633675e-3-(t3910.*t3924.*(et589+et590+et591+et592+et593))./2.0;
et606 = t236.*t241.*t4683.*t4716.*1.16903445774439e-94;
et607 = t236.*t241.*t4705.*t4709.*(-1.16903445774439e-94);
et608 = t236.*t241.*t4563.*t5036.*1.16903445774439e-94;
et609 = t236.*t241.*t4652.*t5025.*(-1.16903445774439e-94);
et610 = t5793+t5796+t4577.*(t4618+t4634-t12.*t2363.*t3047.*9.0e-8-t17.*t2363.*t3047.*9.3e-7+t12.*t3980.*(t1896-t3239).*9.0e-8+t17.*t3980.*(t1896-t3239).*9.3e-7);
et611 = t4573.*(t4617+t4635-t12.*t2363.*t3047.*1.02e-6-t17.*t2363.*t3047.*9.0e-8+t12.*t3980.*(t1896-t3239).*1.02e-6+t17.*t3980.*(t1896-t3239).*9.0e-8);
et612 = t22.*t6675.*(t3242-t3554)+t28.*t6674.*(t3242-t3554);
et613 = t5580+t5581+t6376-t6724-t6725;
et614 = t3395.*(t4618+t4634-t12.*t2363.*t3047.*9.0e-8-t17.*t2363.*t3047.*9.3e-7+t12.*t3980.*(t1896-t3239).*9.0e-8+t17.*t3980.*(t1896-t3239).*9.3e-7);
et615 = t5433+t5434+t7442+t7454+t7487+t7489+t7501+t7507+t7514+t7516+t7542+t7545+t7830+t7832+t7839+t7840+t7846+t7847+(t2297.*(t5490+t6190-t6193-t6609-t6610+t5405.*(t1477-t2502)))./2.0-(t3502.*(t5713+t5714-t6443-t6719-t6722+t6102.*(t3563-t4051)))./2.0+((t1861-t3221).*(t6326-t6665+t5382.*(t1896-t3239)+t6098.*(t3242-t3554)+t6100.*(t3242-t3554)))./2.0;
et616 = (t6647.*(t4371.*(t1896-t3239).*7.26735e-3+t2363.*(t3328+t3344+t3642-t3658+t22.*(t3242-t3554).*1.838876e-2+t28.*(t3242-t3554).*9.99471e-3).*7.26735e-3))./2.0;
et617 = t5767.*(t4853.*(t1896-t3239).*7.26735e-3+t2363.*(t684+t685-t710+t724+t1686-t1690+t1700+t1701+t2371+t2698+t2707-t2716+t2719+t3329-t3337-t3351-t3641+t3643+t3655-t3659+t4114+t4115).*7.26735e-3).*(-1.0./2.0)-(t2297.*t7638)./2.0+(t3216.*t7704)./2.0-(t3217.*t7795)./2.0+(t3502.*t7682)./2.0-(t5791.*t6711)./2.0-(t5771.*t6793)./2.0+(t6064.*t6650)./2.0+(t6039.*t6682)./2.0+(t6041.*t6689)./2.0;
et618 = t5790.*(t4814.*(t1861-t3221)+t2297.*(t642+t643-t667+t674+t1587+t1606+t1608+t1609+t2295+t2671+t2683+t2684-t2695+t3279+t3297-t3303+t3597+t3603+t3609-t3614+t4053+t4054)).*(-1.0./2.0)+(t3217.*(t5669-t6476-t6478+t6875+t4026.*(t3435-t3448+t4615+t4619+t3976.*(t1896-t3239).*5.7e-7+t3980.*(t1896-t3239).*4.0e-8)))./2.0+(t7746.*(t1861-t3221))./2.0+(t3216.*(et610+et611+et612))./2.0;
et619 = t50.*t189.*(et613+et614).*(-4.771516396025243e-17)-t50.*t189.*t7688.*4.771516396025243e-17;
et620 = t236.*t241.*t4035.*t4763.*(-1.297888971568006e-110);
et621 = t236.*t241.*t3974.*t4850.*(-1.297888971568006e-110);
et622 = t236.*t241.*t4762.*t5036.*1.297888971568006e-110;
et623 = t236.*t241.*t4847.*t5025.*1.297888971568006e-110;
et624 = t707+t708-t721-t722-t749+t762+t768-t777-t792-t793-t801-t802-t808+t813-t819+t821-t1629+t1637-t1640-t1641-t1659-t1661+t1666+t1667+t1683+t1692+t1705-t1712+t1758+t1759+t1775+t1776+t1973+t1993+t1994+t2023+t2053+t2060-t2089-t2090+t2098+t2099-t8.*t9.*t15.*t50.*t189.*3.670836568391568e-22;
et625 = t10.*t13.*t14.*t50.*t189.*(-3.279367663374749e-19)-t8.*t9.*t11.*t15.*t50.*t189.*7.075931802640439e-19;
et626 = t8.*t11.*t14.*t15.*t50.*t189.*(-1.190170786299927e-18)-t9.*t11.*t13.*t15.*t50.*t189.*1.190170786299927e-18;
et627 = t13.*t14.*t15.*t16.*t50.*t189.*(-3.226512155691387e-19);
et628 = t1288+t1289+t1302+t1303-t1319-t1320+t1336-t1348+t1350+t1351-t1360+t1369-t1378+t1396-t1425+t1435-t2174+t2183-t2187+t2193-t2194-t2195+t2199-t2203-t2215+t2219-t2222-t2223+t2239+t2240-t2256-t2257+t2555+t2556+t2572+t2583-t2605-t2606+t2612+t2613-t2618-t2619+t2651+t2652;
et629 = t18.*t19.*t20.*t50.*t202.*(-3.566935413776081e-21);
et630 = t24.*t25.*t26.*t50.*t202.*(-3.992732227073824e-24);
et631 = t18.*t19.*t26.*t27.*t50.*t202.*(-3.509445006623964e-21);
et632 = t21.*t24.*t25.*t26.*t50.*t202.*(-7.696420262413979e-21);
et633 = t6257.*(et624+et625+et626+et627).*(-1.0./2.0)-(t3217.*(t5411-t5563+t6762-t6765+t4604.*(t3428-t3432-t4570+t4576+t4582-t4603)+t6244.*(t3563-t4051)))./2.0+(t3901.*t4273)./2.0+(t3902.*t4274)./2.0-(t3217.*t7281)./2.0-(t3216.*t7715)./2.0+(t3217.*t7716)./2.0+(t3216.*t7748)./2.0-(t6011.*t6256)./2.0-(t6013.*t6255)./2.0+(t6059.*t6647)./2.0+(t6060.*t6650)./2.0+(t6031.*t6682)./2.0+(t6032.*t6689)./2.0+(t6014.*(et628+et629+et630+et631+et632))./2.0;
et634 = t3216.*(t5243+t5265-t5821+t3543.*(-t3064+t4065+t3236.*(t1861-t3221).*9.840000000000001e-6)+t5043.*(t1896-t3239)).*(-1.0./2.0);
et635 = t50.*t189.*(-t2388.*(-t3064+t4065+t3236.*(t1861-t3221).*9.840000000000001e-6)+t2363.*t5041-t2363.*t5043+t2388.*t5698+t50.*t202.*t5042.*9.543032792050485e-17).*(-4.771516396025243e-17);
et636 = t50.*t189.*(-t5453+t6371-t6616+t6617+t3395.*(t3428-t3432-t4570+t4576+t4582-t4603)+t3055.*(-t3080+t4100+t11.*t3236.*(t1861-t3221).*1.02e-6)).*4.771516396025243e-17+t50.*t189.*t7697.*4.771516396025243e-17;
et637 = t236.*t241.*t5025.*t5037.*6.337348493984406e-114;
et638 = t236.*t241.*t5027.*t5036.*6.337348493984406e-114;
et639 = t3582.*1.33637554986e-4+t3716-t3717+t27.*(t1896-t3239).*4.36041e-5;
et640 = t27.*t28.*(t1896-t3239).*7.26350557185e-5;
et641 = t707+t708-t721-t722-t749+t762+t768-t777-t792-t793-t801-t802-t808+t813-t819+t821-t1629+t1637-t1640-t1641-t1659-t1661+t1666+t1667+t1683+t1692+t1705-t1712+t1758+t1759+t1775+t1776+t1973+t1993+t1994+t2023+t2053+t2060-t2089-t2090+t2098+t2099-t8.*t9.*t15.*t50.*t189.*3.670836568391568e-22;
et642 = t10.*t13.*t14.*t50.*t189.*(-3.279367663374749e-19)-t8.*t9.*t11.*t15.*t50.*t189.*7.075931802640439e-19;
et643 = t8.*t11.*t14.*t15.*t50.*t189.*(-1.190170786299927e-18)-t9.*t11.*t13.*t15.*t50.*t189.*1.190170786299927e-18;
et644 = t13.*t14.*t15.*t16.*t50.*t189.*(-3.226512155691387e-19);
et645 = t707+t708-t721-t722-t749+t762+t768-t777-t792-t793-t801-t802-t808+t813-t819+t821-t1629+t1637-t1640-t1641-t1659-t1661+t1666+t1667+t1683+t1692+t1705-t1712+t1758+t1759+t1775+t1776+t1973+t1993+t1994+t2023+t2053+t2060-t2089-t2090+t2098+t2099-t8.*t9.*t15.*t50.*t189.*3.670836568391568e-22;
et646 = t10.*t13.*t14.*t50.*t189.*(-3.279367663374749e-19)-t8.*t9.*t11.*t15.*t50.*t189.*7.075931802640439e-19;
et647 = t8.*t11.*t14.*t15.*t50.*t189.*(-1.190170786299927e-18)-t9.*t11.*t13.*t15.*t50.*t189.*1.190170786299927e-18;
et648 = t13.*t14.*t15.*t16.*t50.*t189.*(-3.226512155691387e-19);
et649 = (t4843+t5108+t2307.*(t642+t643-t667+t674+t1587+t1606+t1608+t1609+t2295+t2671+t2683+t2684-t2695+t3279+t3297-t3303+t3597+t3603+t3609-t3614+t4053+t4054)+t2297.*(t2292+t3290+t3524.*1.838876e-2-t3591+t3592+t3611+t16.*(t1861-t3221).*3.131399999999998e-4+t16.*t17.*(t1861-t3221).*9.99471e-3)).*(t2694-t2701+t3036-t3043).*(t1513+t1879+t2598+t2820+t2834+t3117+t3118);
et650 = 3.633675e-3;
et651 = -t4678+t4703-t5308+t5391-t5458+t5481-t5569+t5604-t5849+t6160+t6959+t7010+t7012-t7336-t7409-t7428+t7446+t7464+t7508+t7560-t7563+t7565+t7675-t7677+t7678-t7680+t7727+t7730+t7753+t7759+t7792+t7802+t7807+t7814+t7816-t7869-t7877-t7897-t7898+t7912-t7914;
et652 = (t2307.*(-t6196+t6428+t3055.*(-t4494-t4495+t4799+t4823+t3976.*(t2694-t2701+t3036-t3043).*4.0e-8+t3980.*(t2694-t2701+t3036-t3043).*2.4e-7)))./2.0+(t7799.*(t1861-t3221))./2.0+(t7433.*(t951+t10.*(-t1881+t3121+t3276)))./2.0+(t7470.*(t951+t10.*(-t1881+t3121+t3276)))./2.0;
et653 = (t3216.*(-t5828-t5829+t6593+t6596+t22.*t6699.*(t3242-t3554)+t28.*t6696.*(t3242-t3554)))./2.0;
et654 = (t3503.*(t6287+t4031.*(t4795+t4801+t4808+t3976.*(t2694-t2701+t3036-t3043).*5.7e-7)+t4026.*(-t4494-t4495+t4799+t4823+t3976.*(t2694-t2701+t3036-t3043).*4.0e-8+t3980.*(t2694-t2701+t3036-t3043).*2.4e-7)))./2.0;
et655 = t4215.*t5279.*(t2694-t2701+t3036-t3043).*5.43845e-3+t3810.*t6011.*(t2694-t2701+t3036-t3043).*5.43845e-3+t3951.*t6647.*(t2694-t2701+t3036-t3043).*3.633675e-3+t3810.*t3934.*(et645+et646+et647+et648).*5.43845e-3+et649.*et650;
et656 = t3934.*t5771.*(t1513+t1879+t2598+t2820+t2834+t3117+t3118).*3.633675e-3+t50.*t189.*(t5618+t6429-t6902+t3055.*(t4795+t4801+t4808+t3976.*(t2694-t2701+t3036-t3043).*5.7e-7)+t6384.*(t1477-t2502)).*4.771516396025243e-17;
et657 = t1288+t1289+t1302+t1303-t1319-t1320+t1336-t1348+t1350+t1351-t1360+t1369-t1378+t1396-t1425+t1435-t2174+t2183-t2187+t2193-t2194-t2195+t2199-t2203-t2215+t2219-t2222-t2223+t2239+t2240-t2256-t2257+t2555+t2556+t2572+t2583-t2605-t2606+t2612+t2613-t2618-t2619+t2651+t2652;
et658 = t18.*t19.*t20.*t50.*t202.*(-3.566935413776081e-21);
et659 = t24.*t25.*t26.*t50.*t202.*(-3.992732227073824e-24);
et660 = t18.*t19.*t26.*t27.*t50.*t202.*(-3.509445006623964e-21);
et661 = t21.*t24.*t25.*t26.*t50.*t202.*(-7.696420262413979e-21);
et662 = t707+t708-t721-t722-t749+t762+t768-t777-t792-t793-t801-t802-t808+t813-t819+t821-t1629+t1637-t1640-t1641-t1659-t1661+t1666+t1667+t1683+t1692+t1705-t1712+t1758+t1759+t1775+t1776+t1973+t1993+t1994+t2023+t2053+t2060-t2089-t2090+t2098+t2099-t8.*t9.*t15.*t50.*t189.*3.670836568391568e-22;
et663 = t10.*t13.*t14.*t50.*t189.*(-3.279367663374749e-19)-t8.*t9.*t11.*t15.*t50.*t189.*7.075931802640439e-19;
et664 = t8.*t11.*t14.*t15.*t50.*t189.*(-1.190170786299927e-18)-t9.*t11.*t13.*t15.*t50.*t189.*1.190170786299927e-18;
et665 = t13.*t14.*t15.*t16.*t50.*t189.*(-3.226512155691387e-19);
et666 = -t5343-t5565-t5813-t5851+t5876-t5880+t6066+t6095+t6174+t6223-t6425+t6460-t6469+t6482+t6702+t6708-t6962-t6964+t6995+t7114-t7159-t7161+t7420;
et667 = (t5278.*(t350+t366-t1205+t1210-t1217-t1218-t2147+t2152+t2154+t2155-t3405-t3409-t3420-t3739+t3746+t26.*t50.*t202.*(t46-t47).*8.687615694748404e-39))./2.0;
et668 = (t3500.*(t4573.*(t2813-t2835+t12.*(t1456-t2355).*1.02e-6+t17.*(t1456-t2355).*9.0e-8)+t4577.*(-t2804+t2838+t3109+t17.*(t1456-t2355).*9.3e-7)+t3133.*(t3242-t3554)))./2.0+(t5026.*(et662+et663+et664+et665))./2.0+(t6916.*(t1861-t3221))./2.0;
et669 = (t6647.*(t3359-t3670+t22.*(t3242-t3554).*1.33637554986e-4+t28.*(t3242-t3554).*7.26350557185e-5))./2.0+(t3502.*(t3993+t4240-t4332+t4464+t4031.*(t2801-t2850)+t4026.*(t335-t1539-t2831+t2851)))./2.0;
et670 = (t5949.*(t4843+t5108+t2307.*(t642+t643-t667+t674+t1587+t1606+t1608+t1609+t2295+t2671+t2683+t2684-t2695+t3279+t3297-t3303+t3597+t3603+t3609-t3614+t4053+t4054)+t2297.*(t2292+t3290+t3524.*1.838876e-2-t3591+t3592+t3611+t16.*(t1861-t3221).*3.131399999999998e-4+t16.*t17.*(t1861-t3221).*9.99471e-3)))./2.0;
et671 = t1288+t1289+t1302+t1303-t1319-t1320+t1336-t1348+t1350+t1351-t1360+t1369-t1378+t1396-t1425+t1435-t2174+t2183-t2187+t2193-t2194-t2195+t2199-t2203-t2215+t2219-t2222-t2223+t2239+t2240-t2256-t2257+t2555+t2556+t2572+t2583-t2605-t2606+t2612+t2613-t2618-t2619+t2651+t2652;
et672 = t18.*t19.*t20.*t50.*t202.*(-3.566935413776081e-21);
et673 = t24.*t25.*t26.*t50.*t202.*(-3.992732227073824e-24);
et674 = t18.*t19.*t26.*t27.*t50.*t202.*(-3.509445006623964e-21);
et675 = t21.*t24.*t25.*t26.*t50.*t202.*(-7.696420262413979e-21);
et676 = -t5430+t5493-t5496+t6086-t6112+t6149+t6151./2.0+t6156-t6192+t6194-t6231+t6237+t6283+t6580+t6594+t6611+t6613-t6645-t6648-t6705-t6742+t6744-t7118-t7125+t7170+t7176-t7326+t7328+t7410+(t4950.*(et671+et672+et673+et674+et675))./2.0+(t7092.*(t1477-t2502))./2.0;
et677 = (t3055.*(t3131+t3132+t3171+t3446-t4281-t4282-t4301+t4303-t4308+t4310-t4583-t4594+t4623+t4639+t2388.*(t1456-t2355).*4.0e-8+(t3543.*(t1861-t3221))./1.0e+8+(t3500.*(t1896-t3239))./1.0e+8-t11.*t2297.*t2363.*2.4e-7))./2.0;
et678 = (t2363.*(t3157+t3158+t3386-t4299-t4300-t4562+t4567+t3543.*(t1861-t3221).*6.2e-7+t3500.*(t1896-t3239).*6.2e-7-(t11.*(t1861-t3221).*(t1896-t3239))./1.0e+8-(t11.*t2297.*t2363)./1.0e+8-(t11.*t3502.*t3547)./1.0e+8))./2.0+(t5859.*(t4927+t5198-t5762-t6392))./2.0;
et679 = (t21.*t2363.*(-t3434+t4606+t3980.*(t1896-t3239).*1.02e-6))./2.0;
et680 = t1288+t1289+t1302+t1303-t1319-t1320+t1336-t1348+t1350+t1351-t1360+t1369-t1378+t1396-t1425+t1435-t2174+t2183-t2187+t2193-t2194-t2195+t2199-t2203-t2215+t2219-t2222-t2223+t2239+t2240-t2256-t2257+t2555+t2556+t2572+t2583-t2605-t2606+t2612+t2613-t2618-t2619+t2651+t2652;
et681 = t18.*t19.*t20.*t50.*t202.*(-3.566935413776081e-21);
et682 = t24.*t25.*t26.*t50.*t202.*(-3.992732227073824e-24);
et683 = t18.*t19.*t26.*t27.*t50.*t202.*(-3.509445006623964e-21);
et684 = t21.*t24.*t25.*t26.*t50.*t202.*(-7.696420262413979e-21);
et685 = -t5430+t5493-t5496+t6086-t6112+t6149+t6151./2.0+t6156-t6192+t6194-t6233+t6239+t6283+t6580+t6594+t6611+t6613-t6646-t6649-t6705-t6742+t6744-t7118-t7125+t7170+t7176-t7326+t7328+t7412+(t4950.*(et680+et681+et682+et683+et684))./2.0+(t7092.*(t1477-t2502))./2.0;
et686 = (t3055.*(t3131+t3132+t3171+t3446-t4281-t4282-t4301+t4303-t4308+t4310-t4583-t4594+t4623+t4639+t2388.*(t1456-t2355).*4.0e-8+(t3543.*(t1861-t3221))./1.0e+8+(t3500.*(t1896-t3239))./1.0e+8-t11.*t2297.*t2363.*2.4e-7))./2.0;
et687 = (t2363.*(t3157+t3158+t3386-t4299-t4300-t4562+t4567+t3543.*(t1861-t3221).*6.2e-7+t3500.*(t1896-t3239).*6.2e-7-(t11.*(t1861-t3221).*(t1896-t3239))./1.0e+8-(t11.*t2297.*t2363)./1.0e+8-(t11.*t3502.*t3547)./1.0e+8))./2.0+(t5860.*(t4927+t5198-t5762-t6392))./2.0;
et688 = (t21.*t2363.*(-t3434+t4606+t3980.*(t1896-t3239).*1.02e-6))./2.0;
et689 = t5437+t5464+t7228+t7231+t7253+t7254+t7453+t7498+t7502+t7546+t7718-t7766+t7768+t7769+t7833+(t3047.*(t5490+t6190-t6193-t6609-t6610+t5405.*(t1477-t2502)))./2.0+(t3991.*(t5713+t5714-t6443-t6719-t6722+t6102.*(t3563-t4051)))./2.0+(t3980.*(t5691+t6884-t6886-t7353-t7354+t6065.*(t3242-t3554)))./2.0+(t7426.*(t1456-t2355))./2.0+(t3991.*(t6263-t6887+t6888-t7355+t7307.*(t3563-t4051)+t21.*t3547.*(-t3434+t4606+t3980.*(t1896-t3239).*1.02e-6)))./2.0;
et690 = (t11.*t7523.*(t1861-t3221))./2.0;
et691 = t29.*t7880-t30.*t7881+t34.*(et553+et554)+t31.*(et594+et595+et596+et597+et598+et599+et600+et601+et602+et603+et604+et605+et606+et607+et608+et609)+t33.*(et615+et616+et617+et618+et619+et620+et621+et622+et623)+t32.*(et633+et634+et635+et636+et637+et638)+dq3.*dq6.*(t5399+t5545+t6250+t6261+t7000+t7001+t7582-t7645+t7744+t7745+t7870+t7872+t7942+t7952-t7954+(t7631.*(-t1901+t3122+t3277))./2.0)+dq1.*dq2.*(t3126+t3193+t3194+t3209+t3463+t3480+t3490+t3588+t3820+t3821+t3891+t3895+t4205+t4337+t4342+t4413+t4417-t5589-t5593+t5718+t5721-t5907-t5914+t6007+t6009+t6452+t6502+t6504-t6672+t6687+t6690-t7255+t7257+t7261-t7263+(t5858.*(et639+et640))./2.0+(t5594.*(et641+et642+et643+et644))./2.0)-dq3.*dq5.*(et651+et652+et653+et654+et655+et656);
et692 = dq1.*dq6.*(t5819+t6362-t6635+t6639+t6640+t6643-t6692-t6694+t7037+t7038+t7156+t7370+t7373+(t6682.*(-t4045+t4049+t12.*(t1861-t3221).*1.838876e-2+t17.*(t1861-t3221).*9.99471e-3))./2.0);
et693 = dq2.*dq6.*(t5819+t6362-t6635+t6639+t6640+t6643-t6693-t6695+t7037+t7038+t7156+t7370+t7373+(t6682.*(-t4045+t4049+t12.*(t1861-t3221).*1.838876e-2+t17.*(t1861-t3221).*9.99471e-3))./2.0);
et694 = dq3.*dq6.*(t5404+t5544+t6228+t6230+t6971+t6975+t7429+t7466-t7529+t7564+t7568+t7721+t7765+t7778+t7780+t7821+t7822+t7878-t7917-t7918+(t7470.*(t11.*((t237.*(t42-t43))./9.007199254740992e+15+t15.*(-t1881+t3121+t3276))+t16.*(-t1901+t3122+t3277)))./2.0)-dq3.*dq5.*(t4559+t4713+t5283+t5381+t5460+t5499+t5570+t5586+t5954+t5955+t6172+t6178+t6564+t6565+t6983+t6989+t7059+t7066+t7345+t7347+t7440+t7451+t7511+t7512+t7550+t7552+t7672+t7674+t7683+t7684+t7695+t7696+t7762+t7763+t7841+t7842+t7849+t7850+t7901+t7905+t7920+t7921+t7927+t7929);
et695 = dq3.*dq4.*(t4923+t4924-t5678+t5684+t6918-t6919+t6920-t6987+t7164+t7408+t7427-t7444-t7496+t7668+t7669+t7670-t7737-t7789+t7790+t7868+t7876+t7895-t7896-t7910-t7911+(t5783.*(et657+et658+et659+et660+et661))./2.0+(t6650.*(t5034-t5280-t6302+t7166))./2.0+(t7083.*(-t1901+t3122+t3277))./2.0+(t7433.*(-t1901+t3122+t3277))./2.0+(t7470.*(-t1901+t3122+t3277))./2.0).*2.0+dq4.*dq6.*(t5548+t5550+t7219+t7220+t7221+t7222+t7699+t7732+t7734).*2.0-dq1.*dq6.*t7959-dq2.*dq6.*t7960-dq1.*dq2.*t7974-dq1.*dq5.*t7977+dq1.*dq3.*t7983+dq2.*dq3.*t7984+dq1.*dq3.*t7987+dq2.*dq3.*t7988+dq2.*dq5.*(et666+et667+et668+et669+et670);
et696 = dq4.*dq5.*(t4468+t4644+t5436+t5452+t6622+t6623+t6745+t6751+t7215+t7216+t7217+t7218+t7639+t7690+t7691+t7707+t7751+t7752).*-2.0-dq5.*dq6.*(t5456+t5457+t7237+t7242+t7246+t7250+t7584+t7633+t7635+t7701+t7740+t7741+t7854+t7859+t7864+t7866+t7885+t7887)-dq1.*dq5.*(et676+et677+et678+et679)-dq2.*dq5.*(et685+et686+et687+et688)+dq5.*dq6.*(et689+et690);
et697 = -t7387+t7553+t6058.*(t1005+t20.*(t1941-t3315+t39.*t1022.*(t855-t878).*2.196325630278387e-1))+t6681.*(t4165+t27.*(t1959-t3313+t38.*t1022.*(t855-t878).*2.196325630278387e-1))+t7292.*(t1896-t3239);
et698 = t4874.*(t3435-t3448+t4615+t4619+t3976.*(t1896-t3239).*5.7e-7+t3980.*(t1896-t3239).*4.0e-8);
et699 = t6413+t7401+t4880.*(t4795+t4801+t4808+t3976.*(t2694-t2701+t3036-t3043).*5.7e-7)+t4031.*(t5287+t5291-t5328+t5333+t5337-t5340+t4835.*(t2694-t2701+t3036-t3043).*5.7e-7+t4838.*(t2694-t2701+t3036-t3043).*4.0e-8);
et700 = t4026.*(-t5202+t5286+t5297+t5331-t5332-t5336+t5341+(t4920.*(t1861-t3221))./1.0e+8+(t3934.*(t951+t10.*(-t1881+t3121+t3276)))./1.0e+8+(t4118.*(t2694-t2701+t3036-t3043))./1.0e+8+t4835.*(t2694-t2701+t3036-t3043).*4.0e-8+t4838.*(t2694-t2701+t3036-t3043).*2.4e-7);
et701 = t4872.*(-t4494-t4495+t4799+t4823+t3976.*(t2694-t2701+t3036-t3043).*4.0e-8+t3980.*(t2694-t2701+t3036-t3043).*2.4e-7);
et702 = -t2306-t2317+t3145+t3148+t35.*t941.*t948.*(t850-t874).*3.775747223193135e-1;
et703 = t36.*t941.*t948.*(t850-t874).*2.244797987218524e-1;
et704 = -t2306-t2317+t3145+t3148+t35.*t941.*t948.*(t850-t874).*3.775747223193135e-1;
et705 = t36.*t941.*t948.*(t850-t874).*2.244797987218524e-1;
et706 = t5080-t7199+t4853.*(t1005+t20.*(t1941-t3315+t39.*t1022.*(t855-t878).*2.196325630278387e-1)).*7.26735e-3;
et707 = t2419.*(t684+t685-t710+t724+t1686-t1690+t1700+t1701+t2371+t2698+t2707-t2716+t2719+t3329-t3337-t3351-t3641+t3643+t3655-t3659+t4114+t4115).*7.26735e-3;
et708 = -t2306-t2317+t3145+t3148+t35.*t941.*t948.*(t850-t874).*3.775747223193135e-1;
et709 = t36.*t941.*t948.*(t850-t874).*2.244797987218524e-1;
et710 = t4722+t4741+t5361+t5363+t5535+t5536+t5538+t5539+t5730+t5731+t5734+t5735+t7736+t7738+t7809+t7810-((t2674-t2676+t3022-t3027).*(et697+et698))./2.0+(t3502.*(et699+et700+et701))./2.0-(t4118.*(t6979+t4019.*(t4795+t4801+t4808+t3976.*(t2694-t2701+t3036-t3043).*5.7e-7)+t6159.*(t1896-t3239)))./2.0+(t2338.*t7461)./2.0+(t2297.*t7924)./2.0-(t2297.*t7938)./2.0+(t3502.*t7940)./2.0-(t4118.*t7544)./2.0+(t3910.*t7926)./2.0-(t4879.*t7523)./2.0;
et711 = ((t1861-t3221).*(t7101+t7402+t7458+t7658-t6159.*(t1005+t20.*(t1941-t3315+t39.*t1022.*(t855-t878).*2.196325630278387e-1))-t4874.*(t4795+t4801+t4808+t3976.*(t2694-t2701+t3036-t3043).*5.7e-7)))./2.0;
et712 = (t2338.*(-t6196+t6428+t3055.*(-t4494-t4495+t4799+t4823+t3976.*(t2694-t2701+t3036-t3043).*4.0e-8+t3980.*(t2694-t2701+t3036-t3043).*2.4e-7)))./2.0-(t7939.*(t1861-t3221))./2.0-(t7548.*(t951+t10.*(-t1881+t3121+t3276)))./2.0;
et713 = t4879.*(t6872+t6058.*(t1896-t3239)+t4019.*(t3435-t3448+t4615+t4619+t3976.*(t1896-t3239).*5.7e-7+t3980.*(t1896-t3239).*4.0e-8)).*(-1.0./2.0);
et714 = (t6137-t6873+t4031.*(t3435-t3448+t4615+t4619+t3976.*(t1896-t3239).*5.7e-7+t3980.*(t1896-t3239).*4.0e-8)).*(et702+et703).*(-1.0./2.0)-(t7925.*(t2674-t2676+t3022-t3027))./2.0;
et715 = (t3910.*(t6251-t6997-t7310+t7388+t7554+t4880.*(t3435-t3448+t4615+t4619+t3976.*(t1896-t3239).*5.7e-7+t3980.*(t1896-t3239).*4.0e-8)))./2.0-(t7524.*(et704+et705))./2.0;
et716 = (t951+t10.*(-t1881+t3121+t3276)).*(t6287+t4031.*(t4795+t4801+t4808+t3976.*(t2694-t2701+t3036-t3043).*5.7e-7)+t4026.*(-t4494-t4495+t4799+t4823+t3976.*(t2694-t2701+t3036-t3043).*4.0e-8+t3980.*(t2694-t2701+t3036-t3043).*2.4e-7)).*(-1.0./2.0);
et717 = ((et706+et707).*(t2674-t2676+t3022-t3027).*(t1488+t1874+t2519+t2740+t2747+t3096+t3097))./2.0+(t4346.*(t4853.*(t1896-t3239).*7.26735e-3+t2363.*(t684+t685-t710+t724+t1686-t1690+t1700+t1701+t2371+t2698+t2707-t2716+t2719+t3329-t3337-t3351-t3641+t3643+t3655-t3659+t4114+t4115).*7.26735e-3).*(t2674-t2676+t3022-t3027))./2.0;
et718 = t4352.*(t4814.*(t1861-t3221)+t2297.*(t642+t643-t667+t674+t1587+t1606+t1608+t1609+t2295+t2671+t2683+t2684-t2695+t3279+t3297-t3303+t3597+t3603+t3609-t3614+t4053+t4054)).*(t2694-t2701+t3036-t3043).*3.633675e-3+t7479.*(t2694-t2701+t3036-t3043).*(t1513+t1879+t2598+t2820+t2834+t3117+t3118).*3.633675e-3+(t6793.*(et708+et709).*(t1488+t1874+t2519+t2740+t2747+t3096+t3097))./2.0;
et719 = t3934.*t4352.*t6711.*3.633675e-3+(t3910.*t4346.*t6793)./2.0+(t4879.*(t4853.*(t1896-t3239).*7.26735e-3+t2363.*(t684+t685-t710+t724+t1686-t1690+t1700+t1701+t2371+t2698+t2707-t2716+t2719+t3329-t3337-t3351-t3641+t3643+t3655-t3659+t4114+t4115).*7.26735e-3).*(t1488+t1874+t2519+t2740+t2747+t3096+t3097))./2.0;
et720 = t3910.*t7505.*(t1488+t1874+t2519+t2740+t2747+t3096+t3097).*(-1.0./2.0)+t3934.*t7480.*(t1513+t1879+t2598+t2820+t2834+t3117+t3118).*3.633675e-3-t4915.*t6711.*(t1513+t1879+t2598+t2820+t2834+t3117+t3118).*3.633675e-3;
et721 = t4920.*(t4814.*(t1861-t3221)+t2297.*(t642+t643-t667+t674+t1587+t1606+t1608+t1609+t2295+t2671+t2683+t2684-t2695+t3279+t3297-t3303+t3597+t3603+t3609-t3614+t4053+t4054)).*(t1513+t1879+t2598+t2820+t2834+t3117+t3118).*3.633675e-3;
et722 = t236.*t241.*t4476.*t4716.*(-2.394182569460511e-91);
et723 = t236.*t241.*t4502.*t4705.*(-2.394182569460511e-91);
et724 = t236.*t241.*t4563.*t4850.*(-2.394182569460511e-91);
et725 = t236.*t241.*t4652.*t4763.*2.394182569460511e-91;
et726 = t2363.*(t2368+t3340+t3582.*1.838876e-2-t3639+t3640+t21.*(t1896-t3239).*1.247162e-2+t27.*(t1896-t3239).*3.131399999999998e-4+t27.*t28.*(t1896-t3239).*9.99471e-3);
et727 = 7.26735e-3;
et728 = t6083+t6281-t6704+t7092.*(t1477-t2502)+t3055.*(t3131+t3132+t3171+t3446-t4281-t4282-t4301+t4303-t4308+t4310-t4583-t4594+t4623+t4639+t2388.*(t1456-t2355).*4.0e-8+(t3543.*(t1861-t3221))./1.0e+8+(t3500.*(t1896-t3239))./1.0e+8-t11.*t2297.*t2363.*2.4e-7);
et729 = t2363.*(t3157+t3158+t3386-t4299-t4300-t4562+t4567+t3543.*(t1861-t3221).*6.2e-7+t3500.*(t1896-t3239).*6.2e-7-(t11.*(t1861-t3221).*(t1896-t3239))./1.0e+8-(t11.*t2297.*t2363)./1.0e+8-(t11.*t3502.*t3547)./1.0e+8);
et730 = t4468+t4644+t5436+t5452+t6622+t6623+t6745+t6751+t7215+t7216+t7217+t7218+t7639+t7690+t7691+t7707+t7751+t7752-(t3216.*(t5691+t6884-t6886-t7353-t7354+t6065.*(t3242-t3554)))./2.0+(t2297.*(-t5453+t6371-t6616+t6617+t3395.*(t3428-t3432-t4570+t4576+t4582-t4603)+t3055.*(-t3080+t4100+t11.*t3236.*(t1861-t3221).*1.02e-6)))./2.0+(t3216.*(-t6135+t6402-t7020+t7208+t7337+t21.*t6681.*(t1896-t3239)))./2.0;
et731 = (t3502.*(t5411-t5563+t6762-t6765+t4604.*(t3428-t3432-t4570+t4576+t4582-t4603)+t6244.*(t3563-t4051)))./2.0+(t6031.*(t4853.*(t1896-t3239).*7.26735e-3+t2363.*(t684+t685-t710+t724+t1686-t1690+t1700+t1701+t2371+t2698+t2707-t2716+t2719+t3329-t3337-t3351-t3641+t3643+t3655-t3659+t4114+t4115).*7.26735e-3))./2.0+(t2307.*t7407)./2.0+(t2307.*t7426)./2.0+(t2297.*t7697)./2.0-(t3500.*t7432)./2.0;
et732 = (t3503.*t7433)./2.0-(t3500.*t7469)./2.0+(t3503.*t7470)./2.0+(t3217.*t7838)./2.0-(t3502.*t7716)./2.0+(t6060.*t6711)./2.0+(t6032.*t6793)./2.0+(t6059.*(t4814.*(t1861-t3221)+t2297.*(t642+t643-t667+t674+t1587+t1606+t1608+t1609+t2295+t2671+t2683+t2684-t2695+t3279+t3297-t3303+t3597+t3603+t3609-t3614+t4053+t4054)))./2.0+(t7715.*(t1861-t3221))./2.0-(t7748.*(t1861-t3221))./2.0-(t3217.*(t6263-t6887+t6888-t7355+t7307.*(t3563-t4051)+t21.*t3547.*(-t3434+t4606+t3980.*(t1896-t3239).*1.02e-6)))./2.0;
et733 = (t6682.*(t4843+t5108+t2307.*(t642+t643-t667+t674+t1587+t1606+t1608+t1609+t2295+t2671+t2683+t2684-t2695+t3279+t3297-t3303+t3597+t3603+t3609-t3614+t4053+t4054)+t2297.*(t2292+t3290+t3524.*1.838876e-2-t3591+t3592+t3611+t16.*(t1861-t3221).*3.131399999999998e-4+t16.*t17.*(t1861-t3221).*9.99471e-3)))./2.0-(t6689.*(t4844+t5119-t5723-t6364))./2.0;
et734 = t6650.*(t4927+t5198-t5762-t6392).*(-1.0./2.0)+(t6647.*(t4925+t5194+et726.*et727+t2388.*(t684+t685-t710+t724+t1686-t1690+t1700+t1701+t2371+t2698+t2707-t2716+t2719+t3329-t3337-t3351-t3641+t3643+t3655-t3659+t4114+t4115).*7.26735e-3))./2.0+t50.*t189.*(et728+et729).*4.771516396025243e-17;
et735 = t50.*t189.*t7831.*(-4.771516396025243e-17);
et736 = t236.*t241.*t4334.*t5025.*1.297888971568006e-110;
et737 = t236.*t241.*t4325.*t5036.*1.297888971568006e-110;
et738 = t236.*t241.*t4763.*t5037.*(-1.297888971568006e-110);
et739 = t236.*t241.*t4850.*t5027.*(-1.297888971568006e-110);
et740 = t4371.*(t1896-t3239).*7.26735e-3+t2363.*(t3328+t3344+t3642-t3658+t22.*(t3242-t3554).*1.838876e-2+t28.*(t3242-t3554).*9.99471e-3).*7.26735e-3;
et741 = (t4814.*(t1861-t3221)+t2297.*(t642+t643-t667+t674+t1587+t1606+t1608+t1609+t2295+t2671+t2683+t2684-t2695+t3279+t3297-t3303+t3597+t3603+t3609-t3614+t4053+t4054)).*(-1.0./2.0);
et742 = t5793+t5796+t4577.*(t4618+t4634-t12.*t2363.*t3047.*9.0e-8-t17.*t2363.*t3047.*9.3e-7+t12.*t3980.*(t1896-t3239).*9.0e-8+t17.*t3980.*(t1896-t3239).*9.3e-7);
et743 = t4573.*(t4617+t4635-t12.*t2363.*t3047.*1.02e-6-t17.*t2363.*t3047.*9.0e-8+t12.*t3980.*(t1896-t3239).*1.02e-6+t17.*t3980.*(t1896-t3239).*9.0e-8);
et744 = t22.*t6675.*(t3242-t3554)+t28.*t6674.*(t3242-t3554);
et745 = t5580+t5581+t6376-t6724-t6725;
et746 = t3395.*(t4618+t4634-t12.*t2363.*t3047.*9.0e-8-t17.*t2363.*t3047.*9.3e-7+t12.*t3980.*(t1896-t3239).*9.0e-8+t17.*t3980.*(t1896-t3239).*9.3e-7);
et747 = t6039.*(t4853.*(t1896-t3239).*7.26735e-3+t2363.*(t684+t685-t710+t724+t1686-t1690+t1700+t1701+t2371+t2698+t2707-t2716+t2719+t3329-t3337-t3351-t3641+t3643+t3655-t3659+t4114+t4115).*7.26735e-3).*(-1.0./2.0)+(t2297.*t7688)./2.0-(t3502.*t7795)./2.0-(t6064.*t6711)./2.0-(t6041.*t6793)./2.0+et740.*et741;
et748 = (t3502.*(t5669-t6476-t6478+t6875+t4026.*(t3435-t3448+t4615+t4619+t3976.*(t1896-t3239).*5.7e-7+t3980.*(t1896-t3239).*4.0e-8)))./2.0+(t7704.*(t1861-t3221))./2.0+((t1861-t3221).*(et742+et743+et744))./2.0+(t2297.*(et745+et746))./2.0;
et749 = t236.*t241.*t4763.*t4847.*2.658076613771277e-107;
et750 = t236.*t241.*t4762.*t4850.*2.658076613771277e-107;
et751 = t5080-t7199+t4853.*(t1005+t20.*(t1941-t3315+t39.*t1022.*(t855-t878).*2.196325630278387e-1)).*7.26735e-3;
et752 = t2419.*(t684+t685-t710+t724+t1686-t1690+t1700+t1701+t2371+t2698+t2707-t2716+t2719+t3329-t3337-t3351-t3641+t3643+t3655-t3659+t4114+t4115).*7.26735e-3;
et753 = t707+t708-t721-t722-t749+t762+t768-t777-t792-t793-t801-t802-t808+t813-t819+t821-t1629+t1637-t1640-t1641-t1659-t1661+t1666+t1667+t1683+t1692+t1705-t1712+t1758+t1759+t1775+t1776+t1973+t1993+t1994+t2023+t2053+t2060-t2089-t2090+t2098+t2099-t8.*t9.*t15.*t50.*t189.*3.670836568391568e-22;
et754 = t10.*t13.*t14.*t50.*t189.*(-3.279367663374749e-19)-t8.*t9.*t11.*t15.*t50.*t189.*7.075931802640439e-19;
et755 = t8.*t11.*t14.*t15.*t50.*t189.*(-1.190170786299927e-18)-t9.*t11.*t13.*t15.*t50.*t189.*1.190170786299927e-18;
et756 = t13.*t14.*t15.*t16.*t50.*t189.*(-3.226512155691387e-19);
et757 = (t4843+t5108+t2307.*(t642+t643-t667+t674+t1587+t1606+t1608+t1609+t2295+t2671+t2683+t2684-t2695+t3279+t3297-t3303+t3597+t3603+t3609-t3614+t4053+t4054)+t2297.*(t2292+t3290+t3524.*1.838876e-2-t3591+t3592+t3611+t16.*(t1861-t3221).*3.131399999999998e-4+t16.*t17.*(t1861-t3221).*9.99471e-3)).*(t2694-t2701+t3036-t3043).*(t1513+t1879+t2598+t2820+t2834+t3117+t3118);
et758 = 3.633675e-3;
et759 = -t4678+t4703-t5308+t5391-t5458+t5481-t5570-t5586-t5849+t6160+t6959+t7010+t7012-t7336+t7439+t7450+t7464-t7512+t7549+t7551+t7560-t7563+t7565+t7673-t7684+t7727+t7730+t7753+t7759+t7792+t7802+t7807+t7814+t7816+t7900+t7904+t7919-t7927+t7928+(t6647.*(et751+et752))./2.0;
et760 = (t7462.*(t4853.*(t1896-t3239).*7.26735e-3+t2363.*(t684+t685-t710+t724+t1686-t1690+t1700+t1701+t2371+t2698+t2707-t2716+t2719+t3329-t3337-t3351-t3641+t3643+t3655-t3659+t4114+t4115).*7.26735e-3))./2.0;
